simulink model "simulator_prototype_v2"  (R2021b)
(part 8 of 12)

tau_c = ft_11({dq1,dq2,dq3,dq4,dq5,dq6,t10,t1005,t1022,t1089,t11,t1104,t1105,t1108,t1115,t1121,t1158,t1159,t1196,t12,t1205,t1207,t1208,t1210,t1212,t1217,t1218,t1221,t123,t1230,t1235,t1237,t1238,t1288,t1289,t13,t1302,t1303,t1319,t1320,t1336,t1348,t1350,t1351,t1360,t1369,t1378,t1396,t14,t140,t1425,t1435,t1456,t1477,t1488,t15,t1513,t1539,t1544,t1547,t1548,t1553,t1554,t1559,t1564,t1576,t1577,t1578,t1579,t1584,t1585,t1586,t1587,t1591,t1599,t16,t1600,t1602,t1604,t1605,t1606,t1607,t1608,t1609,t1613,t1614,t1615,t1616,t1626,t1627,t1628,t1629,t1631,t1637,t1640,t1641,t1648,t1649,t1659,t1660,t1661,t1666,t1667,t1683,t1686,t1690,t1692,t17,t1700,t1701,t1704,t1705,t1712,t1717,t1738,t1741,t1742,t1750,t1752,t1753,t1754,t1758,t1759,t1775,t1776,t18,t1861,t1874,t1879,t188,t1881,t189,t1896,t19,t1901,t1941,t1959,t1973,t1993,t1994,t20,t201,t202,t2023,t2053,t2060,t2089,t2090,t2098,t2099,t21,t2117,t2120,t2122,t2123,t2125,t2137,t2139,t2140,t2142,t2147,t2149,t2150,t2151,t2152,t2154,t2155,t2159,t2164,t2165,t2166,t2167,t2168,t2174,t2183,t2187,t2193,t2194,t2195,t2199,t22,t2203,t2215,t2219,t2222,t2223,t2239,t2240,t2256,t2257,t2291,t2292,t2293,t2294,t2295,t2297,t2298,t2299,t2301,t2302,t2303,t2304,t2306,t2307,t2308,t2311,t2317,t2320,t2323,t2325,t2326,t2329,t2337,t2338,t2339,t2341,t2343,t2344,t2352,t2353,t2355,t2359,t236,t2360,t2361,t2362,t2363,t2364,t2365,t2366,t2367,t2368,t2369,t237,t2370,t2371,t2378,t2379,t238,t2380,t2384,t2388,t2389,t2391,t2394,t2395,t2397,t2398,t2399,t24,t2400,t2401,t2403,t2404,t2405,t241,t2414,t2419,t2421,t2423,t2438,t2448,t2449,t2461,t2471,t2472,t2492,t2493,t2494,t25,t2502,t2510,t2519,t2527,t2530,t2534,t2555,t2556,t2572,t2575,t2583,t2598,t26,t2605,t2606,t2612,t2613,t2618,t2619,t262,t2638,t264,t2651,t2652,t2670,t2671,t2673,t2674,t2675,t2676,t2678,t2680,t2683,t2684,t2685,t2686,t2687,t2689,t2690,t2692,t2693,t2694,t2695,t2696,t2697,t2698,t27,t2700,t2701,t2704,t2705,t2707,t2708,t2709,t2711,t2712,t2713,t2715,t2716,t2717,t2719,t2720,t2721,t2736,t2740,t2744,t2745,t2747,t2748,t2749,t2750,t2754,t2759,t2773,t2774,t2777,t2778,t2779,t2781,t2785,t2786,t2787,t2788,t2797,t28,t2801,t2804,t2813,t2814,t2820,t2831,t2834,t2835,t2838,t2850,t2851,t29,t2937,t2942,t2945,t2946,t2950,t2951,t2953,t2954,t2955,t2956,t2957,t2965,t2966,t2975,t2978,t2979,t2984,t2987,t2990,t2991,t2993,t2994,t2998,t30,t3003,t3004,t3008,t3009,t3015,t3017,t3022,t3027,t3029,t3030,t3036,t3043,t3044,t3045,t3047,t3049,t3050,t3051,t3054,t3055,t3057,t3058,t3063,t3064,t3066,t3067,t3068,t3072,t3073,t3079,t3080,t3081,t3085,t3086,t3087,t3088,t3096,t3097,t31,t3109,t3117,t3118,t3121,t3122,t3126,t3129,t313,t3130,t3131,t3132,t3133,t3134,t3135,t3136,t314,t3140,t3141,t3142,t3143,t3145,t3148,t3150,t3153,t3154,t3156,t3157,t3158,t3159,t3160,t3161,t3162,t3163,t3164,t3165,t3167,t3171,t3172,t3173,t3180,t3181,t3185,t3187,t3188,t3189,t3190,t3192,t3193,t3194,t3195,t3196,t3198,t3199,t32,t3200,t3201,t3202,t3203,t3205,t3206,t3208,t3209,t321,t3211,t3213,t3216,t3217,t3219,t3221,t3225,t3230,t3231,t3232,t3233,t3234,t3235,t3236,t3237,t3238,t3239,t3242,t3252,t3253,t3254,t3256,t3257,t3259,t326,t3260,t3261,t3263,t3265,t3266,t3267,t3268,t3269,t3270,t3271,t3272,t3273,t3276,t3277,t3278,t3279,t328,t3282,t3283,t3284,t3287,t3288,t329,t3290,t3291,t3294,t3297,t3298,t3299,t33,t3300,t3302,t3303,t3304,t3305,t3307,t3309,t331,t3310,t3312,t3313,t3314,t3315,t3316,t3318,t332,t3322,t3324,t3326,t3328,t3329,t333,t3332,t3333,t3334,t3335,t3336,t3337,t3338,t3340,t3341,t3343,t3344,t3345,t3346,t3347,t3348,t335,t3350,t3351,t3352,t3353,t3354,t3355,t3357,t3358,t3359,t3361,t3363,t3364,t3365,t3367,t3368,t3369,t3370,t3377,t3379,t338,t3383,t3386,t3387,t3389,t339,t3392,t3394,t3395,t3396,t3399,t34,t3402,t3405,t3409,t3415,t3416,t3419,t3420,t3421,t3423,t3426,t3428,t3430,t3431,t3432,t3433,t3434,t3435,t3438,t3439,t3440,t3441,t3443,t3444,t3445,t3446,t3447,t3448,t3449,t3451,t3452,t3453,t3454,t3455,t3456,t3457,t3458,t346,t3460,t3461,t3462,t3463,t3465,t3467,t3468,t3469,t3470,t3471,t3474,t3480,t3482,t3483,t3488,t3489,t3490,t3492,t3495,t3496,t3498,t3499,t35,t350,t3500,t3502,t3503,t3508,t351,t3510,t3512,t3517,t3519,t3522,t3524,t3527,t3528,t3529,t3531,t3532,t3534,t3537,t354,t3541,t3543,t3545,t3546,t3547,t3549,t3550,t3551,t3552,t3554,t3558,t356,t3561,t3562,t3563,t3566,t3568,t3569,t3577,t3578,t358,t3580,t3581,t3582,t3583,t3584,t3586,t3588,t3589,t359,t3590,t3591,t3592,t3593,t3594,t3597,t3598,t3599,t36,t360,t3600,t3601,t3602,t3603,t3605,t3606,t3607,t3608,t3609,t3610,t3611,t3612,t3614,t3616,t3617,t3618,t3619,t362,t3621,t3624,t3626,t3628,t363,t3630,t3631,t3632,t3633,t3634,t3635,t3636,t3637,t3638,t3639,t364,t3640,t3641,t3642,t3643,t3644,t3645,t3646,t3647,t3648,t3649,t365,t3650,t3651,t3652,t3653,t3654,t3655,t3656,t3657,t3658,t3659,t366,t3660,t3661,t3662,t3664,t3666,t3667,t3668,t3669,t3670,t3671,t3672,t3673,t3674,t3675,t3677,t3678,t3679,t3680,t3681,t3683,t3684,t3688,t3689,t3690,t3692,t3693,t3695,t3696,t3697,t3699,t3700,t3701,t3702,t3703,t3704,t3705,t3706,t3707,t3708,t3709,t371,t3710,t3711,t3712,t3713,t3716,t3717,t3719,t372,t3721,t3722,t3723,t3726,t3728,t3729,t3731,t3732,t3734,t3735,t3736,t3737,t3738,t3739,t3741,t3743,t3746,t3747,t3749,t3751,t3752,t3753,t3754,t3755,t3759,t3760,t3764,t3765,t3766,t3770,t3771,t3772,t3774,t3775,t3777,t3779,t378,t3781,t3782,t3783,t3784,t3785,t3786,t3788,t3789,t3790,t3791,t3792,t3793,t3794,t3795,t3796,t3797,t3798,t38,t380,t3800,t3801,t3802,t3804,t3805,t3808,t3809,t3810,t3814,t3815,t3817,t3818,t3819,t382,t3820,t3821,t3823,t3824,t3826,t3827,t3828,t3830,t3832,t3833,t3834,t3835,t3840,t3843,t3844,t3845,t3846,t3848,t3850,t3851,t3855,t3856,t3857,t3859,t3862,t3863,t3866,t3867,t387,t3870,t3873,t3874,t3876,t3877,t3878,t3879,t3880,t3885,t3888,t3889,t3890,t3891,t3893,t3895,t3896,t3897,t3898,t39,t3900,t3901,t3902,t3903,t3906,t3908,t3909,t3910,t3913,t3915,t3919,t3924,t3925,t3926,t3931,t3934,t3937,t3939,t3941,t3943,t3949,t3951,t3953,t3954,t3957,t3958,t3959,t3961,t3966,t3967,t3968,t3970,t3971,t3973,t3974,t3975,t3976,t3977,t3979,t3980,t3983,t3985,t3987,t3988,t3991,t3992,t3993,t3996,t3997,t3998,t3999,t4001,t4002,t4008,t4010,t4011,t4012,t4014,t4015,t4016,t4017,t4018,t4019,t4026,t4030,t4031,t4032,t4035,t4038,t4039,t4041,t4045,t4046,t4047,t4048,t4049,t4050,t4059,t4060,t4063,t4064,t4065,t4066,t4071,t4086,t4090,t4091,t4092,t4096,t4097,t4098,t4099,t410,t4100,t4101,t4103,t4105,t4107,t4108,t4109,t4110,t4111,t4112,t4116,t4117,t4118,t4121,t4122,t4144,t4146,t4147,t4149,t4151,t4153,t4154,t4156,t4157,t4158,t4159,t4160,t4163,t4165,t4171,t4172,t4179,t4180,t4187,t4188,t4189,t4190,t4193,t4195,t4198,t42,t4200,t4201,t4204,t4205,t4207,t4208,t4210,t4213,t4215,t4218,t4219,t4224,t4229,t4230,t4236,t4237,t4240,t4241,t4243,t4244,t4246,t4248,t4249,t4258,t4260,t4261,t4263,t4265,t4270,t4272,t4273,t4274,t4275,t4276,t4277,t4278,t4279,t4280,t4281,t4282,t4283,t4286,t4287,t4288,t4289,t429,t4290,t4291,t4293,t4294,t4295,t4296,t4297,t4298,t4299,t43,t4300,t4301,t4303,t4304,t4305,t4306,t4307,t4308,t4310,t4311,t4312,t4313,t4314,t4318,t4319,t4320,t4322,t4323,t4324,t4325,t4326,t4330,t4331,t4332,t4333,t4334,t4337,t4339,t4341,t4342,t4343,t4344,t4345,t4346,t4347,t4352,t4354,t4355,t4356,t4358,t4359,t4361,t4362,t4371,t4372,t4373,t4374,t4375,t4376,t4403,t4404,t4405,t4406,t4407,t4409,t4413,t4415,t4416,t4417,t4420,t4422,t4423,t4426,t4427,t4428,t4429,t4430,t4431,t4432,t4434,t4435,t4436,t4438,t4439,t4440,t4441,t4443,t4448,t4449,t4455,t4456,t4457,t4458,t4459,t4461,t4462,t4464,t4465,t4466,t4467,t4468,t4470,t4476,t4479,t4482,t4485,t4486,t4487,t4488,t4489,t4491,t4492,t4493,t4494,t4495,t4496,t4497,t4498,t4499,t4500,t4501,t4502,t4504,t4510,t4515,t4517,t4518,t4520,t4522,t4523,t4529,t4532,t4533,t4534,t4537,t4541,t4542,t4544,t4545,t4546,t4548,t4549,t4550,t4551,t4553,t4554,t4559,t4561,t4562,t4563,t4564,t4565,t4567,t4570,t4571,t4573,t4574,t4576,t4577,t4578,t4579,t4580,t4583,t4584,t4585,t4588,t4589,t4591,t4593,t4594,t4595,t4596,t4598,t4599,t46,t4602,t4605,t4606,t4608,t4609,t4612,t4613,t4614,t4615,t4618,t4623,t4625,t4626,t4634,t4635,t4637,t4643,t4644,t4645,t4646,t4647,t4648,t4649,t4650,t4651,t4652,t4654,t4656,t4657,t4658,t4660,t4663,t4665,t4667,t4669,t4670,t4672,t4673,t4674,t4675,t4676,t4677,t4678,t4680,t4681,t4682,t4683,t4684,t4685,t4686,t4687,t4690,t4691,t4692,t4694,t4696,t47,t4703,t4704,t4705,t4708,t4709,t4711,t4712,t4713,t4716,t4718,t4719,t4722,t4724,t4725,t4726,t4727,t4728,t4730,t4731,t4733,t4734,t4737,t4739,t4741,t4742,t4743,t4744,t4746,t4751,t4757,t4760,t4761,t4762,t4763,t4764,t4766,t4767,t4768,t4769,t4774,t4776,t4777,t4778,t4779,t4781,t4783,t4784,t4785,t4786,t4787,t4790,t4791,t4792,t4793,t4794,t4795,t4796,t4798,t4799,t4801,t4803,t4806,t4812,t4814,t4815,t4816,t4818,t4820,t4824,t4825,t4826,t4828,t4833,t4835,t4838,t4843,t4844,t4845,t4846,t4847,t4848,t4849,t4850,t4853,t4856,t4857,t4858,t4859,t4863,t4867,t4872,t4874,t4875,t4876,t4879,t4880,t4883,t4886,t4887,t4889,t4892,t4893,t4895,t4896,t4898,t4899,t4901,t4902,t4904,t4907,t4911,t4912,t4915,t4918,t4919,t4920,t4921,t4922,t4923,t4924,t4925,t4926,t4927,t4928,t4929,t4930,t4933,t4934,t4935,t4936,t4937,t4938,t4939,t4940,t4941,t4943,t4945,t4946,t4947,t4950,t4952,t4953,t4955,t4958,t4969,t4973,t4974,t4977,t4979,t50,t5001,t5003,t5004,t5005,t5012,t5013,t5014,t5016,t5019,t5020,t5024,t5025,t5026,t5027,t5028,t5033,t5034,t5035,t5036,t5037,t5038,t5041,t5042,t5043,t5045,t5046,t5047,t5049,t5051,t5052,t5053,t5059,t5061,t5062,t5063,t5064,t5066,t5070,t5071,t5072,t5074,t5075,t5076,t5077,t5079,t5080,t5081,t5082,t5083,t5084,t5085,t5086,t5087,t5088,t5089,t5090,t5091,t5093,t5096,t5097,t5098,t5100,t5101,t5103,t5106,t5108,t5111,t5113,t5114,t5117,t5118,t5119,t5123,t5124,t5126,t5127,t5141,t5142,t5144,t5146,t5155,t5158,t5161,t5163,t5164,t5165,t5166,t5168,t5169,t5171,t5173,t5174,t5176,t5177,t5178,t5180,t5181,t5194,t5195,t5196,t5197,t5198,t5199,t5200,t5201,t5202,t5203,t5205,t5208,t5212,t5213,t5214,t5215,t5219,t5234,t5240,t5241,t5243,t5244,t5246,t5247,t5248,t5249,t5251,t5254,t5255,t5256,t5257,t5258,t5259,t5261,t5262,t5263,t5264,t5265,t5266,t5267,t5268,t5269,t5271,t5272,t5273,t5274,t5276,t5277,t5278,t5279,t5280,t5281,t5283,t5284,t5285,t5286,t5287,t5288,t5289,t5290,t5291,t5292,t5293,t5294,t5295,t5296,t5297,t5298,t5300,t5301,t5302,t5303,t5304,t5305,t5306,t5308,t5309,t5310,t5312,t5315,t5316,t5318,t5320,t5321,t5322,t5324,t5325,t5327,t5328,t5329,t5330,t5331,t5332,t5336,t5337,t5340,t5343,t5344,t5345,t5346,t5348,t5350,t5352,t5353,t5354,t5356,t5357,t5358,t5359,t5361,t5362,t5363,t5370,t5372,t5374,t5378,t5381,t5383,t5384,t5387,t5389,t5391,t5392,t5393,t5395,t5399,t5400,t5401,t5402,t5403,t5404,t5410,t5411,t5412,t5415,t5416,t5419,t5424,t5425,t5433,t5434,t5436,t5437,t5438,t5439,t5440,t5441,t5442,t5443,t5444,t5445,t5446,t5448,t5449,t5452,t5456,t5457,t5458,t5459,t5460,t5461,t5462,t5464,t5465,t5472,t5474,t5481,t5487,t5488,t5494,t5495,t5499,t5500,t5501,t5503,t5504,t5506,t5507,t5509,t5510,t5512,t5513,t5514,t5516,t5517,t5520,t5522,t5523,t5524,t5535,t5536,t5537,t5538,t5539,t5540,t5541,t5542,t5543,t5544,t5545,t5548,t5549,t5550,t5555,t5556,t5560,t5561,t5565,t5567,t5568,t5569,t5570,t5575,t5576,t5577,t5578,t5586,t5590,t5591,t5592,t5595,t5599,t56,t5602,t5604,t5605,t5607,t5608,t5609,t5611,t5612,t5620,t5624,t5627,t5653,t5658,t5660,t5662,t5677,t5678,t5684,t5698,t5699,t5705,t5719,t5721,t5722,t5730,t5731,t5734,t5735,t5737,t5738,t5739,t5741,t5742,t5744,t5757,t5758,t5759,t5760,t5761,t5768,t5775,t5777,t5779,t5781,t5782,t5783,t5784,t5788,t58,t5813,t5818,t5825,t5849,t5852,t5891,t5892,t5896,t59,t5901,t5902,t5908,t5909,t5916,t5917,t5922,t5924,t5925,t5928,t5933,t5938,t5941,t5954,t5955,t5966,t5971,t5990,t60,t6002,t6004,t6005,t6011,t6013,t6014,t6048,t6050,t6051,t6062,t6074,t6075,t6078,t6123,t6125,t6132,t6143,t6166,t6211,t6221,t6222,t6255,t6256,t6257,t6271,t628,t638,t6394,t6396,t6398,t640,t642,t643,t6442,t6482,t649,t6523,t654,t655,t656,t6564,t6565,t657,t6574,t6588,t6589,t659,t660,t6622,t6623,t665,t6651,t667,t668,t669,t67,t670,t672,t673,t674,t6745,t675,t6751,t676,t677,t68,t681,t682,t684,t685,t686,t687,t691,t6919,t692,t6920,t693,t694,t6966,t6987,t70,t7005,t702,t707,t708,t7088,t7089,t71,t710,t7138,t7148,t715,t7150,t7152,t716,t7160,t717,t7172,t718,t721,t722,t724,t725,t73,t7304,t7319,t7331,t7332,t7333,t7334,t736,t738,t740,t741,t749,t756,t76,t762,t768,t777,t792,t793,t8,t801,t802,t808,t813,t819,t821,t850,t855,t874,t878,t89,t9,t90,t91,t92,t941,t944,t948,t951,t97});
end
function tau_c = ft_11(ct)
dq1 = ct{1};
dq2 = ct{2};
dq3 = ct{3};
dq4 = ct{4};
dq5 = ct{5};
dq6 = ct{6};
t10 = ct{7};
t1005 = ct{8};
t1022 = ct{9};
t1089 = ct{10};
t11 = ct{11};
t1104 = ct{12};
t1105 = ct{13};
t1108 = ct{14};
t1115 = ct{15};
t1121 = ct{16};
t1158 = ct{17};
t1159 = ct{18};
t1196 = ct{19};
t12 = ct{20};
t1205 = ct{21};
t1207 = ct{22};
t1208 = ct{23};
t1210 = ct{24};
t1212 = ct{25};
t1217 = ct{26};
t1218 = ct{27};
t1221 = ct{28};
t123 = ct{29};
t1230 = ct{30};
t1235 = ct{31};
t1237 = ct{32};
t1238 = ct{33};
t1288 = ct{34};
t1289 = ct{35};
t13 = ct{36};
t1302 = ct{37};
t1303 = ct{38};
t1319 = ct{39};
t1320 = ct{40};
t1336 = ct{41};
t1348 = ct{42};
t1350 = ct{43};
t1351 = ct{44};
t1360 = ct{45};
t1369 = ct{46};
t1378 = ct{47};
t1396 = ct{48};
t14 = ct{49};
t140 = ct{50};
t1425 = ct{51};
t1435 = ct{52};
t1456 = ct{53};
t1477 = ct{54};
t1488 = ct{55};
t15 = ct{56};
t1513 = ct{57};
t1539 = ct{58};
t1544 = ct{59};
t1547 = ct{60};
t1548 = ct{61};
t1553 = ct{62};
t1554 = ct{63};
t1559 = ct{64};
t1564 = ct{65};
t1576 = ct{66};
t1577 = ct{67};
t1578 = ct{68};
t1579 = ct{69};
t1584 = ct{70};
t1585 = ct{71};
t1586 = ct{72};
t1587 = ct{73};
t1591 = ct{74};
t1599 = ct{75};
t16 = ct{76};
t1600 = ct{77};
t1602 = ct{78};
t1604 = ct{79};
t1605 = ct{80};
t1606 = ct{81};
t1607 = ct{82};
t1608 = ct{83};
t1609 = ct{84};
t1613 = ct{85};
t1614 = ct{86};
t1615 = ct{87};
t1616 = ct{88};
t1626 = ct{89};
t1627 = ct{90};
t1628 = ct{91};
t1629 = ct{92};
t1631 = ct{93};
t1637 = ct{94};
t1640 = ct{95};
t1641 = ct{96};
t1648 = ct{97};
t1649 = ct{98};
t1659 = ct{99};
t1660 = ct{100};
t1661 = ct{101};
t1666 = ct{102};
t1667 = ct{103};
t1683 = ct{104};
t1686 = ct{105};
t1690 = ct{106};
t1692 = ct{107};
t17 = ct{108};
t1700 = ct{109};
t1701 = ct{110};
t1704 = ct{111};
t1705 = ct{112};
t1712 = ct{113};
t1717 = ct{114};
t1738 = ct{115};
t1741 = ct{116};
t1742 = ct{117};
t1750 = ct{118};
t1752 = ct{119};
t1753 = ct{120};
t1754 = ct{121};
t1758 = ct{122};
t1759 = ct{123};
t1775 = ct{124};
t1776 = ct{125};
t18 = ct{126};
t1861 = ct{127};
t1874 = ct{128};
t1879 = ct{129};
t188 = ct{130};
t1881 = ct{131};
t189 = ct{132};
t1896 = ct{133};
t19 = ct{134};
t1901 = ct{135};
t1941 = ct{136};
t1959 = ct{137};
t1973 = ct{138};
t1993 = ct{139};
t1994 = ct{140};
t20 = ct{141};
t201 = ct{142};
t202 = ct{143};
t2023 = ct{144};
t2053 = ct{145};
t2060 = ct{146};
t2089 = ct{147};
t2090 = ct{148};
t2098 = ct{149};
t2099 = ct{150};
t21 = ct{151};
t2117 = ct{152};
t2120 = ct{153};
t2122 = ct{154};
t2123 = ct{155};
t2125 = ct{156};
t2137 = ct{157};
t2139 = ct{158};
t2140 = ct{159};
t2142 = ct{160};
t2147 = ct{161};
t2149 = ct{162};
t2150 = ct{163};
t2151 = ct{164};
t2152 = ct{165};
t2154 = ct{166};
t2155 = ct{167};
t2159 = ct{168};
t2164 = ct{169};
t2165 = ct{170};
t2166 = ct{171};
t2167 = ct{172};
t2168 = ct{173};
t2174 = ct{174};
t2183 = ct{175};
t2187 = ct{176};
t2193 = ct{177};
t2194 = ct{178};
t2195 = ct{179};
t2199 = ct{180};
t22 = ct{181};
t2203 = ct{182};
t2215 = ct{183};
t2219 = ct{184};
t2222 = ct{185};
t2223 = ct{186};
t2239 = ct{187};
t2240 = ct{188};
t2256 = ct{189};
t2257 = ct{190};
t2291 = ct{191};
t2292 = ct{192};
t2293 = ct{193};
t2294 = ct{194};
t2295 = ct{195};
t2297 = ct{196};
t2298 = ct{197};
t2299 = ct{198};
t2301 = ct{199};
t2302 = ct{200};
t2303 = ct{201};
t2304 = ct{202};
t2306 = ct{203};
t2307 = ct{204};
t2308 = ct{205};
t2311 = ct{206};
t2317 = ct{207};
t2320 = ct{208};
t2323 = ct{209};
t2325 = ct{210};
t2326 = ct{211};
t2329 = ct{212};
t2337 = ct{213};
t2338 = ct{214};
t2339 = ct{215};
t2341 = ct{216};
t2343 = ct{217};
t2344 = ct{218};
t2352 = ct{219};
t2353 = ct{220};
t2355 = ct{221};
t2359 = ct{222};
t236 = ct{223};
t2360 = ct{224};
t2361 = ct{225};
t2362 = ct{226};
t2363 = ct{227};
t2364 = ct{228};
t2365 = ct{229};
t2366 = ct{230};
t2367 = ct{231};
t2368 = ct{232};
t2369 = ct{233};
t237 = ct{234};
t2370 = ct{235};
t2371 = ct{236};
t2378 = ct{237};
t2379 = ct{238};
t238 = ct{239};
t2380 = ct{240};
t2384 = ct{241};
t2388 = ct{242};
t2389 = ct{243};
t2391 = ct{244};
t2394 = ct{245};
t2395 = ct{246};
t2397 = ct{247};
t2398 = ct{248};
t2399 = ct{249};
t24 = ct{250};
t2400 = ct{251};
t2401 = ct{252};
t2403 = ct{253};
t2404 = ct{254};
t2405 = ct{255};
t241 = ct{256};
t2414 = ct{257};
t2419 = ct{258};
t2421 = ct{259};
t2423 = ct{260};
t2438 = ct{261};
t2448 = ct{262};
t2449 = ct{263};
t2461 = ct{264};
t2471 = ct{265};
t2472 = ct{266};
t2492 = ct{267};
t2493 = ct{268};
t2494 = ct{269};
t25 = ct{270};
t2502 = ct{271};
t2510 = ct{272};
t2519 = ct{273};
t2527 = ct{274};
t2530 = ct{275};
t2534 = ct{276};
t2555 = ct{277};
t2556 = ct{278};
t2572 = ct{279};
t2575 = ct{280};
t2583 = ct{281};
t2598 = ct{282};
t26 = ct{283};
t2605 = ct{284};
t2606 = ct{285};
t2612 = ct{286};
t2613 = ct{287};
t2618 = ct{288};
t2619 = ct{289};
t262 = ct{290};
t2638 = ct{291};
t264 = ct{292};
t2651 = ct{293};
t2652 = ct{294};
t2670 = ct{295};
t2671 = ct{296};
t2673 = ct{297};
t2674 = ct{298};
t2675 = ct{299};
t2676 = ct{300};
t2678 = ct{301};
t2680 = ct{302};
t2683 = ct{303};
t2684 = ct{304};
t2685 = ct{305};
t2686 = ct{306};
t2687 = ct{307};
t2689 = ct{308};
t2690 = ct{309};
t2692 = ct{310};
t2693 = ct{311};
t2694 = ct{312};
t2695 = ct{313};
t2696 = ct{314};
t2697 = ct{315};
t2698 = ct{316};
t27 = ct{317};
t2700 = ct{318};
t2701 = ct{319};
t2704 = ct{320};
t2705 = ct{321};
t2707 = ct{322};
t2708 = ct{323};
t2709 = ct{324};
t2711 = ct{325};
t2712 = ct{326};
t2713 = ct{327};
t2715 = ct{328};
t2716 = ct{329};
t2717 = ct{330};
t2719 = ct{331};
t2720 = ct{332};
t2721 = ct{333};
t2736 = ct{334};
t2740 = ct{335};
t2744 = ct{336};
t2745 = ct{337};
t2747 = ct{338};
t2748 = ct{339};
t2749 = ct{340};
t2750 = ct{341};
t2754 = ct{342};
t2759 = ct{343};
t2773 = ct{344};
t2774 = ct{345};
t2777 = ct{346};
t2778 = ct{347};
t2779 = ct{348};
t2781 = ct{349};
t2785 = ct{350};
t2786 = ct{351};
t2787 = ct{352};
t2788 = ct{353};
t2797 = ct{354};
t28 = ct{355};
t2801 = ct{356};
t2804 = ct{357};
t2813 = ct{358};
t2814 = ct{359};
t2820 = ct{360};
t2831 = ct{361};
t2834 = ct{362};
t2835 = ct{363};
t2838 = ct{364};
t2850 = ct{365};
t2851 = ct{366};
t29 = ct{367};
t2937 = ct{368};
t2942 = ct{369};
t2945 = ct{370};
t2946 = ct{371};
t2950 = ct{372};
t2951 = ct{373};
t2953 = ct{374};
t2954 = ct{375};
t2955 = ct{376};
t2956 = ct{377};
t2957 = ct{378};
t2965 = ct{379};
t2966 = ct{380};
t2975 = ct{381};
t2978 = ct{382};
t2979 = ct{383};
t2984 = ct{384};
t2987 = ct{385};
t2990 = ct{386};
t2991 = ct{387};
t2993 = ct{388};
t2994 = ct{389};
t2998 = ct{390};
t30 = ct{391};
t3003 = ct{392};
t3004 = ct{393};
t3008 = ct{394};
t3009 = ct{395};
t3015 = ct{396};
t3017 = ct{397};
t3022 = ct{398};
t3027 = ct{399};
t3029 = ct{400};
t3030 = ct{401};
t3036 = ct{402};
t3043 = ct{403};
t3044 = ct{404};
t3045 = ct{405};
t3047 = ct{406};
t3049 = ct{407};
t3050 = ct{408};
t3051 = ct{409};
t3054 = ct{410};
t3055 = ct{411};
t3057 = ct{412};
t3058 = ct{413};
t3063 = ct{414};
t3064 = ct{415};
t3066 = ct{416};
t3067 = ct{417};
t3068 = ct{418};
t3072 = ct{419};
t3073 = ct{420};
t3079 = ct{421};
t3080 = ct{422};
t3081 = ct{423};
t3085 = ct{424};
t3086 = ct{425};
t3087 = ct{426};
t3088 = ct{427};
t3096 = ct{428};
t3097 = ct{429};
t31 = ct{430};
t3109 = ct{431};
t3117 = ct{432};
t3118 = ct{433};
t3121 = ct{434};
t3122 = ct{435};
t3126 = ct{436};
t3129 = ct{437};
t313 = ct{438};
t3130 = ct{439};
t3131 = ct{440};
t3132 = ct{441};
t3133 = ct{442};
t3134 = ct{443};
t3135 = ct{444};
t3136 = ct{445};
t314 = ct{446};
t3140 = ct{447};
t3141 = ct{448};
t3142 = ct{449};
t3143 = ct{450};
t3145 = ct{451};
t3148 = ct{452};
t3150 = ct{453};
t3153 = ct{454};
t3154 = ct{455};
t3156 = ct{456};
t3157 = ct{457};
t3158 = ct{458};
t3159 = ct{459};
t3160 = ct{460};
t3161 = ct{461};
t3162 = ct{462};
t3163 = ct{463};
t3164 = ct{464};
t3165 = ct{465};
t3167 = ct{466};
t3171 = ct{467};
t3172 = ct{468};
t3173 = ct{469};
t3180 = ct{470};
t3181 = ct{471};
t3185 = ct{472};
t3187 = ct{473};
t3188 = ct{474};
t3189 = ct{475};
t3190 = ct{476};
t3192 = ct{477};
t3193 = ct{478};
t3194 = ct{479};
t3195 = ct{480};
t3196 = ct{481};
t3198 = ct{482};
t3199 = ct{483};
t32 = ct{484};
t3200 = ct{485};
t3201 = ct{486};
t3202 = ct{487};
t3203 = ct{488};
t3205 = ct{489};
t3206 = ct{490};
t3208 = ct{491};
t3209 = ct{492};
t321 = ct{493};
t3211 = ct{494};
t3213 = ct{495};
t3216 = ct{496};
t3217 = ct{497};
t3219 = ct{498};
t3221 = ct{499};
t3225 = ct{500};
t3230 = ct{501};
t3231 = ct{502};
t3232 = ct{503};
t3233 = ct{504};
t3234 = ct{505};
t3235 = ct{506};
t3236 = ct{507};
t3237 = ct{508};
t3238 = ct{509};
t3239 = ct{510};
t3242 = ct{511};
t3252 = ct{512};
t3253 = ct{513};
t3254 = ct{514};
t3256 = ct{515};
t3257 = ct{516};
t3259 = ct{517};
t326 = ct{518};
t3260 = ct{519};
t3261 = ct{520};
t3263 = ct{521};
t3265 = ct{522};
t3266 = ct{523};
t3267 = ct{524};
t3268 = ct{525};
t3269 = ct{526};
t3270 = ct{527};
t3271 = ct{528};
t3272 = ct{529};
t3273 = ct{530};
t3276 = ct{531};
t3277 = ct{532};
t3278 = ct{533};
t3279 = ct{534};
t328 = ct{535};
t3282 = ct{536};
t3283 = ct{537};
t3284 = ct{538};
t3287 = ct{539};
t3288 = ct{540};
t329 = ct{541};
t3290 = ct{542};
t3291 = ct{543};
t3294 = ct{544};
t3297 = ct{545};
t3298 = ct{546};
t3299 = ct{547};
t33 = ct{548};
t3300 = ct{549};
t3302 = ct{550};
t3303 = ct{551};
t3304 = ct{552};
t3305 = ct{553};
t3307 = ct{554};
t3309 = ct{555};
t331 = ct{556};
t3310 = ct{557};
t3312 = ct{558};
t3313 = ct{559};
t3314 = ct{560};
t3315 = ct{561};
t3316 = ct{562};
t3318 = ct{563};
t332 = ct{564};
t3322 = ct{565};
t3324 = ct{566};
t3326 = ct{567};
t3328 = ct{568};
t3329 = ct{569};
t333 = ct{570};
t3332 = ct{571};
t3333 = ct{572};
t3334 = ct{573};
t3335 = ct{574};
t3336 = ct{575};
t3337 = ct{576};
t3338 = ct{577};
t3340 = ct{578};
t3341 = ct{579};
t3343 = ct{580};
t3344 = ct{581};
t3345 = ct{582};
t3346 = ct{583};
t3347 = ct{584};
t3348 = ct{585};
t335 = ct{586};
t3350 = ct{587};
t3351 = ct{588};
t3352 = ct{589};
t3353 = ct{590};
t3354 = ct{591};
t3355 = ct{592};
t3357 = ct{593};
t3358 = ct{594};
t3359 = ct{595};
t3361 = ct{596};
t3363 = ct{597};
t3364 = ct{598};
t3365 = ct{599};
t3367 = ct{600};
t3368 = ct{601};
t3369 = ct{602};
t3370 = ct{603};
t3377 = ct{604};
t3379 = ct{605};
t338 = ct{606};
t3383 = ct{607};
t3386 = ct{608};
t3387 = ct{609};
t3389 = ct{610};
t339 = ct{611};
t3392 = ct{612};
t3394 = ct{613};
t3395 = ct{614};
t3396 = ct{615};
t3399 = ct{616};
t34 = ct{617};
t3402 = ct{618};
t3405 = ct{619};
t3409 = ct{620};
t3415 = ct{621};
t3416 = ct{622};
t3419 = ct{623};
t3420 = ct{624};
t3421 = ct{625};
t3423 = ct{626};
t3426 = ct{627};
t3428 = ct{628};
t3430 = ct{629};
t3431 = ct{630};
t3432 = ct{631};
t3433 = ct{632};
t3434 = ct{633};
t3435 = ct{634};
t3438 = ct{635};
t3439 = ct{636};
t3440 = ct{637};
t3441 = ct{638};
t3443 = ct{639};
t3444 = ct{640};
t3445 = ct{641};
t3446 = ct{642};
t3447 = ct{643};
t3448 = ct{644};
t3449 = ct{645};
t3451 = ct{646};
t3452 = ct{647};
t3453 = ct{648};
t3454 = ct{649};
t3455 = ct{650};
t3456 = ct{651};
t3457 = ct{652};
t3458 = ct{653};
t346 = ct{654};
t3460 = ct{655};
t3461 = ct{656};
t3462 = ct{657};
t3463 = ct{658};
t3465 = ct{659};
t3467 = ct{660};
t3468 = ct{661};
t3469 = ct{662};
t3470 = ct{663};
t3471 = ct{664};
t3474 = ct{665};
t3480 = ct{666};
t3482 = ct{667};
t3483 = ct{668};
t3488 = ct{669};
t3489 = ct{670};
t3490 = ct{671};
t3492 = ct{672};
t3495 = ct{673};
t3496 = ct{674};
t3498 = ct{675};
t3499 = ct{676};
t35 = ct{677};
t350 = ct{678};
t3500 = ct{679};
t3502 = ct{680};
t3503 = ct{681};
t3508 = ct{682};
t351 = ct{683};
t3510 = ct{684};
t3512 = ct{685};
t3517 = ct{686};
t3519 = ct{687};
t3522 = ct{688};
t3524 = ct{689};
t3527 = ct{690};
t3528 = ct{691};
t3529 = ct{692};
t3531 = ct{693};
t3532 = ct{694};
t3534 = ct{695};
t3537 = ct{696};
t354 = ct{697};
t3541 = ct{698};
t3543 = ct{699};
t3545 = ct{700};
t3546 = ct{701};
t3547 = ct{702};
t3549 = ct{703};
t3550 = ct{704};
t3551 = ct{705};
t3552 = ct{706};
t3554 = ct{707};
t3558 = ct{708};
t356 = ct{709};
t3561 = ct{710};
t3562 = ct{711};
t3563 = ct{712};
t3566 = ct{713};
t3568 = ct{714};
t3569 = ct{715};
t3577 = ct{716};
t3578 = ct{717};
t358 = ct{718};
t3580 = ct{719};
t3581 = ct{720};
t3582 = ct{721};
t3583 = ct{722};
t3584 = ct{723};
t3586 = ct{724};
t3588 = ct{725};
t3589 = ct{726};
t359 = ct{727};
t3590 = ct{728};
t3591 = ct{729};
t3592 = ct{730};
t3593 = ct{731};
t3594 = ct{732};
t3597 = ct{733};
t3598 = ct{734};
t3599 = ct{735};
t36 = ct{736};
t360 = ct{737};
t3600 = ct{738};
t3601 = ct{739};
t3602 = ct{740};
t3603 = ct{741};
t3605 = ct{742};
t3606 = ct{743};
t3607 = ct{744};
t3608 = ct{745};
t3609 = ct{746};
t3610 = ct{747};
t3611 = ct{748};
t3612 = ct{749};
t3614 = ct{750};
t3616 = ct{751};
t3617 = ct{752};
t3618 = ct{753};
t3619 = ct{754};
t362 = ct{755};
t3621 = ct{756};
t3624 = ct{757};
t3626 = ct{758};
t3628 = ct{759};
t363 = ct{760};
t3630 = ct{761};
t3631 = ct{762};
t3632 = ct{763};
t3633 = ct{764};
t3634 = ct{765};
t3635 = ct{766};
t3636 = ct{767};
t3637 = ct{768};
t3638 = ct{769};
t3639 = ct{770};
t364 = ct{771};
t3640 = ct{772};
t3641 = ct{773};
t3642 = ct{774};
t3643 = ct{775};
t3644 = ct{776};
t3645 = ct{777};
t3646 = ct{778};
t3647 = ct{779};
t3648 = ct{780};
t3649 = ct{781};
t365 = ct{782};
t3650 = ct{783};
t3651 = ct{784};
t3652 = ct{785};
t3653 = ct{786};
t3654 = ct{787};
t3655 = ct{788};
t3656 = ct{789};
t3657 = ct{790};
t3658 = ct{791};
t3659 = ct{792};
t366 = ct{793};
t3660 = ct{794};
t3661 = ct{795};
t3662 = ct{796};
t3664 = ct{797};
t3666 = ct{798};
t3667 = ct{799};
t3668 = ct{800};
t3669 = ct{801};
t3670 = ct{802};
t3671 = ct{803};
t3672 = ct{804};
t3673 = ct{805};
t3674 = ct{806};
t3675 = ct{807};
t3677 = ct{808};
t3678 = ct{809};
t3679 = ct{810};
t3680 = ct{811};
t3681 = ct{812};
t3683 = ct{813};
t3684 = ct{814};
t3688 = ct{815};
t3689 = ct{816};
t3690 = ct{817};
t3692 = ct{818};
t3693 = ct{819};
t3695 = ct{820};
t3696 = ct{821};
t3697 = ct{822};
t3699 = ct{823};
t3700 = ct{824};
t3701 = ct{825};
t3702 = ct{826};
t3703 = ct{827};
t3704 = ct{828};
t3705 = ct{829};
t3706 = ct{830};
t3707 = ct{831};
t3708 = ct{832};
t3709 = ct{833};
t371 = ct{834};
t3710 = ct{835};
t3711 = ct{836};
t3712 = ct{837};
t3713 = ct{838};
t3716 = ct{839};
t3717 = ct{840};
t3719 = ct{841};
t372 = ct{842};
t3721 = ct{843};
t3722 = ct{844};
t3723 = ct{845};
t3726 = ct{846};
t3728 = ct{847};
t3729 = ct{848};
t3731 = ct{849};
t3732 = ct{850};
t3734 = ct{851};
t3735 = ct{852};
t3736 = ct{853};
t3737 = ct{854};
t3738 = ct{855};
t3739 = ct{856};
t3741 = ct{857};
t3743 = ct{858};
t3746 = ct{859};
t3747 = ct{860};
t3749 = ct{861};
t3751 = ct{862};
t3752 = ct{863};
t3753 = ct{864};
t3754 = ct{865};
t3755 = ct{866};
t3759 = ct{867};
t3760 = ct{868};
t3764 = ct{869};
t3765 = ct{870};
t3766 = ct{871};
t3770 = ct{872};
t3771 = ct{873};
t3772 = ct{874};
t3774 = ct{875};
t3775 = ct{876};
t3777 = ct{877};
t3779 = ct{878};
t378 = ct{879};
t3781 = ct{880};
t3782 = ct{881};
t3783 = ct{882};
t3784 = ct{883};
t3785 = ct{884};
t3786 = ct{885};
t3788 = ct{886};
t3789 = ct{887};
t3790 = ct{888};
t3791 = ct{889};
t3792 = ct{890};
t3793 = ct{891};
t3794 = ct{892};
t3795 = ct{893};
t3796 = ct{894};
t3797 = ct{895};
t3798 = ct{896};
t38 = ct{897};
t380 = ct{898};
t3800 = ct{899};
t3801 = ct{900};
t3802 = ct{901};
t3804 = ct{902};
t3805 = ct{903};
t3808 = ct{904};
t3809 = ct{905};
t3810 = ct{906};
t3814 = ct{907};
t3815 = ct{908};
t3817 = ct{909};
t3818 = ct{910};
t3819 = ct{911};
t382 = ct{912};
t3820 = ct{913};
t3821 = ct{914};
t3823 = ct{915};
t3824 = ct{916};
t3826 = ct{917};
t3827 = ct{918};
t3828 = ct{919};
t3830 = ct{920};
t3832 = ct{921};
t3833 = ct{922};
t3834 = ct{923};
t3835 = ct{924};
t3840 = ct{925};
t3843 = ct{926};
t3844 = ct{927};
t3845 = ct{928};
t3846 = ct{929};
t3848 = ct{930};
t3850 = ct{931};
t3851 = ct{932};
t3855 = ct{933};
t3856 = ct{934};
t3857 = ct{935};
t3859 = ct{936};
t3862 = ct{937};
t3863 = ct{938};
t3866 = ct{939};
t3867 = ct{940};
t387 = ct{941};
t3870 = ct{942};
t3873 = ct{943};
t3874 = ct{944};
t3876 = ct{945};
t3877 = ct{946};
t3878 = ct{947};
t3879 = ct{948};
t3880 = ct{949};
t3885 = ct{950};
t3888 = ct{951};
t3889 = ct{952};
t3890 = ct{953};
t3891 = ct{954};
t3893 = ct{955};
t3895 = ct{956};
t3896 = ct{957};
t3897 = ct{958};
t3898 = ct{959};
t39 = ct{960};
t3900 = ct{961};
t3901 = ct{962};
t3902 = ct{963};
t3903 = ct{964};
t3906 = ct{965};
t3908 = ct{966};
t3909 = ct{967};
t3910 = ct{968};
t3913 = ct{969};
t3915 = ct{970};
t3919 = ct{971};
t3924 = ct{972};
t3925 = ct{973};
t3926 = ct{974};
t3931 = ct{975};
t3934 = ct{976};
t3937 = ct{977};
t3939 = ct{978};
t3941 = ct{979};
t3943 = ct{980};
t3949 = ct{981};
t3951 = ct{982};
t3953 = ct{983};
t3954 = ct{984};
t3957 = ct{985};
t3958 = ct{986};
t3959 = ct{987};
t3961 = ct{988};
t3966 = ct{989};
t3967 = ct{990};
t3968 = ct{991};
t3970 = ct{992};
t3971 = ct{993};
t3973 = ct{994};
t3974 = ct{995};
t3975 = ct{996};
t3976 = ct{997};
t3977 = ct{998};
t3979 = ct{999};
t3980 = ct{1000};
t3983 = ct{1001};
t3985 = ct{1002};
t3987 = ct{1003};
t3988 = ct{1004};
t3991 = ct{1005};
t3992 = ct{1006};
t3993 = ct{1007};
t3996 = ct{1008};
t3997 = ct{1009};
t3998 = ct{1010};
t3999 = ct{1011};
t4001 = ct{1012};
t4002 = ct{1013};
t4008 = ct{1014};
t4010 = ct{1015};
t4011 = ct{1016};
t4012 = ct{1017};
t4014 = ct{1018};
t4015 = ct{1019};
t4016 = ct{1020};
t4017 = ct{1021};
t4018 = ct{1022};
t4019 = ct{1023};
t4026 = ct{1024};
t4030 = ct{1025};
t4031 = ct{1026};
t4032 = ct{1027};
t4035 = ct{1028};
t4038 = ct{1029};
t4039 = ct{1030};
t4041 = ct{1031};
t4045 = ct{1032};
t4046 = ct{1033};
t4047 = ct{1034};
t4048 = ct{1035};
t4049 = ct{1036};
t4050 = ct{1037};
t4059 = ct{1038};
t4060 = ct{1039};
t4063 = ct{1040};
t4064 = ct{1041};
t4065 = ct{1042};
t4066 = ct{1043};
t4071 = ct{1044};
t4086 = ct{1045};
t4090 = ct{1046};
t4091 = ct{1047};
t4092 = ct{1048};
t4096 = ct{1049};
t4097 = ct{1050};
t4098 = ct{1051};
t4099 = ct{1052};
t410 = ct{1053};
t4100 = ct{1054};
t4101 = ct{1055};
t4103 = ct{1056};
t4105 = ct{1057};
t4107 = ct{1058};
t4108 = ct{1059};
t4109 = ct{1060};
t4110 = ct{1061};
t4111 = ct{1062};
t4112 = ct{1063};
t4116 = ct{1064};
t4117 = ct{1065};
t4118 = ct{1066};
t4121 = ct{1067};
t4122 = ct{1068};
t4144 = ct{1069};
t4146 = ct{1070};
t4147 = ct{1071};
t4149 = ct{1072};
t4151 = ct{1073};
t4153 = ct{1074};
t4154 = ct{1075};
t4156 = ct{1076};
t4157 = ct{1077};
t4158 = ct{1078};
t4159 = ct{1079};
t4160 = ct{1080};
t4163 = ct{1081};
t4165 = ct{1082};
t4171 = ct{1083};
t4172 = ct{1084};
t4179 = ct{1085};
t4180 = ct{1086};
t4187 = ct{1087};
t4188 = ct{1088};
t4189 = ct{1089};
t4190 = ct{1090};
t4193 = ct{1091};
t4195 = ct{1092};
t4198 = ct{1093};
t42 = ct{1094};
t4200 = ct{1095};
t4201 = ct{1096};
t4204 = ct{1097};
t4205 = ct{1098};
t4207 = ct{1099};
t4208 = ct{1100};
t4210 = ct{1101};
t4213 = ct{1102};
t4215 = ct{1103};
t4218 = ct{1104};
t4219 = ct{1105};
t4224 = ct{1106};
t4229 = ct{1107};
t4230 = ct{1108};
t4236 = ct{1109};
t4237 = ct{1110};
t4240 = ct{1111};
t4241 = ct{1112};
t4243 = ct{1113};
t4244 = ct{1114};
t4246 = ct{1115};
t4248 = ct{1116};
t4249 = ct{1117};
t4258 = ct{1118};
t4260 = ct{1119};
t4261 = ct{1120};
t4263 = ct{1121};
t4265 = ct{1122};
t4270 = ct{1123};
t4272 = ct{1124};
t4273 = ct{1125};
t4274 = ct{1126};
t4275 = ct{1127};
t4276 = ct{1128};
t4277 = ct{1129};
t4278 = ct{1130};
t4279 = ct{1131};
t4280 = ct{1132};
t4281 = ct{1133};
t4282 = ct{1134};
t4283 = ct{1135};
t4286 = ct{1136};
t4287 = ct{1137};
t4288 = ct{1138};
t4289 = ct{1139};
t429 = ct{1140};
t4290 = ct{1141};
t4291 = ct{1142};
t4293 = ct{1143};
t4294 = ct{1144};
t4295 = ct{1145};
t4296 = ct{1146};
t4297 = ct{1147};
t4298 = ct{1148};
t4299 = ct{1149};
t43 = ct{1150};
t4300 = ct{1151};
t4301 = ct{1152};
t4303 = ct{1153};
t4304 = ct{1154};
t4305 = ct{1155};
t4306 = ct{1156};
t4307 = ct{1157};
t4308 = ct{1158};
t4310 = ct{1159};
t4311 = ct{1160};
t4312 = ct{1161};
t4313 = ct{1162};
t4314 = ct{1163};
t4318 = ct{1164};
t4319 = ct{1165};
t4320 = ct{1166};
t4322 = ct{1167};
t4323 = ct{1168};
t4324 = ct{1169};
t4325 = ct{1170};
t4326 = ct{1171};
t4330 = ct{1172};
t4331 = ct{1173};
t4332 = ct{1174};
t4333 = ct{1175};
t4334 = ct{1176};
t4337 = ct{1177};
t4339 = ct{1178};
t4341 = ct{1179};
t4342 = ct{1180};
t4343 = ct{1181};
t4344 = ct{1182};
t4345 = ct{1183};
t4346 = ct{1184};
t4347 = ct{1185};
t4352 = ct{1186};
t4354 = ct{1187};
t4355 = ct{1188};
t4356 = ct{1189};
t4358 = ct{1190};
t4359 = ct{1191};
t4361 = ct{1192};
t4362 = ct{1193};
t4371 = ct{1194};
t4372 = ct{1195};
t4373 = ct{1196};
t4374 = ct{1197};
t4375 = ct{1198};
t4376 = ct{1199};
t4403 = ct{1200};
t4404 = ct{1201};
t4405 = ct{1202};
t4406 = ct{1203};
t4407 = ct{1204};
t4409 = ct{1205};
t4413 = ct{1206};
t4415 = ct{1207};
t4416 = ct{1208};
t4417 = ct{1209};
t4420 = ct{1210};
t4422 = ct{1211};
t4423 = ct{1212};
t4426 = ct{1213};
t4427 = ct{1214};
t4428 = ct{1215};
t4429 = ct{1216};
t4430 = ct{1217};
t4431 = ct{1218};
t4432 = ct{1219};
t4434 = ct{1220};
t4435 = ct{1221};
t4436 = ct{1222};
t4438 = ct{1223};
t4439 = ct{1224};
t4440 = ct{1225};
t4441 = ct{1226};
t4443 = ct{1227};
t4448 = ct{1228};
t4449 = ct{1229};
t4455 = ct{1230};
t4456 = ct{1231};
t4457 = ct{1232};
t4458 = ct{1233};
t4459 = ct{1234};
t4461 = ct{1235};
t4462 = ct{1236};
t4464 = ct{1237};
t4465 = ct{1238};
t4466 = ct{1239};
t4467 = ct{1240};
t4468 = ct{1241};
t4470 = ct{1242};
t4476 = ct{1243};
t4479 = ct{1244};
t4482 = ct{1245};
t4485 = ct{1246};
t4486 = ct{1247};
t4487 = ct{1248};
t4488 = ct{1249};
t4489 = ct{1250};
t4491 = ct{1251};
t4492 = ct{1252};
t4493 = ct{1253};
t4494 = ct{1254};
t4495 = ct{1255};
t4496 = ct{1256};
t4497 = ct{1257};
t4498 = ct{1258};
t4499 = ct{1259};
t4500 = ct{1260};
t4501 = ct{1261};
t4502 = ct{1262};
t4504 = ct{1263};
t4510 = ct{1264};
t4515 = ct{1265};
t4517 = ct{1266};
t4518 = ct{1267};
t4520 = ct{1268};
t4522 = ct{1269};
t4523 = ct{1270};
t4529 = ct{1271};
t4532 = ct{1272};
t4533 = ct{1273};
t4534 = ct{1274};
t4537 = ct{1275};
t4541 = ct{1276};
t4542 = ct{1277};
t4544 = ct{1278};
t4545 = ct{1279};
t4546 = ct{1280};
t4548 = ct{1281};
t4549 = ct{1282};
t4550 = ct{1283};
t4551 = ct{1284};
t4553 = ct{1285};
t4554 = ct{1286};
t4559 = ct{1287};
t4561 = ct{1288};
t4562 = ct{1289};
t4563 = ct{1290};
t4564 = ct{1291};
t4565 = ct{1292};
t4567 = ct{1293};
t4570 = ct{1294};
t4571 = ct{1295};
t4573 = ct{1296};
t4574 = ct{1297};
t4576 = ct{1298};
t4577 = ct{1299};
t4578 = ct{1300};
t4579 = ct{1301};
t4580 = ct{1302};
t4583 = ct{1303};
t4584 = ct{1304};
t4585 = ct{1305};
t4588 = ct{1306};
t4589 = ct{1307};
t4591 = ct{1308};
t4593 = ct{1309};
t4594 = ct{1310};
t4595 = ct{1311};
t4596 = ct{1312};
t4598 = ct{1313};
t4599 = ct{1314};
t46 = ct{1315};
t4602 = ct{1316};
t4605 = ct{1317};
t4606 = ct{1318};
t4608 = ct{1319};
t4609 = ct{1320};
t4612 = ct{1321};
t4613 = ct{1322};
t4614 = ct{1323};
t4615 = ct{1324};
t4618 = ct{1325};
t4623 = ct{1326};
t4625 = ct{1327};
t4626 = ct{1328};
t4634 = ct{1329};
t4635 = ct{1330};
t4637 = ct{1331};
t4643 = ct{1332};
t4644 = ct{1333};
t4645 = ct{1334};
t4646 = ct{1335};
t4647 = ct{1336};
t4648 = ct{1337};
t4649 = ct{1338};
t4650 = ct{1339};
t4651 = ct{1340};
t4652 = ct{1341};
t4654 = ct{1342};
t4656 = ct{1343};
t4657 = ct{1344};
t4658 = ct{1345};
t4660 = ct{1346};
t4663 = ct{1347};
t4665 = ct{1348};
t4667 = ct{1349};
t4669 = ct{1350};
t4670 = ct{1351};
t4672 = ct{1352};
t4673 = ct{1353};
t4674 = ct{1354};
t4675 = ct{1355};
t4676 = ct{1356};
t4677 = ct{1357};
t4678 = ct{1358};
t4680 = ct{1359};
t4681 = ct{1360};
t4682 = ct{1361};
t4683 = ct{1362};
t4684 = ct{1363};
t4685 = ct{1364};
t4686 = ct{1365};
t4687 = ct{1366};
t4690 = ct{1367};
t4691 = ct{1368};
t4692 = ct{1369};
t4694 = ct{1370};
t4696 = ct{1371};
t47 = ct{1372};
t4703 = ct{1373};
t4704 = ct{1374};
t4705 = ct{1375};
t4708 = ct{1376};
t4709 = ct{1377};
t4711 = ct{1378};
t4712 = ct{1379};
t4713 = ct{1380};
t4716 = ct{1381};
t4718 = ct{1382};
t4719 = ct{1383};
t4722 = ct{1384};
t4724 = ct{1385};
t4725 = ct{1386};
t4726 = ct{1387};
t4727 = ct{1388};
t4728 = ct{1389};
t4730 = ct{1390};
t4731 = ct{1391};
t4733 = ct{1392};
t4734 = ct{1393};
t4737 = ct{1394};
t4739 = ct{1395};
t4741 = ct{1396};
t4742 = ct{1397};
t4743 = ct{1398};
t4744 = ct{1399};
t4746 = ct{1400};
t4751 = ct{1401};
t4757 = ct{1402};
t4760 = ct{1403};
t4761 = ct{1404};
t4762 = ct{1405};
t4763 = ct{1406};
t4764 = ct{1407};
t4766 = ct{1408};
t4767 = ct{1409};
t4768 = ct{1410};
t4769 = ct{1411};
t4774 = ct{1412};
t4776 = ct{1413};
t4777 = ct{1414};
t4778 = ct{1415};
t4779 = ct{1416};
t4781 = ct{1417};
t4783 = ct{1418};
t4784 = ct{1419};
t4785 = ct{1420};
t4786 = ct{1421};
t4787 = ct{1422};
t4790 = ct{1423};
t4791 = ct{1424};
t4792 = ct{1425};
t4793 = ct{1426};
t4794 = ct{1427};
t4795 = ct{1428};
t4796 = ct{1429};
t4798 = ct{1430};
t4799 = ct{1431};
t4801 = ct{1432};
t4803 = ct{1433};
t4806 = ct{1434};
t4812 = ct{1435};
t4814 = ct{1436};
t4815 = ct{1437};
t4816 = ct{1438};
t4818 = ct{1439};
t4820 = ct{1440};
t4824 = ct{1441};
t4825 = ct{1442};
t4826 = ct{1443};
t4828 = ct{1444};
t4833 = ct{1445};
t4835 = ct{1446};
t4838 = ct{1447};
t4843 = ct{1448};
t4844 = ct{1449};
t4845 = ct{1450};
t4846 = ct{1451};
t4847 = ct{1452};
t4848 = ct{1453};
t4849 = ct{1454};
t4850 = ct{1455};
t4853 = ct{1456};
t4856 = ct{1457};
t4857 = ct{1458};
t4858 = ct{1459};
t4859 = ct{1460};
t4863 = ct{1461};
t4867 = ct{1462};
t4872 = ct{1463};
t4874 = ct{1464};
t4875 = ct{1465};
t4876 = ct{1466};
t4879 = ct{1467};
t4880 = ct{1468};
t4883 = ct{1469};
t4886 = ct{1470};
t4887 = ct{1471};
t4889 = ct{1472};
t4892 = ct{1473};
t4893 = ct{1474};
t4895 = ct{1475};
t4896 = ct{1476};
t4898 = ct{1477};
t4899 = ct{1478};
t4901 = ct{1479};
t4902 = ct{1480};
t4904 = ct{1481};
t4907 = ct{1482};
t4911 = ct{1483};
t4912 = ct{1484};
t4915 = ct{1485};
t4918 = ct{1486};
t4919 = ct{1487};
t4920 = ct{1488};
t4921 = ct{1489};
t4922 = ct{1490};
t4923 = ct{1491};
t4924 = ct{1492};
t4925 = ct{1493};
t4926 = ct{1494};
t4927 = ct{1495};
t4928 = ct{1496};
t4929 = ct{1497};
t4930 = ct{1498};
t4933 = ct{1499};
t4934 = ct{1500};
t4935 = ct{1501};
t4936 = ct{1502};
t4937 = ct{1503};
t4938 = ct{1504};
t4939 = ct{1505};
t4940 = ct{1506};
t4941 = ct{1507};
t4943 = ct{1508};
t4945 = ct{1509};
t4946 = ct{1510};
t4947 = ct{1511};
t4950 = ct{1512};
t4952 = ct{1513};
t4953 = ct{1514};
t4955 = ct{1515};
t4958 = ct{1516};
t4969 = ct{1517};
t4973 = ct{1518};
t4974 = ct{1519};
t4977 = ct{1520};
t4979 = ct{1521};
t50 = ct{1522};
t5001 = ct{1523};
t5003 = ct{1524};
t5004 = ct{1525};
t5005 = ct{1526};
t5012 = ct{1527};
t5013 = ct{1528};
t5014 = ct{1529};
t5016 = ct{1530};
t5019 = ct{1531};
t5020 = ct{1532};
t5024 = ct{1533};
t5025 = ct{1534};
t5026 = ct{1535};
t5027 = ct{1536};
t5028 = ct{1537};
t5033 = ct{1538};
t5034 = ct{1539};
t5035 = ct{1540};
t5036 = ct{1541};
t5037 = ct{1542};
t5038 = ct{1543};
t5041 = ct{1544};
t5042 = ct{1545};
t5043 = ct{1546};
t5045 = ct{1547};
t5046 = ct{1548};
t5047 = ct{1549};
t5049 = ct{1550};
t5051 = ct{1551};
t5052 = ct{1552};
t5053 = ct{1553};
t5059 = ct{1554};
t5061 = ct{1555};
t5062 = ct{1556};
t5063 = ct{1557};
t5064 = ct{1558};
t5066 = ct{1559};
t5070 = ct{1560};
t5071 = ct{1561};
t5072 = ct{1562};
t5074 = ct{1563};
t5075 = ct{1564};
t5076 = ct{1565};
t5077 = ct{1566};
t5079 = ct{1567};
t5080 = ct{1568};
t5081 = ct{1569};
t5082 = ct{1570};
t5083 = ct{1571};
t5084 = ct{1572};
t5085 = ct{1573};
t5086 = ct{1574};
t5087 = ct{1575};
t5088 = ct{1576};
t5089 = ct{1577};
t5090 = ct{1578};
t5091 = ct{1579};
t5093 = ct{1580};
t5096 = ct{1581};
t5097 = ct{1582};
t5098 = ct{1583};
t5100 = ct{1584};
t5101 = ct{1585};
t5103 = ct{1586};
t5106 = ct{1587};
t5108 = ct{1588};
t5111 = ct{1589};
t5113 = ct{1590};
t5114 = ct{1591};
t5117 = ct{1592};
t5118 = ct{1593};
t5119 = ct{1594};
t5123 = ct{1595};
t5124 = ct{1596};
t5126 = ct{1597};
t5127 = ct{1598};
t5141 = ct{1599};
t5142 = ct{1600};
t5144 = ct{1601};
t5146 = ct{1602};
t5155 = ct{1603};
t5158 = ct{1604};
t5161 = ct{1605};
t5163 = ct{1606};
t5164 = ct{1607};
t5165 = ct{1608};
t5166 = ct{1609};
t5168 = ct{1610};
t5169 = ct{1611};
t5171 = ct{1612};
t5173 = ct{1613};
t5174 = ct{1614};
t5176 = ct{1615};
t5177 = ct{1616};
t5178 = ct{1617};
t5180 = ct{1618};
t5181 = ct{1619};
t5194 = ct{1620};
t5195 = ct{1621};
t5196 = ct{1622};
t5197 = ct{1623};
t5198 = ct{1624};
t5199 = ct{1625};
t5200 = ct{1626};
t5201 = ct{1627};
t5202 = ct{1628};
t5203 = ct{1629};
t5205 = ct{1630};
t5208 = ct{1631};
t5212 = ct{1632};
t5213 = ct{1633};
t5214 = ct{1634};
t5215 = ct{1635};
t5219 = ct{1636};
t5234 = ct{1637};
t5240 = ct{1638};
t5241 = ct{1639};
t5243 = ct{1640};
t5244 = ct{1641};
t5246 = ct{1642};
t5247 = ct{1643};
t5248 = ct{1644};
t5249 = ct{1645};
t5251 = ct{1646};
t5254 = ct{1647};
t5255 = ct{1648};
t5256 = ct{1649};
t5257 = ct{1650};
t5258 = ct{1651};
t5259 = ct{1652};
t5261 = ct{1653};
t5262 = ct{1654};
t5263 = ct{1655};
t5264 = ct{1656};
t5265 = ct{1657};
t5266 = ct{1658};
t5267 = ct{1659};
t5268 = ct{1660};
t5269 = ct{1661};
t5271 = ct{1662};
t5272 = ct{1663};
t5273 = ct{1664};
t5274 = ct{1665};
t5276 = ct{1666};
t5277 = ct{1667};
t5278 = ct{1668};
t5279 = ct{1669};
t5280 = ct{1670};
t5281 = ct{1671};
t5283 = ct{1672};
t5284 = ct{1673};
t5285 = ct{1674};
t5286 = ct{1675};
t5287 = ct{1676};
t5288 = ct{1677};
t5289 = ct{1678};
t5290 = ct{1679};
t5291 = ct{1680};
t5292 = ct{1681};
t5293 = ct{1682};
t5294 = ct{1683};
t5295 = ct{1684};
t5296 = ct{1685};
t5297 = ct{1686};
t5298 = ct{1687};
t5300 = ct{1688};
t5301 = ct{1689};
t5302 = ct{1690};
t5303 = ct{1691};
t5304 = ct{1692};
t5305 = ct{1693};
t5306 = ct{1694};
t5308 = ct{1695};
t5309 = ct{1696};
t5310 = ct{1697};
t5312 = ct{1698};
t5315 = ct{1699};
t5316 = ct{1700};
t5318 = ct{1701};
t5320 = ct{1702};
t5321 = ct{1703};
t5322 = ct{1704};
t5324 = ct{1705};
t5325 = ct{1706};
t5327 = ct{1707};
t5328 = ct{1708};
t5329 = ct{1709};
t5330 = ct{1710};
t5331 = ct{1711};
t5332 = ct{1712};
t5336 = ct{1713};
t5337 = ct{1714};
t5340 = ct{1715};
t5343 = ct{1716};
t5344 = ct{1717};
t5345 = ct{1718};
t5346 = ct{1719};
t5348 = ct{1720};
t5350 = ct{1721};
t5352 = ct{1722};
t5353 = ct{1723};
t5354 = ct{1724};
t5356 = ct{1725};
t5357 = ct{1726};
t5358 = ct{1727};
t5359 = ct{1728};
t5361 = ct{1729};
t5362 = ct{1730};
t5363 = ct{1731};
t5370 = ct{1732};
t5372 = ct{1733};
t5374 = ct{1734};
t5378 = ct{1735};
t5381 = ct{1736};
t5383 = ct{1737};
t5384 = ct{1738};
t5387 = ct{1739};
t5389 = ct{1740};
t5391 = ct{1741};
t5392 = ct{1742};
t5393 = ct{1743};
t5395 = ct{1744};
t5399 = ct{1745};
t5400 = ct{1746};
t5401 = ct{1747};
t5402 = ct{1748};
t5403 = ct{1749};
t5404 = ct{1750};
t5410 = ct{1751};
t5411 = ct{1752};
t5412 = ct{1753};
t5415 = ct{1754};
t5416 = ct{1755};
t5419 = ct{1756};
t5424 = ct{1757};
t5425 = ct{1758};
t5433 = ct{1759};
t5434 = ct{1760};
t5436 = ct{1761};
t5437 = ct{1762};
t5438 = ct{1763};
t5439 = ct{1764};
t5440 = ct{1765};
t5441 = ct{1766};
t5442 = ct{1767};
t5443 = ct{1768};
t5444 = ct{1769};
t5445 = ct{1770};
t5446 = ct{1771};
t5448 = ct{1772};
t5449 = ct{1773};
t5452 = ct{1774};
t5456 = ct{1775};
t5457 = ct{1776};
t5458 = ct{1777};
t5459 = ct{1778};
t5460 = ct{1779};
t5461 = ct{1780};
t5462 = ct{1781};
t5464 = ct{1782};
t5465 = ct{1783};
t5472 = ct{1784};
t5474 = ct{1785};
t5481 = ct{1786};
t5487 = ct{1787};
t5488 = ct{1788};
t5494 = ct{1789};
t5495 = ct{1790};
t5499 = ct{1791};
t5500 = ct{1792};
t5501 = ct{1793};
t5503 = ct{1794};
t5504 = ct{1795};
t5506 = ct{1796};
t5507 = ct{1797};
t5509 = ct{1798};
t5510 = ct{1799};
t5512 = ct{1800};
t5513 = ct{1801};
t5514 = ct{1802};
t5516 = ct{1803};
t5517 = ct{1804};
t5520 = ct{1805};
t5522 = ct{1806};
t5523 = ct{1807};
t5524 = ct{1808};
t5535 = ct{1809};
t5536 = ct{1810};
t5537 = ct{1811};
t5538 = ct{1812};
t5539 = ct{1813};
t5540 = ct{1814};
t5541 = ct{1815};
t5542 = ct{1816};
t5543 = ct{1817};
t5544 = ct{1818};
t5545 = ct{1819};
t5548 = ct{1820};
t5549 = ct{1821};
t5550 = ct{1822};
t5555 = ct{1823};
t5556 = ct{1824};
t5560 = ct{1825};
t5561 = ct{1826};
t5565 = ct{1827};
t5567 = ct{1828};
t5568 = ct{1829};
t5569 = ct{1830};
t5570 = ct{1831};
t5575 = ct{1832};
t5576 = ct{1833};
t5577 = ct{1834};
t5578 = ct{1835};
t5586 = ct{1836};
t5590 = ct{1837};
t5591 = ct{1838};
t5592 = ct{1839};
t5595 = ct{1840};
t5599 = ct{1841};
t56 = ct{1842};
t5602 = ct{1843};
t5604 = ct{1844};
t5605 = ct{1845};
t5607 = ct{1846};
t5608 = ct{1847};
t5609 = ct{1848};
t5611 = ct{1849};
t5612 = ct{1850};
t5620 = ct{1851};
t5624 = ct{1852};
t5627 = ct{1853};
t5653 = ct{1854};
t5658 = ct{1855};
t5660 = ct{1856};
t5662 = ct{1857};
t5677 = ct{1858};
t5678 = ct{1859};
t5684 = ct{1860};
t5698 = ct{1861};
t5699 = ct{1862};
t5705 = ct{1863};
t5719 = ct{1864};
t5721 = ct{1865};
t5722 = ct{1866};
t5730 = ct{1867};
t5731 = ct{1868};
t5734 = ct{1869};
t5735 = ct{1870};
t5737 = ct{1871};
t5738 = ct{1872};
t5739 = ct{1873};
t5741 = ct{1874};
t5742 = ct{1875};
t5744 = ct{1876};
t5757 = ct{1877};
t5758 = ct{1878};
t5759 = ct{1879};
t5760 = ct{1880};
t5761 = ct{1881};
t5768 = ct{1882};
t5775 = ct{1883};
t5777 = ct{1884};
t5779 = ct{1885};
t5781 = ct{1886};
t5782 = ct{1887};
t5783 = ct{1888};
t5784 = ct{1889};
t5788 = ct{1890};
t58 = ct{1891};
t5813 = ct{1892};
t5818 = ct{1893};
t5825 = ct{1894};
t5849 = ct{1895};
t5852 = ct{1896};
t5891 = ct{1897};
t5892 = ct{1898};
t5896 = ct{1899};
t59 = ct{1900};
t5901 = ct{1901};
t5902 = ct{1902};
t5908 = ct{1903};
t5909 = ct{1904};
t5916 = ct{1905};
t5917 = ct{1906};
t5922 = ct{1907};
t5924 = ct{1908};
t5925 = ct{1909};
t5928 = ct{1910};
t5933 = ct{1911};
t5938 = ct{1912};
t5941 = ct{1913};
t5954 = ct{1914};
t5955 = ct{1915};
t5966 = ct{1916};
t5971 = ct{1917};
t5990 = ct{1918};
t60 = ct{1919};
t6002 = ct{1920};
t6004 = ct{1921};
t6005 = ct{1922};
t6011 = ct{1923};
t6013 = ct{1924};
t6014 = ct{1925};
t6048 = ct{1926};
t6050 = ct{1927};
t6051 = ct{1928};
t6062 = ct{1929};
t6074 = ct{1930};
t6075 = ct{1931};
t6078 = ct{1932};
t6123 = ct{1933};
t6125 = ct{1934};
t6132 = ct{1935};
t6143 = ct{1936};
t6166 = ct{1937};
t6211 = ct{1938};
t6221 = ct{1939};
t6222 = ct{1940};
t6255 = ct{1941};
t6256 = ct{1942};
t6257 = ct{1943};
t6271 = ct{1944};
t628 = ct{1945};
t638 = ct{1946};
t6394 = ct{1947};
t6396 = ct{1948};
t6398 = ct{1949};
t640 = ct{1950};
t642 = ct{1951};
t643 = ct{1952};
t6442 = ct{1953};
t6482 = ct{1954};
t649 = ct{1955};
t6523 = ct{1956};
t654 = ct{1957};
t655 = ct{1958};
t656 = ct{1959};
t6564 = ct{1960};
t6565 = ct{1961};
t657 = ct{1962};
t6574 = ct{1963};
t6588 = ct{1964};
t6589 = ct{1965};
t659 = ct{1966};
t660 = ct{1967};
t6622 = ct{1968};
t6623 = ct{1969};
t665 = ct{1970};
t6651 = ct{1971};
t667 = ct{1972};
t668 = ct{1973};
t669 = ct{1974};
t67 = ct{1975};
t670 = ct{1976};
t672 = ct{1977};
t673 = ct{1978};
t674 = ct{1979};
t6745 = ct{1980};
t675 = ct{1981};
t6751 = ct{1982};
t676 = ct{1983};
t677 = ct{1984};
t68 = ct{1985};
t681 = ct{1986};
t682 = ct{1987};
t684 = ct{1988};
t685 = ct{1989};
t686 = ct{1990};
t687 = ct{1991};
t691 = ct{1992};
t6919 = ct{1993};
t692 = ct{1994};
t6920 = ct{1995};
t693 = ct{1996};
t694 = ct{1997};
t6966 = ct{1998};
t6987 = ct{1999};
t70 = ct{2000};
t7005 = ct{2001};
t702 = ct{2002};
t707 = ct{2003};
t708 = ct{2004};
t7088 = ct{2005};
t7089 = ct{2006};
t71 = ct{2007};
t710 = ct{2008};
t7138 = ct{2009};
t7148 = ct{2010};
t715 = ct{2011};
t7150 = ct{2012};
t7152 = ct{2013};
t716 = ct{2014};
t7160 = ct{2015};
t717 = ct{2016};
t7172 = ct{2017};
t718 = ct{2018};
t721 = ct{2019};
t722 = ct{2020};
t724 = ct{2021};
t725 = ct{2022};
t73 = ct{2023};
t7304 = ct{2024};
t7319 = ct{2025};
t7331 = ct{2026};
t7332 = ct{2027};
t7333 = ct{2028};
t7334 = ct{2029};
t736 = ct{2030};
t738 = ct{2031};
t740 = ct{2032};
t741 = ct{2033};
t749 = ct{2034};
t756 = ct{2035};
t76 = ct{2036};
t762 = ct{2037};
t768 = ct{2038};
t777 = ct{2039};
t792 = ct{2040};
t793 = ct{2041};
t8 = ct{2042};
t801 = ct{2043};
t802 = ct{2044};
t808 = ct{2045};
t813 = ct{2046};
t819 = ct{2047};
t821 = ct{2048};
t850 = ct{2049};
t855 = ct{2050};
t874 = ct{2051};
t878 = ct{2052};
t89 = ct{2053};
t9 = ct{2054};
t90 = ct{2055};
t91 = ct{2056};
t92 = ct{2057};
t941 = ct{2058};
t944 = ct{2059};
t948 = ct{2060};
t951 = ct{2061};
t97 = ct{2062};
t5525 = t3547.*t5346;
t5526 = t3550.*t5345;
t5527 = t3550.*t5346;
t5530 = -t5353.*(t1896-t3239);
t5531 = t3547.*t5353;
t5532 = t5353.*(t1896-t3239);
t5587 = (t4374.*t5200)./2.0;
t5589 = (t4374.*t5201)./2.0;
t5593 = (t4376.*t5205)./2.0;
t5594 = t1207+t1208+t1221+t1235+t2149+t2150+t2151+t2168+t2744+t3399+t3402+t3419+t3719+t3721;
t5596 = t5318.*(t2694-t2701+t3036-t3043).*(-1.02e-6);
t5597 = t5318.*(t2694-t2701+t3036-t3043).*1.02e-6;
t5598 = t5318.*(t2694-t2701+t3036-t3043).*(-9.0e-8);
t5600 = t5318.*(t2694-t2701+t3036-t3043).*9.0e-8;
t5601 = -t5599;
t5606 = -t5602;
t5610 = t3764+t3859+t3866+t3870+t3939;
t5613 = t3369.*t5200.*(t2694-t2701+t3036-t3043).*(-1.444822e-2);
t5614 = t3369.*t5200.*(t2694-t2701+t3036-t3043).*1.444822e-2;
t5615 = t3369.*t5201.*(t2694-t2701+t3036-t3043).*(-1.444822e-2);
t5616 = t3369.*t5201.*(t2694-t2701+t3036-t3043).*1.444822e-2;
t5617 = t5318.*(t3242-t3554).*(-1.02e-6);
t5619 = t5318.*(t3242-t3554).*1.02e-6;
t5621 = t5318.*(t3242-t3554).*(-9.0e-8);
t5623 = -t5620;
t5625 = t5318.*(t3242-t3554).*9.0e-8;
t5629 = -t5627;
t5630 = t4026.*t5320.*9.3e-7;
t5631 = t3369.*t3934.*t5205.*1.444822e-2;
t5633 = t4026.*t5321.*1.02e-6;
t5634 = t4026.*t5320.*9.0e-8;
t5635 = t4026.*t5321.*9.0e-8;
t5636 = -t5354.*(t3242-t3554);
t5637 = t4026.*t5354;
t5649 = t4215.*t4939.*(t2694-t2701+t3036-t3043).*(-5.43845e-3);
t5650 = t4215.*t4939.*(t2694-t2701+t3036-t3043).*5.43845e-3;
t5654 = t5346.*(t3941-(t262.*(t46-t47))./9.007199254740992e+15);
t5655 = -t5653;
t5656 = t4149.*t5346;
t5659 = -t5658;
t5663 = (t4171-t4896).*(t2813-t2835+t12.*(t1456-t2355).*1.02e-6+t17.*(t1456-t2355).*9.0e-8);
t5664 = t2298+t3300+t3591+t3601+t3602+t3616+t3619+t3628;
t5674 = t3333+t3353+t3650+t3658+t4116+t4117;
t5675 = t3649.*t3934.*t5200.*1.444822e-2;
t5679 = t4172.*t5024.*(t2674-t2676+t3022-t3027).*(-1.0./2.0);
t5680 = (t4172.*t5024.*(t2674-t2676+t3022-t3027))./2.0;
t5696 = t2397+t3348+t3639+t3647+t3648+t3666+t3668+t3669;
t5697 = t2369+t2423+t3341+t3361+t3580+t3639+t3647+t3668+t3669;
t5717 = (t4322.*t5358)./2.0;
t5720 = (t4322.*t5359)./2.0;
t5724 = (t4323.*t5362)./2.0;
t5725 = t201.*t5699.*4.297799892626299e-1;
t5726 = t201.*t5699.*8.595599785252598e-1;
t5736 = t50.*t202.*t5699.*9.543032792050485e-17;
t5745 = (t3216.*t5595)./2.0;
t5748 = t2363.*t5698;
t5750 = t2419.*t5698;
t5751 = (t2388.*t5698)./2.0;
t5763 = t3322.*t5358.*(t2674-t2676+t3022-t3027).*(-1.0./2.0);
t5764 = (t3322.*t5358.*(t2674-t2676+t3022-t3027))./2.0;
t5765 = t3322.*t5359.*(t2674-t2676+t3022-t3027).*(-1.0./2.0);
t5766 = (t3322.*t5359.*(t2674-t2676+t3022-t3027))./2.0;
t5769 = (t3322.*t3910.*t5362)./2.0;
t5776 = -t5775;
t5778 = -t5777;
t5785 = -t5784;
t5787 = (t3638.*t3910.*t5358)./2.0;
t5789 = t3051+t3073+t4012+t4017+t4066+t4097;
t5790 = t4405+t5378;
t5804 = t3236.*t5699;
t5805 = t3237.*t5699;
t5807 = t3085+t3086+t4092+t4096+t4099+t4107;
t5808 = t4237+t4682+t4734;
t5812 = -t2363.*(t3067+t4016-t4066+t4091+(t11.*t3236.*(t1861-t3221))./1.0e+8-t11.*t50.*t202.*t2297.*9.543032792050485e-25);
t5814 = t2363.*(t3067+t4016-t4066+t4091+(t11.*t3236.*(t1861-t3221))./1.0e+8-t11.*t50.*t202.*t2297.*9.543032792050485e-25);
t5821 = t3543.*t5698;
t5822 = -t5698.*(t1896-t3239);
t5823 = t3547.*t5698;
t5824 = t3550.*t5698;
t5835 = t5595.*(t2674-t2676+t3022-t3027).*(-1.0./2.0);
t5836 = (t5595.*(t2674-t2676+t3022-t3027))./2.0;
t5842 = t50.*t189.*t5818.*4.771516396025243e-17;
t5851 = (t2297.*t5818)./2.0;
t5853 = t5852./2.0;
t5863 = (t1896-t3239).*(t3067+t4016-t4066+t4091+(t11.*t3236.*(t1861-t3221))./1.0e+8-t11.*t50.*t202.*t2297.*9.543032792050485e-25);
t5864 = -t3547.*(t3067+t4016-t4066+t4091+(t11.*t3236.*(t1861-t3221))./1.0e+8-t11.*t50.*t202.*t2297.*9.543032792050485e-25);
t5865 = t3937.*t5699;
t5866 = -t5699.*(t1959-t3313+t38.*t1022.*(t855-t878).*2.196325630278387e-1);
t5885 = t4151.*t5698;
t5886 = -t5698.*(t1005+t20.*(t1941-t3315+t39.*t1022.*(t855-t878).*2.196325630278387e-1));
t5887 = t5698.*(t1005+t20.*(t1941-t3315+t39.*t1022.*(t855-t878).*2.196325630278387e-1));
t5919 = t5200.*(t1196+t1212+t1237+t1238+t2139+t2140+t2159+t2165+t2754+t2814+t2953+t3072+t3415+t3423).*(-1.0./2.0);
t5930 = t5358.*(t649+t670+t686+t687+t1577+t1578+t1586+t1600+t2303+t2339+t2689+t3030+t3299+t3312).*(-1.0./2.0);
t5959 = t3712.*t3910.*(t350+t366-t1205+t1210-t1217-t1218-t2147+t2152+t2154+t2155-t3405-t3409-t3420-t3739+t3746+t26.*t50.*t202.*(t46-t47).*8.687615694748404e-39).*(-1.0./2.0);
t5960 = (t3712.*t3910.*(t350+t366-t1205+t1210-t1217-t1218-t2147+t2152+t2154+t2155-t3405-t3409-t3420-t3739+t3746+t26.*t50.*t202.*(t46-t47).*8.687615694748404e-39))./2.0;
t5978 = t3808.*t3910.*(t350+t366-t1205+t1210-t1217-t1218-t2147+t2152+t2154+t2155-t3405-t3409-t3420-t3739+t3746+t26.*t50.*t202.*(t46-t47).*8.687615694748404e-39).*(-1.0./2.0);
t5979 = (t3808.*t3910.*(t350+t366-t1205+t1210-t1217-t1218-t2147+t2152+t2154+t2155-t3405-t3409-t3420-t3739+t3746+t26.*t50.*t202.*(t46-t47).*8.687615694748404e-39))./2.0;
t6019 = t201.*t6005.*4.297799892626299e-1;
t6022 = (t2388.*t6004)./2.0;
t6024 = (t2419.*t6004)./2.0;
t6030 = t4498+t4500+t4510+t4529;
t6031 = t4726+t5705;
t6040 = t4541+t4546+t4548+t4550;
t6054 = t3236.*t6005;
t6056 = t3237.*t6005;
t6059 = t4742+t5744;
t6063 = t4820+t5737;
t6066 = t50.*t189.*t6051.*4.771516396025243e-17;
t6068 = t3543.*t6004;
t6069 = -t6004.*(t1896-t3239);
t6070 = t3547.*t6004;
t6072 = t3550.*t6004;
t6076 = (t2297.*t6051)./2.0;
t6079 = -t6078;
t6080 = t6078./2.0;
t6090 = t3834+t3867+t3900+t4331+t4347+t4420;
t6091 = t50.*t189.*t6075.*4.771516396025243e-17;
t6093 = (t3047.*t6051)./2.0;
t6095 = (t2297.*t6075)./2.0;
t6118 = (t3047.*t6075)./2.0;
t6126 = t3937.*t6005;
t6127 = -t6005.*(t1959-t3313+t38.*t1022.*(t855-t878).*2.196325630278387e-1);
et106 = -t2125-t2142+t2745-t2750+t2774+t2785+t2786-t3470+t4038+t26.*(t1941-t3315+t39.*t1022.*(t855-t878).*2.196325630278387e-1).*1.869599668e-7;
et107 = t38.*t1022.*(t855-t878).*1.46680315462752e-4;
t6128 = t5200.*(et106+et107).*(-1.0./2.0);
et108 = -t2125-t2142+t2745-t2750+t2774+t2785+t2786-t3470+t4038+t26.*(t1941-t3315+t39.*t1022.*(t855-t878).*2.196325630278387e-1).*1.869599668e-7;
et109 = t38.*t1022.*(t855-t878).*1.46680315462752e-4;
t6129 = (t5200.*(et108+et109))./2.0;
et110 = -t2125-t2142+t2745-t2750+t2774+t2785+t2786-t3470+t4038+t26.*(t1941-t3315+t39.*t1022.*(t855-t878).*2.196325630278387e-1).*1.869599668e-7;
et111 = t38.*t1022.*(t855-t878).*1.46680315462752e-4;
t6130 = t5201.*(et110+et111).*(-1.0./2.0);
et112 = -t2125-t2142+t2745-t2750+t2774+t2785+t2786-t3470+t4038+t26.*(t1941-t3315+t39.*t1022.*(t855-t878).*2.196325630278387e-1).*1.869599668e-7;
et113 = t38.*t1022.*(t855-t878).*1.46680315462752e-4;
t6131 = (t5201.*(et112+et113))./2.0;
t6133 = -t6132;
et114 = -t2748-t2749+t2773+t2781-t2788+t3211+t3471+t4032-t4047+t262.*(t46-t47).*2.075672598245148e-23;
et115 = t264.*(t46-t47).*1.875105520197095e-20;
t6134 = t5205.*(et114+et115).*(-1.0./2.0);
t6154 = t4151.*t6004;
t6155 = -t6004.*(t1005+t20.*(t1941-t3315+t39.*t1022.*(t855-t878).*2.196325630278387e-1));
t6158 = t6004.*(t1005+t20.*(t1941-t3315+t39.*t1022.*(t855-t878).*2.196325630278387e-1));
t6162 = (t5358.*t5560)./2.0;
t6164 = (t5359.*t5560)./2.0;
t6167 = t3050+t3087+t3088+t4011+t4015+t4098+t4101+t4103+t4108;
t6168 = (t5362.*t5561)./2.0;
t6183 = t5278.*(t350+t366-t1205+t1210-t1217-t1218-t2147+t2152+t2154+t2155-t3405-t3409-t3420-t3739+t3746+t26.*t50.*t202.*(t46-t47).*8.687615694748404e-39).*(-1.0./2.0);
t6203 = t3680+t3683+t4455+t4456+t4485+t4487;
t6381 = t3987+t4236+t4333+t4403+t4462+t4648;
t6397 = -t6396;
t6425 = (t5024.*t6011)./2.0;
t6440 = (t3910.*t4172.*t6048)./2.0;
t6460 = t3216.*(t3885+t4681-t4731+t3815.*(t3242-t3554)+t3819.*(t3242-t3554)).*(-1.0./2.0);
t6461 = (t3216.*(t3885+t4681-t4731+t3815.*(t3242-t3554)+t3819.*(t3242-t3554)))./2.0;
t6483 = -t6482;
t6491 = ((t1861-t3221).*(t3885+t4681-t4731+t3815.*(t3242-t3554)+t3819.*(t3242-t3554)))./2.0;
t6517 = t5783.*(t350+t366-t1205+t1210-t1217-t1218-t2147+t2152+t2154+t2155-t3405-t3409-t3420-t3739+t3746+t26.*t50.*t202.*(t46-t47).*8.687615694748404e-39).*(-1.0./2.0);
t6524 = -t6523;
t6527 = ((t2674-t2676+t3022-t3027).*(t3885+t4681-t4731+t3815.*(t3242-t3554)+t3819.*(t3242-t3554)))./2.0;
t6581 = t4492+t4499+t4544+t4549+t4551+t4554;
t6587 = t2320+t2378+t2510+t2534+t2978+t2979+t3926+t4144+t4190+t4193+t4863+t4867;
t6594 = (t4939.*t6255)./2.0;
t6602 = (t2388.*t6589)./2.0;
t6661 = t3543.*t6589;
t6662 = t3550.*t6589;
et116 = t1554+t2361+t2362+t2367+t2414+t3961+t3968+t4198+t4201+t11.*(-t1901+t3122+t3277).*5.68686e-3;
et117 = (t350+t366-t1205+t1210-t1217-t1218-t2147+t2152+t2154+t2155-t3405-t3409-t3420-t3739+t3746+t26.*t50.*t202.*(t46-t47).*8.687615694748404e-39)./2.0;
t6680 = et116.*et117;
t6961 = t4204+t4637+t4658+t4719+t5240+t5262;
t6965 = (t2694-t2701+t3036-t3043).*(t1513+t1879+t2598+t2820+t2834+t3117+t3118).*(-t2308+t2378+t2510-t2530-t2975+t2979+t3926+t4144+t4190+t4193+t4863+t4867).*3.633675e-3;
t7003 = (t3216.*(t4658+t4719+t5240+t5262-t3483.*(t1005+t20.*(t1941-t3315+t39.*t1022.*(t855-t878).*2.196325630278387e-1))-t3431.*(t1896-t3239)))./2.0;
et118 = t707+t708-t721-t722-t749+t762+t768-t777-t792-t793-t801-t802-t808+t813-t819+t821-t1629+t1637-t1640-t1641-t1659-t1661+t1666+t1667+t1683+t1692+t1705-t1712+t1758+t1759+t1775+t1776+t1973+t1993+t1994+t2023+t2053+t2060-t2089-t2090+t2098+t2099-t8.*t9.*t15.*t50.*t189.*3.670836568391568e-22;
et119 = t10.*t13.*t14.*t50.*t189.*(-3.279367663374749e-19)-t8.*t9.*t11.*t15.*t50.*t189.*7.075931802640439e-19;
et120 = t8.*t11.*t14.*t15.*t50.*t189.*(-1.190170786299927e-18)-t9.*t11.*t13.*t15.*t50.*t189.*1.190170786299927e-18;
et121 = t13.*t14.*t15.*t16.*t50.*t189.*(-3.226512155691387e-19);
t7006 = t6048.*(et118+et119+et120+et121).*(-1.0./2.0);
et122 = t707+t708-t721-t722-t749+t762+t768-t777-t792-t793-t801-t802-t808+t813-t819+t821-t1629+t1637-t1640-t1641-t1659-t1661+t1666+t1667+t1683+t1692+t1705-t1712+t1758+t1759+t1775+t1776+t1973+t1993+t1994+t2023+t2053+t2060-t2089-t2090+t2098+t2099-t8.*t9.*t15.*t50.*t189.*3.670836568391568e-22;
et123 = t10.*t13.*t14.*t50.*t189.*(-3.279367663374749e-19)-t8.*t9.*t11.*t15.*t50.*t189.*7.075931802640439e-19;
et124 = t8.*t11.*t14.*t15.*t50.*t189.*(-1.190170786299927e-18)-t9.*t11.*t13.*t15.*t50.*t189.*1.190170786299927e-18;
et125 = t13.*t14.*t15.*t16.*t50.*t189.*(-3.226512155691387e-19);
t7007 = (t6048.*(et122+et123+et124+et125))./2.0;
t7014 = (t6651.*(t2674-t2676+t3022-t3027).*(t1488+t1874+t2519+t2740+t2747+t3096+t3097))./2.0;
t7035 = (t1861-t3221).*(t4658+t4719+t5240+t5262-t3483.*(t1005+t20.*(t1941-t3315+t39.*t1022.*(t855-t878).*2.196325630278387e-1))-t3431.*(t1896-t3239)).*(-1.0./2.0);
t7086 = (t2674-t2676+t3022-t3027).*(t4658+t4719+t5240+t5262-t3483.*(t1005+t20.*(t1941-t3315+t39.*t1022.*(t855-t878).*2.196325630278387e-1))-t3431.*(t1896-t3239)).*(-1.0./2.0);
t7087 = ((t2674-t2676+t3022-t3027).*(t4658+t4719+t5240+t5262-t3483.*(t1005+t20.*(t1941-t3315+t39.*t1022.*(t855-t878).*2.196325630278387e-1))-t3431.*(t1896-t3239)))./2.0;
t7093 = t50.*t202.*t7089.*4.771516396025243e-17;
t7094 = t50.*t202.*t7089.*9.543032792050485e-17;
t7096 = t2363.*t7088;
t7116 = t1544+t1559+t2320+t2323+t2329+t2341+t2379+t2380+t2510+t2534+t2978+t2979+t3153+t3377+t3926+t3953+t3973+t4144+t4190+t4193+t4863+t4867;
t7134 = t3236.*t7089;
t7135 = t3237.*t7089;
t7137 = t50.*t189.*(t1548+t1564+t2308-t2323+t2326+t2343+t2352+t2353-t2510+t2530+t2975-t2979+t3150+t3379-t3926+t3958+t3970+t4189-t4190-t4863-t4867+t16.*(t944-t3919).*(3.0./5.0e+2)).*(-9.543032792050485e-17);
t7139 = t1547+t2320+t2364+t2378+t2384+t2394+t2395+t2510+t2534+t2978+t2979+t3957+t3959+t3971+t4190+t4193+t4195+t4210+t4863+t4867;
t7153 = -t7088.*(t1896-t3239);
t7154 = t3547.*t7088;
t7158 = -t2297.*(t1553+t2308+t2359+t2365+t2366-t2378+t2389-t2510+t2530+t2975-t2979+t3954+t3966-t3971+t4189-t4190+t4200-t4863-t4867+t16.*(t944-t3919).*3.131399999999998e-4);
t7167 = t50.*t202.*t7152.*6.935255936130809e-19;
t7199 = t2363.*t7172.*7.26735e-3;
t4006 = t12.*t4001;
t4007 = t17.*t4001;
t4051 = t22.*t4031;
t4052 = t28.*t4031;
t4053 = -t4046;
t4054 = -t4048;
t4056 = -t4049;
t4113 = -t4109;
t4114 = -t4111;
t4115 = -t4112;
t4168 = -t4157;
t4267 = t3519+t3528;
t4292 = t3568+t3584;
t4321 = -t4320;
t4363 = t3133.*t4031;
t4364 = -t4359;
t4408 = -t4031.*(t2801-t2850);
t4411 = (t3237.*t4001)./1.0e+8;
t4433 = t12.*t4428;
t4442 = t12.*t4436;
t4444 = t3237.*t4001.*5.7e-7;
t4445 = t3237.*t4001.*1.02e-6;
t4446 = t3237.*t4001.*2.4e-7;
t4447 = t3237.*t4001.*4.0e-8;
t4555 = t3508+t3997;
t4566 = -t4565;
t4568 = -t4567;
t4569 = (t3547.*t4001)./1.0e+8;
t4582 = t3237.*t4265.*9.3e-7;
t4590 = t3237.*t4265.*9.0e-8;
t4600 = -t4596;
t4601 = t12.*t4591;
t4607 = t21.*t4591;
t4610 = -t4605;
t4611 = -t4606;
t4617 = t12.*t4606;
t4619 = t3547.*t4001.*5.7e-7;
t4620 = -t4612;
t4621 = t3547.*t4001.*1.02e-6;
t4622 = -t4614;
t4624 = -t4615;
t4627 = -t4618;
t4629 = t3550.*t4001.*5.7e-7;
t4630 = t21.*t4606;
t4631 = -t4623;
t4632 = t3547.*t4001.*2.4e-7;
t4633 = t3547.*t4001.*4.0e-8;
t4639 = t3550.*t4001.*4.0e-8;
t4640 = -t4634;
t4641 = -t4635;
t4661 = t3711.*t4031;
t4688 = t3814.*t4031;
t4689 = t3815.*t4031;
t4697 = t3547.*t4265.*9.3e-7;
t4698 = t3547.*t4265.*9.0e-8;
t4720 = -t4718;
t4735 = t3893.*t4031;
t4770 = -t4768;
t4771 = -t4769;
t4772 = (t3934.*t4001)./1.0e+8;
t4788 = t12.*t4781;
t4797 = t12.*t4784;
t4800 = -t4794;
t4805 = t12.*t4792;
t4808 = t3934.*t4001.*5.7e-7;
t4809 = t3934.*t4001.*1.02e-6;
t4810 = -t4799;
t4811 = -t4801;
t4813 = -t4803;
t4821 = t3934.*t4001.*2.4e-7;
t4822 = t3937.*t4001.*5.7e-7;
t4823 = t3934.*t4001.*4.0e-8;
t4830 = t3937.*t4001.*4.0e-8;
t4851 = t3236.*t4553.*9.3e-7;
t4852 = t3236.*t4553.*1.02e-6;
t4854 = t3236.*t4553.*9.0e-8;
t4881 = -t4876;
t4888 = t12.*t4883;
t4903 = t12.*t4899;
t4905 = t3991.*t4031.*1.02e-6;
t4906 = t4001.*t4026.*1.02e-6;
t4908 = -t4904;
t4913 = -t4911;
t4914 = -t4912;
t4948 = t4001.*t4151.*5.7e-7;
t4949 = t4001.*t4151.*4.0e-8;
t4957 = t3934.*t4265.*9.3e-7;
t4959 = t3934.*t4265.*9.0e-8;
t4964 = t3543.*t4553.*1.02e-6;
t4965 = t4553.*(t1896-t3239).*(-9.3e-7);
t4966 = t4553.*(t1896-t3239).*(-1.02e-6);
t4968 = t3543.*t4553.*9.0e-8;
t4970 = t4553.*(t1896-t3239).*1.02e-6;
t4971 = t4553.*(t1896-t3239).*(-9.0e-8);
t4976 = t4553.*(t1896-t3239).*9.0e-8;
t4981 = t21.*t4973;
t4983 = t21.*t4979;
t5006 = t4026.*t4265.*9.3e-7;
t5008 = t4026.*t4265.*9.0e-8;
t5021 = -t4291.*(-t2804+t2838+t3109+t17.*(t1456-t2355).*9.3e-7);
t5029 = t3760.*t4573;
t5030 = t3759.*t4577;
t5054 = t3874.*t4573;
t5055 = t3873.*t4577;
t5104 = t5101./2.0;
t5107 = -t5106;
t5109 = t4553.*(t2694-t2701+t3036-t3043).*(-9.3e-7);
t5110 = t4553.*(t2694-t2701+t3036-t3043).*(-1.02e-6);
t5112 = t4553.*(t2694-t2701+t3036-t3043).*1.02e-6;
t5115 = t4553.*(t1959-t3313+t38.*t1022.*(t855-t878).*2.196325630278387e-1).*(-1.02e-6);
t5116 = t4553.*(t2694-t2701+t3036-t3043).*(-9.0e-8);
t5120 = t4553.*(t1959-t3313+t38.*t1022.*(t855-t878).*2.196325630278387e-1).*1.02e-6;
t5121 = t4553.*(t2694-t2701+t3036-t3043).*9.0e-8;
t5122 = t4553.*(t1959-t3313+t38.*t1022.*(t855-t878).*2.196325630278387e-1).*(-9.0e-8);
t5125 = t4553.*(t1959-t3313+t38.*t1022.*(t855-t878).*2.196325630278387e-1).*9.0e-8;
t5147 = t3979.*t4573;
t5148 = t3977.*t4577;
t5153 = t4019.*t4553.*1.02e-6;
t5154 = t4019.*t4553.*9.0e-8;
t5156 = t4553.*(t3242-t3554).*(-9.3e-7);
t5157 = t4553.*(t3242-t3554).*(-1.02e-6);
t5159 = t4553.*(t3242-t3554).*1.02e-6;
t5162 = t4553.*(t3242-t3554).*(-9.0e-8);
t5167 = t4553.*(t3242-t3554).*9.0e-8;
t5206 = t4553.*(t1005+t20.*(t1941-t3315+t39.*t1022.*(t855-t878).*2.196325630278387e-1)).*(-1.02e-6);
t5207 = t4553.*(t1005+t20.*(t1941-t3315+t39.*t1022.*(t855-t878).*2.196325630278387e-1)).*(-9.0e-8);
t5211 = -t5208;
t5216 = -t5212;
t5224 = -t4573.*(-t2804+t2838+t3109+t17.*(t1456-t2355).*9.3e-7);
t5225 = -t4573.*(t2813-t2835+t12.*(t1456-t2355).*1.02e-6+t17.*(t1456-t2355).*9.0e-8);
t5226 = t4163.*t4573;
t5227 = t4160.*t4577;
t5228 = -t4577.*(-t2804+t2838+t3109+t17.*(t1456-t2355).*9.3e-7);
t5229 = t4573.*(-t2804+t2838+t3109+t17.*(t1456-t2355).*9.3e-7);
t5230 = -t4577.*(t2813-t2835+t12.*(t1456-t2355).*1.02e-6+t17.*(t1456-t2355).*9.0e-8);
t5245 = -t5243;
t5270 = -t5266;
t5275 = t3532+t3618+t3630+t3631+t3632;
t5313 = t3231+t3529+t4059+t4060;
t5317 = t3234+t3534+t4063+t4064;
t5323 = -t5322;
t5326 = -t5325;
t5333 = t4001.*t4915.*5.7e-7;
t5334 = -t5330;
t5335 = -t5331;
t5339 = -t5337;
t5341 = t4001.*t4915.*4.0e-8;
t5355 = t3254+t3586+t4121+t4122;
t5369 = t3679+t3743+t3749+t3753+t3754;
t5373 = t3365+t3681+t4179+t4180;
t5376 = -t5374;
t5385 = -t5383;
t5386 = -t5384;
t5388 = -t5387;
t5390 = -t5389;
t5405 = t3259+t4428+t4436;
t5407 = t50.*t189.*(-t4045+t4049+t12.*(t1861-t3221).*1.838876e-2+t17.*(t1861-t3221).*9.99471e-3).*(-9.543032792050485e-17);
t5408 = t50.*t189.*(-t4045+t4049+t12.*(t1861-t3221).*1.838876e-2+t17.*(t1861-t3221).*9.99471e-3).*9.543032792050485e-17;
t5413 = -t2297.*(-t4045+t4049+t12.*(t1861-t3221).*1.838876e-2+t17.*(t1861-t3221).*9.99471e-3);
t5414 = t2297.*(-t4045+t4049+t12.*(t1861-t3221).*1.838876e-2+t17.*(t1861-t3221).*9.99471e-3);
t5421 = t5419./2.0;
t5426 = -t5425;
t5429 = t50.*t202.*(t3566.*1.838876e-2+t4109-t4110+t28.*(t1896-t3239).*9.99471e-3).*(-6.935255936130809e-19);
t5431 = t50.*t202.*(t3566.*1.838876e-2+t4109-t4110+t28.*(t1896-t3239).*9.99471e-3).*6.935255936130809e-19;
t5447 = t2363.*(t3566.*1.838876e-2+t4109-t4110+t28.*(t1896-t3239).*9.99471e-3).*(-7.26735e-3);
t5451 = t5141.*(-t1901+t3122+t3277).*(-1.0./2.0);
t5466 = t628+t665+t675+t676+t1604+t1605+t1607+t1628+t2302+t3283+t3294+t3298+t3624+t3635;
t5469 = t4553.*(t4165+t27.*(t1959-t3313+t38.*t1022.*(t855-t878).*2.196325630278387e-1)).*(-1.02e-6);
t5470 = t4553.*(t4165+t27.*(t1959-t3313+t38.*t1022.*(t855-t878).*2.196325630278387e-1)).*1.02e-6;
t5471 = t4553.*(t4165+t27.*(t1959-t3313+t38.*t1022.*(t855-t878).*2.196325630278387e-1)).*(-9.0e-8);
t5473 = t4553.*(t4165+t27.*(t1959-t3313+t38.*t1022.*(t855-t878).*2.196325630278387e-1)).*9.0e-8;
t5480 = t58+t59+t5465;
t5483 = t429+t5465;
t5502 = t4553.*t4920.*1.02e-6;
t5508 = t4553.*t4920.*9.0e-8;
t5528 = -t5525;
t5529 = -t5526;
t5553 = -t21.*t2363.*(-t3434+t4606+t3980.*(t1896-t3239).*1.02e-6);
t5554 = t21.*t2363.*(-t3434+t4606+t3980.*(t1896-t3239).*1.02e-6).*(-1.0./2.0);
t5557 = t3934.*t4215.*t4712.*5.43845e-3;
t5572 = t4784+t4792;
t5573 = -t3003.*(-t3434+t4606+t3980.*(t1896-t3239).*1.02e-6);
t5574 = t3003.*(-t3434+t4606+t3980.*(t1896-t3239).*1.02e-6).*(-1.0./2.0);
t5579 = -t3055.*(-t3434+t4606+t3980.*(t1896-t3239).*1.02e-6);
t5581 = (t1477-t2502).*(-t3434+t4606+t3980.*(t1896-t3239).*1.02e-6);
t5588 = -t5587;
t5603 = t1205+t1217+t1218+t1230+t2147+t2164+t2166+t2167+t2759+t3405+t3409+t3420+t3739+t3751;
t5632 = -t5631;
t5638 = -t5637;
t5639 = t3278+t3304+t3594+t3626+t4059+t4060;
t5644 = t3282+t3309+t3633+t3636+t4063+t4064;
t5645 = t328+t338+t5594;
t5646 = t351+t363+t5594;
t5651 = t3934.*t4215.*t4950.*5.43845e-3;
t5657 = -t5656;
t5661 = -t5348.*(-t2804+t2838+t3109+t17.*(t1456-t2355).*9.3e-7);
t5665 = t2293+t2304+t3291+t3310+t5273;
t5666 = t2299+t3305+t3612+t3618+t3630+t3631+t3632+t3634;
t5676 = t3332+t3352+t3672+t3677+t4121+t4122;
t5689 = (t3910.*t4172.*t5026)./2.0;
t5691 = t21.*(t1896-t3239).*(-t3434+t4606+t3980.*(t1896-t3239).*1.02e-6);
t5694 = -t21.*t3547.*(-t3434+t4606+t3980.*(t1896-t3239).*1.02e-6);
t5701 = t2398+t3355+t3657+t3661+t3667+t3673+t3674+t3675;
t5702 = t2370+t2494+t3350+t3368+t3583+t3661+t3667+t3674+t3675;
t5718 = -t5717;
t5727 = -t5726;
t5747 = (t3217.*t5610)./2.0;
t5749 = -t5748;
t5752 = t5750./2.0;
t5770 = -t5769;
et126 = -t2306-t2317+t3145+t3148+t35.*t941.*t948.*(t850-t874).*3.775747223193135e-1;
et127 = t36.*t941.*t948.*(t850-t874).*2.244797987218524e-1;
t5786 = t5141.*(et126+et127).*(-1.0./2.0);
t5792 = t3700+t4887+t4899;
t5793 = -t4019.*(-t3434+t4606+t3980.*(t1896-t3239).*1.02e-6);
t5794 = (t3242-t3554).*(-t3434+t4606+t3980.*(t1896-t3239).*1.02e-6);
t5795 = t4019.*(-t3434+t4606+t3980.*(t1896-t3239).*1.02e-6);
t5797 = -t4026.*(-t3434+t4606+t3980.*(t1896-t3239).*1.02e-6);
t5800 = -t4031.*(-t3434+t4606+t3980.*(t1896-t3239).*1.02e-6);
t5801 = t4026.*(-t3434+t4606+t3980.*(t1896-t3239).*1.02e-6);
t5802 = t4031.*(-t3434+t4606+t3980.*(t1896-t3239).*1.02e-6);
t5806 = -t5804;
t5815 = t5814.*(-1.0./2.0);
t5839 = (t3910.*t5610)./2.0;
t5843 = -t5842;
t5854 = -t5853;
t5855 = t70+t76+t90+t91+t2675+t2678+t2690+t2695+t3230+t3527+t3600+t3605+t4046+t4048;
t5876 = (t3500.*t5808)./2.0;
t5904 = t360+t364+t365+t371+t2946+t2951+t2954+t2956+t3358+t3671+t3723+t3734+t4156+t4159;
t5918 = t3066+t3219+t4071+t4090+t4407+t4409;
t5920 = t3934.*t4215.*t5465.*5.43845e-3;
t5929 = (t3915.*t5808)./2.0;
t5961 = -t4872.*(-t3434+t4606+t3980.*(t1896-t3239).*1.02e-6);
t5963 = t4872.*(-t3434+t4606+t3980.*(t1896-t3239).*1.02e-6);
t5964 = (t4165+t27.*(t1959-t3313+t38.*t1022.*(t855-t878).*2.196325630278387e-1)).*(-t3434+t4606+t3980.*(t1896-t3239).*1.02e-6);
t5967 = (-t4045+t4049+t12.*(t1861-t3221).*1.838876e-2+t17.*(t1861-t3221).*9.99471e-3).*(t2694-t2701+t3036-t3043).*(t1513+t1879+t2598+t2820+t2834+t3117+t3118).*(-3.633675e-3);
t5968 = (-t4045+t4049+t12.*(t1861-t3221).*1.838876e-2+t17.*(t1861-t3221).*9.99471e-3).*(t2694-t2701+t3036-t3043).*(t1513+t1879+t2598+t2820+t2834+t3117+t3118).*3.633675e-3;
t5972 = -t4031.*(t3081-t3086+t4086-t4099+t4105+t11.*t3236.*(t1861-t3221).*4.0e-8);
t5973 = t4031.*(t3081-t3086+t4086-t4099+t4105+t11.*t3236.*(t1861-t3221).*4.0e-8);
t5980 = (t4118.*t5808)./2.0;
t5992 = (t3566.*1.33637554986e-4+t4157-t4158+t28.*(t1896-t3239).*7.26350557185e-5).*(t2674-t2676+t3022-t3027).*(t1488+t1874+t2519+t2740+t2747+t3096+t3097).*(-1.0./2.0);
t5993 = ((t3566.*1.33637554986e-4+t4157-t4158+t28.*(t1896-t3239).*7.26350557185e-5).*(t2674-t2676+t3022-t3027).*(t1488+t1874+t2519+t2740+t2747+t3096+t3097))./2.0;
t6012 = t4712.*(t350+t366-t1205+t1210-t1217-t1218-t2147+t2152+t2154+t2155-t3405-t3409-t3420-t3739+t3746+t26.*t50.*t202.*(t46-t47).*8.687615694748404e-39).*(-1.0./2.0);
t6015 = (t4712.*(t350+t366-t1205+t1210-t1217-t1218-t2147+t2152+t2154+t2155-t3405-t3409-t3420-t3739+t3746+t26.*t50.*t202.*(t46-t47).*8.687615694748404e-39))./2.0;
t6020 = (t3910.*t4172.*t5594)./2.0;
t6023 = -t6022;
t6025 = -t6024;
t6047 = t4950.*(t350+t366-t1205+t1210-t1217-t1218-t2147+t2152+t2154+t2155-t3405-t3409-t3420-t3739+t3746+t26.*t50.*t202.*(t46-t47).*8.687615694748404e-39).*(-1.0./2.0);
t6052 = t2363.*t6030;
t6057 = -t6054;
t6067 = -t6066;
t6071 = -t6068;
t6077 = -t6076;
t6081 = -t6080;
t6094 = -t6093;
t6096 = -t6095;
t6101 = t3260+t3271+t4434+t4438+t4443+t4448;
t6113 = -t6030.*(t1896-t3239);
t6114 = t3547.*t6030;
t6115 = (t4879.*t5808)./2.0;
t6119 = -t6118;
t6144 = (t3217.*t6090)./2.0;
t6172 = (t5790.*(t2674-t2676+t3022-t3027).*(t1488+t1874+t2519+t2740+t2747+t3096+t3097))./2.0;
t6212 = -t4031.*(t4533+t4542-t4546-t4550);
t6213 = t4031.*(t4533+t4542-t4546-t4550);
t6217 = t3500.*(t4573.*(t2813-t2835+t12.*(t1456-t2355).*1.02e-6+t17.*(t1456-t2355).*9.0e-8)+t4577.*(-t2804+t2838+t3109+t17.*(t1456-t2355).*9.3e-7)+t3133.*(t3242-t3554)).*(-1.0./2.0);
t6219 = (t11.*(t1861-t3221).*(t4573.*(t2813-t2835+t12.*(t1456-t2355).*1.02e-6+t17.*(t1456-t2355).*9.0e-8)+t4577.*(-t2804+t2838+t3109+t17.*(t1456-t2355).*9.3e-7)+t3133.*(t3242-t3554)))./2.0;
t6227 = t50.*t189.*t6203.*4.771516396025243e-17;
t6232 = t3055.*t6167;
t6241 = (t2297.*t6203)./2.0;
t6270 = (t3047.*t6203)./2.0;
t6272 = (t3910.*t6090)./2.0;
t6279 = t667+t672+t673+t691+t1591+t1602+t1626+t1627+t2301+t2675+t2678+t2690+t2695+t3284+t3287+t3303+t3593+t3600+t3605+t3614+t4046+t4048;
t6301 = (t4673+t2363.*(t3566.*1.838876e-2+t4109-t4110+t28.*(t1896-t3239).*9.99471e-3).*7.26735e-3).*(t2674-t2676+t3022-t3027).*(t1488+t1874+t2519+t2740+t2747+t3096+t3097).*(-1.0./2.0);
t6307 = t3915.*(t4573.*(t2813-t2835+t12.*(t1456-t2355).*1.02e-6+t17.*(t1456-t2355).*9.0e-8)+t4577.*(-t2804+t2838+t3109+t17.*(t1456-t2355).*9.3e-7)+t3133.*(t3242-t3554)).*(-1.0./2.0);
t6324 = t3976.*(t4573.*(t2813-t2835+t12.*(t1456-t2355).*1.02e-6+t17.*(t1456-t2355).*9.0e-8)+t4577.*(-t2804+t2838+t3109+t17.*(t1456-t2355).*9.3e-7)+t3133.*(t3242-t3554)).*(-1.0./2.0);
t6349 = t710+t717+t718+t756+t1690+t1738+t1752+t1753+t2400+t2705+t2711+t2713+t2716+t3335+t3337+t3351+t3641+t3646+t3651+t3659+t4111+t4112;
t6366 = t4118.*(t4573.*(t2813-t2835+t12.*(t1456-t2355).*1.02e-6+t17.*(t1456-t2355).*9.0e-8)+t4577.*(-t2804+t2838+t3109+t17.*(t1456-t2355).*9.3e-7)+t3133.*(t3242-t3554)).*(-1.0./2.0);
t6375 = -t3395.*(t4618+t4634-t12.*t2363.*t3047.*9.0e-8-t17.*t2363.*t3047.*9.3e-7+t12.*t3980.*(t1896-t3239).*9.0e-8+t17.*t3980.*(t1896-t3239).*9.3e-7);
t6377 = t3395.*(t4618+t4634-t12.*t2363.*t3047.*9.0e-8-t17.*t2363.*t3047.*9.3e-7+t12.*t3980.*(t1896-t3239).*9.0e-8+t17.*t3980.*(t1896-t3239).*9.3e-7).*(-1.0./2.0);
t6378 = (t3395.*(t4618+t4634-t12.*t2363.*t3047.*9.0e-8-t17.*t2363.*t3047.*9.3e-7+t12.*t3980.*(t1896-t3239).*9.0e-8+t17.*t3980.*(t1896-t3239).*9.3e-7))./2.0;
t6388 = t4798+t4806+t4812+t4824;
t6401 = t3888+t4684+t4685+t4687+t4731;
t6411 = -t6167.*(t3242-t3554);
t6412 = t4026.*t6167;
et128 = t707+t708-t721-t722-t749+t762+t768-t777-t792-t793-t801-t802-t808+t813-t819+t821-t1629+t1637-t1640-t1641-t1659-t1661+t1666+t1667+t1683+t1692+t1705-t1712+t1758+t1759+t1775+t1776+t1973+t1993+t1994+t2023+t2053+t2060-t2089-t2090+t2098+t2099-t8.*t9.*t15.*t50.*t189.*3.670836568391568e-22;
et129 = t10.*t13.*t14.*t50.*t189.*(-3.279367663374749e-19)-t8.*t9.*t11.*t15.*t50.*t189.*7.075931802640439e-19;
et130 = t8.*t11.*t14.*t15.*t50.*t189.*(-1.190170786299927e-18)-t9.*t11.*t13.*t15.*t50.*t189.*1.190170786299927e-18;
et131 = t13.*t14.*t15.*t16.*t50.*t189.*(-3.226512155691387e-19);
t6438 = t5026.*(et128+et129+et130+et131).*(-1.0./2.0);
t6451 = t3217.*(t3993+t4240-t4332+t4464+t4031.*(t2801-t2850)+t4026.*(t335-t1539-t2831+t2851)).*(-1.0./2.0);
t6484 = t3502.*(t3993+t4240-t4332+t4464+t4031.*(t2801-t2850)+t4026.*(t335-t1539-t2831+t2851)).*(-1.0./2.0);
t6492 = -t6491;
t6508 = t4838.*(t4573.*(t2813-t2835+t12.*(t1456-t2355).*1.02e-6+t17.*(t1456-t2355).*9.0e-8)+t4577.*(-t2804+t2838+t3109+t17.*(t1456-t2355).*9.3e-7)+t3133.*(t3242-t3554)).*(-1.0./2.0);
t6515 = t4879.*(t4573.*(t2813-t2835+t12.*(t1456-t2355).*1.02e-6+t17.*(t1456-t2355).*9.0e-8)+t4577.*(-t2804+t2838+t3109+t17.*(t1456-t2355).*9.3e-7)+t3133.*(t3242-t3554)).*(-1.0./2.0);
t6516 = (t4879.*(t4573.*(t2813-t2835+t12.*(t1456-t2355).*1.02e-6+t17.*(t1456-t2355).*9.0e-8)+t4577.*(-t2804+t2838+t3109+t17.*(t1456-t2355).*9.3e-7)+t3133.*(t3242-t3554)))./2.0;
t6525 = t3910.*(t3993+t4240-t4332+t4464+t4031.*(t2801-t2850)+t4026.*(t335-t1539-t2831+t2851)).*(-1.0./2.0);
t6526 = (t3910.*(t3993+t4240-t4332+t4464+t4031.*(t2801-t2850)+t4026.*(t335-t1539-t2831+t2851)))./2.0;
t6528 = -t6527;
t6560 = -t4577.*(t4618+t4634-t12.*t2363.*t3047.*9.0e-8-t17.*t2363.*t3047.*9.3e-7+t12.*t3980.*(t1896-t3239).*9.0e-8+t17.*t3980.*(t1896-t3239).*9.3e-7);
et132 = t1288+t1289+t1302+t1303-t1319-t1320+t1336-t1348+t1350+t1351-t1360+t1369-t1378+t1396-t1425+t1435-t2174+t2183-t2187+t2193-t2194-t2195+t2199-t2203-t2215+t2219-t2222-t2223+t2239+t2240-t2256-t2257+t2555+t2556+t2572+t2583-t2605-t2606+t2612+t2613-t2618-t2619+t2651+t2652;
et133 = t18.*t19.*t20.*t50.*t202.*(-3.566935413776081e-21);
et134 = t24.*t25.*t26.*t50.*t202.*(-3.992732227073824e-24);
tau_c = ft_12({dq1,dq2,dq3,dq4,dq5,dq6,et132,et133,et134,t10,t1005,t1022,t1089,t11,t1104,t1105,t1108,t1115,t1121,t1158,t1159,t1196,t12,t1205,t1210,t1212,t1217,t1218,t123,t1237,t1238,t1288,t1289,t13,t1302,t1303,t1319,t1320,t1336,t1348,t1350,t1351,t1360,t1369,t1378,t1396,t14,t140,t1425,t1435,t1456,t1477,t1488,t15,t1513,t1539,t1554,t1576,t1577,t1578,t1579,t1584,t1585,t1586,t1587,t1599,t16,t1600,t1604,t1605,t1606,t1607,t1608,t1609,t1613,t1614,t1615,t1616,t1628,t1629,t1631,t1637,t1640,t1641,t1648,t1649,t1659,t1660,t1661,t1666,t1667,t1683,t1686,t1690,t1692,t17,t1700,t1701,t1704,t1705,t1712,t1717,t1741,t1742,t1750,t1754,t1758,t1759,t1775,t1776,t18,t1861,t1874,t1879,t188,t1881,t189,t1896,t19,t1901,t1941,t1959,t1973,t1993,t1994,t20,t201,t202,t2023,t2053,t2060,t2089,t2090,t2098,t2099,t21,t2117,t2120,t2122,t2123,t2137,t2139,t2140,t2147,t2152,t2154,t2155,t2159,t2165,t2174,t2183,t2187,t2193,t2194,t2195,t2199,t22,t2203,t2215,t2219,t2222,t2223,t2239,t2240,t2256,t2257,t2291,t2292,t2294,t2295,t2297,t2302,t2303,t2306,t2307,t2308,t2311,t2317,t2325,t2337,t2338,t2339,t2344,t2355,t236,t2360,t2361,t2362,t2363,t2367,t2368,t237,t2371,t2378,t238,t2388,t2391,t2399,t24,t2401,t2403,t2404,t2405,t241,t2414,t2419,t2421,t2438,t2448,t2449,t2461,t2471,t2472,t2492,t2493,t25,t2502,t2510,t2519,t2527,t2530,t2555,t2556,t2572,t2575,t2583,t2598,t26,t2605,t2606,t2612,t2613,t2618,t2619,t262,t2638,t264,t2651,t2652,t2670,t2671,t2673,t2674,t2676,t2680,t2683,t2684,t2685,t2686,t2687,t2689,t2692,t2693,t2694,t2695,t2696,t2697,t2698,t27,t2700,t2701,t2704,t2707,t2708,t2709,t2712,t2715,t2716,t2717,t2719,t2720,t2721,t2736,t2740,t2747,t2748,t2749,t2754,t2773,t2777,t2778,t2779,t2781,t2787,t2788,t2797,t28,t2801,t2804,t2813,t2814,t2820,t2831,t2834,t2835,t2838,t2850,t2851,t29,t2937,t2942,t2945,t2950,t2953,t2955,t2957,t2965,t2966,t2975,t2979,t2984,t2987,t2990,t2991,t2993,t2994,t2998,t30,t3003,t3004,t3008,t3009,t3015,t3017,t3022,t3027,t3029,t3030,t3036,t3043,t3044,t3045,t3047,t3049,t3054,t3055,t3057,t3058,t3063,t3064,t3068,t3072,t3079,t3080,t3096,t3097,t31,t3109,t3117,t3118,t3121,t3122,t3126,t3129,t313,t3130,t3131,t3132,t3133,t3134,t3135,t3136,t314,t3140,t3141,t3142,t3143,t3145,t3148,t3154,t3156,t3157,t3158,t3159,t3160,t3161,t3162,t3163,t3164,t3165,t3167,t3171,t3172,t3173,t3180,t3181,t3185,t3187,t3188,t3189,t3190,t3192,t3193,t3194,t3195,t3196,t3198,t3199,t32,t3200,t3201,t3202,t3203,t3205,t3206,t3208,t3209,t321,t3211,t3213,t3216,t3217,t3221,t3225,t3232,t3233,t3235,t3236,t3237,t3238,t3239,t3242,t3252,t3253,t3256,t3257,t326,t3261,t3263,t3265,t3266,t3267,t3268,t3269,t3270,t3272,t3273,t3276,t3277,t3279,t3283,t3288,t329,t3290,t3297,t3298,t3299,t33,t3302,t3303,t3307,t331,t3312,t3313,t3314,t3315,t3316,t3318,t332,t3322,t3324,t3326,t3328,t3329,t333,t3334,t3336,t3337,t3338,t3340,t3343,t3344,t3345,t3346,t3347,t335,t3351,t3354,t3357,t3359,t3363,t3364,t3367,t3369,t3370,t3383,t3386,t3387,t3389,t339,t3392,t3394,t3395,t3396,t34,t3405,t3409,t3415,t3416,t3420,t3421,t3423,t3426,t3428,t3430,t3431,t3432,t3433,t3434,t3435,t3438,t3439,t3440,t3441,t3443,t3444,t3445,t3446,t3447,t3448,t3449,t3451,t3452,t3453,t3454,t3455,t3456,t3457,t3458,t346,t3460,t3461,t3462,t3463,t3465,t3467,t3468,t3469,t3471,t3474,t3480,t3482,t3483,t3488,t3489,t3490,t3492,t3495,t3496,t3498,t3499,t35,t350,t3500,t3502,t3503,t3510,t3512,t3517,t3522,t3524,t3531,t3537,t354,t3541,t3543,t3545,t3546,t3547,t3549,t3550,t3551,t3552,t3554,t3558,t356,t3561,t3562,t3563,t3566,t3569,t3577,t3578,t358,t3581,t3582,t3588,t3589,t359,t3590,t3591,t3592,t3597,t3598,t3599,t36,t3603,t3606,t3607,t3608,t3609,t3610,t3611,t3614,t3617,t362,t3621,t3624,t3637,t3638,t3639,t3640,t3641,t3642,t3643,t3644,t3645,t3649,t3652,t3653,t3654,t3655,t3656,t3658,t3659,t366,t3660,t3662,t3664,t3670,t3678,t3684,t3688,t3689,t3690,t3692,t3693,t3695,t3696,t3697,t3699,t3701,t3702,t3703,t3704,t3705,t3706,t3707,t3708,t3709,t3710,t3712,t3713,t3716,t3717,t372,t3722,t3726,t3728,t3729,t3731,t3732,t3735,t3736,t3737,t3738,t3739,t3741,t3746,t3747,t3752,t3755,t3759,t3760,t3765,t3766,t3770,t3771,t3772,t3774,t3775,t3777,t3779,t378,t3781,t3782,t3783,t3784,t3785,t3786,t3788,t3789,t3790,t3791,t3792,t3793,t3794,t3795,t3796,t3797,t3798,t38,t380,t3800,t3801,t3802,t3804,t3805,t3808,t3809,t3810,t3817,t3818,t382,t3820,t3821,t3823,t3824,t3826,t3827,t3828,t3830,t3832,t3833,t3835,t3840,t3843,t3844,t3845,t3846,t3848,t3850,t3851,t3855,t3856,t3857,t3862,t3863,t387,t3873,t3874,t3876,t3877,t3878,t3879,t3880,t3889,t3890,t3891,t3893,t3895,t3896,t3897,t3898,t39,t3901,t3902,t3903,t3906,t3908,t3909,t3910,t3913,t3915,t3924,t3925,t3926,t3931,t3934,t3937,t3943,t3949,t3951,t3961,t3967,t3968,t3974,t3975,t3976,t3977,t3979,t3980,t3983,t3985,t3988,t3991,t3992,t3993,t3996,t3998,t3999,t4001,t4002,t4006,t4007,t4008,t4010,t4014,t4018,t4019,t4026,t4030,t4031,t4032,t4035,t4039,t4041,t4045,t4047,t4049,t4050,t4051,t4052,t4053,t4054,t4056,t4065,t410,t4100,t4109,t4110,t4113,t4114,t4115,t4118,t4144,t4146,t4147,t4151,t4153,t4154,t4157,t4158,t4160,t4163,t4165,t4168,t4171,t4172,t4187,t4188,t4190,t4193,t4198,t42,t4201,t4205,t4207,t4208,t4213,t4215,t4218,t4219,t4224,t4229,t4230,t4236,t4240,t4241,t4243,t4244,t4246,t4248,t4249,t4258,t4260,t4261,t4263,t4267,t4270,t4272,t4273,t4274,t4275,t4276,t4277,t4278,t4279,t4280,t4281,t4282,t4283,t4286,t4287,t4288,t4289,t429,t4290,t4291,t4292,t4293,t4294,t4295,t4296,t4297,t4298,t4299,t43,t4300,t4301,t4303,t4304,t4305,t4306,t4307,t4308,t4310,t4311,t4312,t4313,t4314,t4318,t4319,t4321,t4324,t4325,t4326,t4330,t4332,t4334,t4337,t4339,t4341,t4342,t4343,t4344,t4345,t4346,t4352,t4354,t4355,t4356,t4358,t4359,t4361,t4362,t4363,t4364,t4371,t4372,t4373,t4375,t4404,t4406,t4408,t4411,t4413,t4415,t4416,t4417,t4422,t4423,t4426,t4427,t4429,t4430,t4431,t4432,t4433,t4435,t4439,t4440,t4441,t4442,t4444,t4445,t4446,t4447,t4449,t4457,t4458,t4459,t4461,t4464,t4465,t4466,t4467,t4468,t4470,t4476,t4479,t4482,t4486,t4488,t4489,t4491,t4493,t4494,t4495,t4496,t4497,t4501,t4502,t4504,t4515,t4517,t4518,t4520,t4522,t4523,t4532,t4534,t4537,t4545,t4553,t4559,t4561,t4562,t4563,t4564,t4566,t4567,t4568,t4569,t4570,t4571,t4573,t4574,t4576,t4577,t4578,t4579,t4580,t4582,t4583,t4584,t4585,t4588,t4589,t4590,t4591,t4593,t4594,t4595,t4598,t4599,t46,t4600,t4601,t4602,t4606,t4608,t4609,t4610,t4611,t4613,t4615,t4617,t4618,t4619,t4620,t4621,t4622,t4623,t4624,t4625,t4626,t4627,t4629,t4630,t4631,t4632,t4633,t4634,t4635,t4639,t4640,t4641,t4643,t4644,t4645,t4646,t4647,t4649,t4650,t4651,t4652,t4654,t4656,t4657,t4658,t4660,t4661,t4663,t4665,t4667,t4669,t4670,t4672,t4673,t4674,t4675,t4676,t4677,t4678,t4680,t4683,t4686,t4688,t4689,t4690,t4691,t4692,t4694,t4696,t4697,t4698,t47,t4703,t4704,t4705,t4708,t4709,t4711,t4712,t4713,t4716,t4719,t4720,t4722,t4724,t4725,t4727,t4728,t4730,t4733,t4735,t4737,t4739,t4741,t4743,t4744,t4746,t4751,t4757,t4760,t4761,t4762,t4763,t4764,t4766,t4767,t4770,t4771,t4772,t4774,t4776,t4777,t4778,t4779,t4783,t4785,t4786,t4787,t4790,t4791,t4793,t4795,t4796,t4797,t4799,t4800,t4801,t4805,t4808,t4809,t4810,t4811,t4813,t4814,t4815,t4816,t4818,t4821,t4822,t4823,t4825,t4826,t4828,t4830,t4833,t4835,t4838,t4843,t4844,t4845,t4846,t4847,t4848,t4849,t4850,t4851,t4852,t4853,t4854,t4856,t4857,t4858,t4859,t4863,t4867,t4872,t4874,t4875,t4876,t4879,t4880,t4881,t4886,t4887,t4888,t4889,t4892,t4893,t4895,t4896,t4898,t4901,t4902,t4903,t4904,t4905,t4906,t4907,t4908,t4911,t4912,t4913,t4914,t4915,t4918,t4919,t4920,t4921,t4922,t4923,t4924,t4925,t4926,t4927,t4928,t4929,t4930,t4933,t4934,t4935,t4936,t4937,t4938,t4939,t4940,t4941,t4943,t4945,t4946,t4947,t4948,t4949,t4950,t4952,t4953,t4955,t4957,t4958,t4959,t4964,t4965,t4966,t4968,t4969,t4970,t4971,t4973,t4974,t4976,t4977,t4979,t4981,t4983,t50,t5001,t5003,t5004,t5005,t5006,t5008,t5012,t5013,t5014,t5016,t5019,t5020,t5021,t5024,t5025,t5026,t5027,t5028,t5029,t5030,t5033,t5034,t5035,t5036,t5037,t5038,t5041,t5042,t5043,t5045,t5046,t5047,t5049,t5051,t5052,t5053,t5054,t5055,t5059,t5061,t5062,t5063,t5064,t5066,t5070,t5071,t5072,t5074,t5075,t5076,t5077,t5079,t5080,t5081,t5082,t5083,t5084,t5085,t5086,t5087,t5088,t5089,t5090,t5091,t5093,t5096,t5097,t5098,t5100,t5101,t5103,t5104,t5106,t5108,t5109,t5111,t5112,t5113,t5114,t5116,t5117,t5118,t5119,t5120,t5121,t5123,t5124,t5125,t5126,t5127,t5141,t5142,t5144,t5146,t5147,t5148,t5153,t5154,t5155,t5156,t5158,t5159,t5161,t5162,t5163,t5164,t5165,t5166,t5167,t5168,t5169,t5171,t5173,t5174,t5176,t5177,t5178,t5180,t5181,t5194,t5195,t5196,t5197,t5198,t5199,t5200,t5201,t5202,t5203,t5205,t5206,t5207,t5208,t5211,t5212,t5213,t5214,t5215,t5216,t5219,t5225,t5226,t5227,t5228,t5229,t5230,t5234,t5240,t5241,t5243,t5244,t5245,t5246,t5247,t5248,t5249,t5251,t5254,t5255,t5256,t5257,t5258,t5259,t5261,t5262,t5263,t5264,t5265,t5267,t5268,t5269,t5270,t5271,t5272,t5274,t5275,t5276,t5277,t5278,t5279,t5280,t5281,t5283,t5284,t5285,t5286,t5287,t5288,t5289,t5290,t5291,t5292,t5293,t5294,t5295,t5296,t5297,t5298,t5300,t5301,t5302,t5303,t5304,t5305,t5306,t5308,t5309,t5310,t5312,t5313,t5315,t5316,t5317,t5323,t5324,t5325,t5326,t5327,t5328,t5329,t5330,t5331,t5332,t5333,t5334,t5335,t5336,t5337,t5339,t5340,t5341,t5343,t5344,t5345,t5346,t5348,t5350,t5352,t5353,t5355,t5356,t5357,t5358,t5359,t5361,t5362,t5363,t5369,t5370,t5372,t5373,t5374,t5376,t5381,t5383,t5384,t5385,t5386,t5387,t5389,t5390,t5391,t5392,t5393,t5395,t5399,t5400,t5401,t5402,t5403,t5404,t5405,t5408,t5410,t5411,t5412,t5413,t5414,t5415,t5416,t5419,t5421,t5424,t5425,t5426,t5431,t5433,t5434,t5436,t5437,t5438,t5439,t5440,t5441,t5442,t5443,t5444,t5445,t5446,t5447,t5448,t5449,t5451,t5452,t5456,t5457,t5458,t5459,t5460,t5461,t5462,t5464,t5465,t5466,t5470,t5472,t5473,t5474,t5480,t5481,t5483,t5487,t5488,t5494,t5495,t5499,t5500,t5501,t5502,t5503,t5504,t5506,t5507,t5508,t5509,t5510,t5512,t5513,t5514,t5516,t5517,t5520,t5522,t5523,t5524,t5527,t5528,t5529,t5531,t5532,t5535,t5536,t5537,t5538,t5539,t5540,t5541,t5542,t5543,t5544,t5545,t5548,t5549,t5550,t5553,t5554,t5555,t5556,t5557,t5560,t5565,t5567,t5568,t5569,t5570,t5572,t5573,t5574,t5575,t5576,t5577,t5578,t5579,t5581,t5586,t5587,t5588,t5589,t5590,t5591,t5592,t5593,t5594,t5596,t5597,t5598,t5599,t56,t5600,t5601,t5602,t5603,t5604,t5605,t5606,t5607,t5608,t5609,t5611,t5612,t5613,t5614,t5615,t5616,t5619,t5623,t5624,t5625,t5629,t5630,t5631,t5632,t5633,t5634,t5635,t5636,t5637,t5638,t5639,t5644,t5645,t5646,t5649,t5650,t5651,t5653,t5654,t5655,t5657,t5658,t5659,t5660,t5661,t5662,t5663,t5666,t5675,t5676,t5677,t5678,t5679,t5680,t5684,t5689,t5691,t5694,t5698,t5699,t5701,t5702,t5717,t5718,t5719,t5720,t5721,t5722,t5724,t5725,t5727,t5730,t5731,t5734,t5735,t5736,t5738,t5739,t5741,t5742,t5745,t5747,t5749,t5750,t5751,t5752,t5757,t5758,t5759,t5760,t5761,t5763,t5764,t5765,t5766,t5768,t5769,t5770,t5775,t5776,t5777,t5778,t5779,t5781,t5782,t5783,t5784,t5787,t5788,t5790,t5792,t5793,t5794,t5795,t58,t5801,t5802,t5804,t5805,t5806,t5813,t5814,t5821,t5822,t5823,t5824,t5825,t5835,t5836,t5839,t5842,t5849,t5851,t5852,t5853,t5855,t5863,t5864,t5865,t5866,t5876,t5885,t5886,t5887,t5891,t5892,t5896,t59,t5901,t5902,t5904,t5908,t5909,t5916,t5917,t5918,t5919,t5920,t5922,t5924,t5925,t5928,t5929,t5930,t5933,t5938,t5941,t5954,t5955,t5959,t5960,t5963,t5964,t5966,t5967,t5968,t5971,t5973,t5978,t5979,t5980,t5990,t5992,t5993,t60,t6002,t6004,t6005,t6011,t6013,t6014,t6015,t6019,t6020,t6022,t6023,t6024,t6031,t6047,t6048,t6050,t6052,t6054,t6056,t6057,t6059,t6062,t6066,t6067,t6069,t6070,t6071,t6072,t6074,t6076,t6079,t6080,t6081,t6091,t6093,t6094,t6095,t6096,t6101,t6113,t6114,t6115,t6119,t6123,t6125,t6126,t6127,t6129,t6131,t6133,t6134,t6143,t6144,t6154,t6158,t6162,t6164,t6166,t6168,t6172,t6183,t6211,t6213,t6217,t6219,t6221,t6222,t6227,t6232,t6241,t6255,t6256,t6257,t6270,t6271,t6272,t6307,t6324,t6366,t6375,t6377,t638,t6388,t6394,t6396,t6398,t640,t6411,t6412,t642,t6425,t643,t6438,t6440,t6442,t6460,t6461,t6482,t6483,t6484,t649,t6491,t6508,t6515,t6517,t6523,t6524,t6525,t6526,t6527,t6528,t654,t655,t656,t6560,t6564,t6565,t657,t6574,t6581,t6588,t6589,t659,t6594,t660,t6602,t6622,t6623,t6651,t6661,t6662,t667,t668,t6680,t669,t67,t670,t674,t6745,t6751,t677,t68,t681,t682,t684,t685,t686,t687,t6919,t692,t6920,t693,t694,t6965,t6966,t6987,t7003,t7005,t7007,t7014,t702,t7035,t707,t708,t7086,t7088,t7093,t7094,t7096,t71,t710,t7134,t7135,t7137,t7138,t7148,t715,t7150,t7153,t7154,t7158,t716,t7160,t7167,t7199,t721,t722,t724,t725,t73,t7304,t7319,t7331,t7332,t7333,t7334,t736,t738,t740,t741,t749,t762,t768,t777,t792,t793,t8,t801,t802,t808,t813,t819,t821,t850,t855,t874,t878,t89,t9,t92,t941,t948,t951,t97});
end
function tau_c = ft_12(ct)
dq1 = ct{1};
dq2 = ct{2};
dq3 = ct{3};
dq4 = ct{4};
dq5 = ct{5};
dq6 = ct{6};
et132 = ct{7};
et133 = ct{8};
et134 = ct{9};
t10 = ct{10};
t1005 = ct{11};
t1022 = ct{12};
t1089 = ct{13};
t11 = ct{14};
t1104 = ct{15};
t1105 = ct{16};
t1108 = ct{17};
t1115 = ct{18};
t1121 = ct{19};
t1158 = ct{20};
t1159 = ct{21};
t1196 = ct{22};
t12 = ct{23};
t1205 = ct{24};
t1210 = ct{25};
t1212 = ct{26};
t1217 = ct{27};
t1218 = ct{28};
t123 = ct{29};
t1237 = ct{30};
t1238 = ct{31};
t1288 = ct{32};
t1289 = ct{33};
t13 = ct{34};
t1302 = ct{35};
t1303 = ct{36};
t1319 = ct{37};
t1320 = ct{38};
t1336 = ct{39};
t1348 = ct{40};
t1350 = ct{41};
t1351 = ct{42};
t1360 = ct{43};
t1369 = ct{44};
t1378 = ct{45};
t1396 = ct{46};
t14 = ct{47};
t140 = ct{48};
t1425 = ct{49};
t1435 = ct{50};
t1456 = ct{51};
t1477 = ct{52};
t1488 = ct{53};
t15 = ct{54};
t1513 = ct{55};
t1539 = ct{56};
t1554 = ct{57};
t1576 = ct{58};
t1577 = ct{59};
t1578 = ct{60};
t1579 = ct{61};
t1584 = ct{62};
t1585 = ct{63};
t1586 = ct{64};
t1587 = ct{65};
t1599 = ct{66};
t16 = ct{67};
t1600 = ct{68};
t1604 = ct{69};
t1605 = ct{70};
t1606 = ct{71};
t1607 = ct{72};
t1608 = ct{73};
t1609 = ct{74};
t1613 = ct{75};
t1614 = ct{76};
t1615 = ct{77};
t1616 = ct{78};
t1628 = ct{79};
t1629 = ct{80};
t1631 = ct{81};
t1637 = ct{82};
t1640 = ct{83};
t1641 = ct{84};
t1648 = ct{85};
t1649 = ct{86};
t1659 = ct{87};
t1660 = ct{88};
t1661 = ct{89};
t1666 = ct{90};
t1667 = ct{91};
t1683 = ct{92};
t1686 = ct{93};
t1690 = ct{94};
t1692 = ct{95};
t17 = ct{96};
t1700 = ct{97};
t1701 = ct{98};
t1704 = ct{99};
t1705 = ct{100};
t1712 = ct{101};
t1717 = ct{102};
t1741 = ct{103};
t1742 = ct{104};
t1750 = ct{105};
t1754 = ct{106};
t1758 = ct{107};
t1759 = ct{108};
t1775 = ct{109};
t1776 = ct{110};
t18 = ct{111};
t1861 = ct{112};
t1874 = ct{113};
t1879 = ct{114};
t188 = ct{115};
t1881 = ct{116};
t189 = ct{117};
t1896 = ct{118};
t19 = ct{119};
t1901 = ct{120};
t1941 = ct{121};
t1959 = ct{122};
t1973 = ct{123};
t1993 = ct{124};
t1994 = ct{125};
t20 = ct{126};
t201 = ct{127};
t202 = ct{128};
t2023 = ct{129};
t2053 = ct{130};
t2060 = ct{131};
t2089 = ct{132};
t2090 = ct{133};
t2098 = ct{134};
t2099 = ct{135};
t21 = ct{136};
t2117 = ct{137};
t2120 = ct{138};
t2122 = ct{139};
t2123 = ct{140};
t2137 = ct{141};
t2139 = ct{142};
t2140 = ct{143};
t2147 = ct{144};
t2152 = ct{145};
t2154 = ct{146};
t2155 = ct{147};
t2159 = ct{148};
t2165 = ct{149};
t2174 = ct{150};
t2183 = ct{151};
t2187 = ct{152};
t2193 = ct{153};
t2194 = ct{154};
t2195 = ct{155};
t2199 = ct{156};
t22 = ct{157};
t2203 = ct{158};
t2215 = ct{159};
t2219 = ct{160};
t2222 = ct{161};
t2223 = ct{162};
t2239 = ct{163};
t2240 = ct{164};
t2256 = ct{165};
t2257 = ct{166};
t2291 = ct{167};
t2292 = ct{168};
t2294 = ct{169};
t2295 = ct{170};
t2297 = ct{171};
t2302 = ct{172};
t2303 = ct{173};
t2306 = ct{174};
t2307 = ct{175};
t2308 = ct{176};
t2311 = ct{177};
t2317 = ct{178};
t2325 = ct{179};
t2337 = ct{180};
t2338 = ct{181};
t2339 = ct{182};
t2344 = ct{183};
t2355 = ct{184};
t236 = ct{185};
t2360 = ct{186};
t2361 = ct{187};
t2362 = ct{188};
t2363 = ct{189};
t2367 = ct{190};
t2368 = ct{191};
t237 = ct{192};
t2371 = ct{193};
t2378 = ct{194};
t238 = ct{195};
t2388 = ct{196};
t2391 = ct{197};
t2399 = ct{198};
t24 = ct{199};
t2401 = ct{200};
t2403 = ct{201};
t2404 = ct{202};
t2405 = ct{203};
t241 = ct{204};
t2414 = ct{205};
t2419 = ct{206};
t2421 = ct{207};
t2438 = ct{208};
t2448 = ct{209};
t2449 = ct{210};
t2461 = ct{211};
t2471 = ct{212};
t2472 = ct{213};
t2492 = ct{214};
t2493 = ct{215};
t25 = ct{216};
t2502 = ct{217};
t2510 = ct{218};
t2519 = ct{219};
t2527 = ct{220};
t2530 = ct{221};
t2555 = ct{222};
t2556 = ct{223};
t2572 = ct{224};
t2575 = ct{225};
t2583 = ct{226};
t2598 = ct{227};
t26 = ct{228};
t2605 = ct{229};
t2606 = ct{230};
t2612 = ct{231};
t2613 = ct{232};
t2618 = ct{233};
t2619 = ct{234};
t262 = ct{235};
t2638 = ct{236};
t264 = ct{237};
t2651 = ct{238};
t2652 = ct{239};
t2670 = ct{240};
t2671 = ct{241};
t2673 = ct{242};
t2674 = ct{243};
t2676 = ct{244};
t2680 = ct{245};
t2683 = ct{246};
t2684 = ct{247};
t2685 = ct{248};
t2686 = ct{249};
t2687 = ct{250};
t2689 = ct{251};
t2692 = ct{252};
t2693 = ct{253};
t2694 = ct{254};
t2695 = ct{255};
t2696 = ct{256};
t2697 = ct{257};
t2698 = ct{258};
t27 = ct{259};
t2700 = ct{260};
t2701 = ct{261};
t2704 = ct{262};
t2707 = ct{263};
t2708 = ct{264};
t2709 = ct{265};
t2712 = ct{266};
t2715 = ct{267};
t2716 = ct{268};
t2717 = ct{269};
t2719 = ct{270};
t2720 = ct{271};
t2721 = ct{272};
t2736 = ct{273};
t2740 = ct{274};
t2747 = ct{275};
t2748 = ct{276};
t2749 = ct{277};
t2754 = ct{278};
t2773 = ct{279};
t2777 = ct{280};
t2778 = ct{281};
t2779 = ct{282};
t2781 = ct{283};
t2787 = ct{284};
t2788 = ct{285};
t2797 = ct{286};
t28 = ct{287};
t2801 = ct{288};
t2804 = ct{289};
t2813 = ct{290};
t2814 = ct{291};
t2820 = ct{292};
t2831 = ct{293};
t2834 = ct{294};
t2835 = ct{295};
t2838 = ct{296};
t2850 = ct{297};
t2851 = ct{298};
t29 = ct{299};
t2937 = ct{300};
t2942 = ct{301};
t2945 = ct{302};
t2950 = ct{303};
t2953 = ct{304};
t2955 = ct{305};
t2957 = ct{306};
t2965 = ct{307};
t2966 = ct{308};
t2975 = ct{309};
t2979 = ct{310};
t2984 = ct{311};
t2987 = ct{312};
t2990 = ct{313};
t2991 = ct{314};
t2993 = ct{315};
t2994 = ct{316};
t2998 = ct{317};
t30 = ct{318};
t3003 = ct{319};
t3004 = ct{320};
t3008 = ct{321};
t3009 = ct{322};
t3015 = ct{323};
t3017 = ct{324};
t3022 = ct{325};
t3027 = ct{326};
t3029 = ct{327};
t3030 = ct{328};
t3036 = ct{329};
t3043 = ct{330};
t3044 = ct{331};
t3045 = ct{332};
t3047 = ct{333};
t3049 = ct{334};
t3054 = ct{335};
t3055 = ct{336};
t3057 = ct{337};
t3058 = ct{338};
t3063 = ct{339};
t3064 = ct{340};
t3068 = ct{341};
t3072 = ct{342};
t3079 = ct{343};
t3080 = ct{344};
t3096 = ct{345};
t3097 = ct{346};
t31 = ct{347};
t3109 = ct{348};
t3117 = ct{349};
t3118 = ct{350};
t3121 = ct{351};
t3122 = ct{352};
t3126 = ct{353};
t3129 = ct{354};
t313 = ct{355};
t3130 = ct{356};
t3131 = ct{357};
t3132 = ct{358};
t3133 = ct{359};
t3134 = ct{360};
t3135 = ct{361};
t3136 = ct{362};
t314 = ct{363};
t3140 = ct{364};
t3141 = ct{365};
t3142 = ct{366};
t3143 = ct{367};
t3145 = ct{368};
t3148 = ct{369};
t3154 = ct{370};
t3156 = ct{371};
t3157 = ct{372};
t3158 = ct{373};
t3159 = ct{374};
t3160 = ct{375};
t3161 = ct{376};
t3162 = ct{377};
t3163 = ct{378};
t3164 = ct{379};
t3165 = ct{380};
t3167 = ct{381};
t3171 = ct{382};
t3172 = ct{383};
t3173 = ct{384};
t3180 = ct{385};
t3181 = ct{386};
t3185 = ct{387};
t3187 = ct{388};
t3188 = ct{389};
t3189 = ct{390};
t3190 = ct{391};
t3192 = ct{392};
t3193 = ct{393};
t3194 = ct{394};
t3195 = ct{395};
t3196 = ct{396};
t3198 = ct{397};
t3199 = ct{398};
t32 = ct{399};
t3200 = ct{400};
t3201 = ct{401};
t3202 = ct{402};
t3203 = ct{403};
t3205 = ct{404};
t3206 = ct{405};
t3208 = ct{406};
t3209 = ct{407};
t321 = ct{408};
t3211 = ct{409};
t3213 = ct{410};
t3216 = ct{411};
t3217 = ct{412};
t3221 = ct{413};
t3225 = ct{414};
t3232 = ct{415};
t3233 = ct{416};
t3235 = ct{417};
t3236 = ct{418};
t3237 = ct{419};
t3238 = ct{420};
t3239 = ct{421};
t3242 = ct{422};
t3252 = ct{423};
t3253 = ct{424};
t3256 = ct{425};
t3257 = ct{426};
t326 = ct{427};
t3261 = ct{428};
t3263 = ct{429};
t3265 = ct{430};
t3266 = ct{431};
t3267 = ct{432};
t3268 = ct{433};
t3269 = ct{434};
t3270 = ct{435};
t3272 = ct{436};
t3273 = ct{437};
t3276 = ct{438};
t3277 = ct{439};
t3279 = ct{440};
t3283 = ct{441};
t3288 = ct{442};
t329 = ct{443};
t3290 = ct{444};
t3297 = ct{445};
t3298 = ct{446};
t3299 = ct{447};
t33 = ct{448};
t3302 = ct{449};
t3303 = ct{450};
t3307 = ct{451};
t331 = ct{452};
t3312 = ct{453};
t3313 = ct{454};
t3314 = ct{455};
t3315 = ct{456};
t3316 = ct{457};
t3318 = ct{458};
t332 = ct{459};
t3322 = ct{460};
t3324 = ct{461};
t3326 = ct{462};
t3328 = ct{463};
t3329 = ct{464};
t333 = ct{465};
t3334 = ct{466};
t3336 = ct{467};
t3337 = ct{468};
t3338 = ct{469};
t3340 = ct{470};
t3343 = ct{471};
t3344 = ct{472};
t3345 = ct{473};
t3346 = ct{474};
t3347 = ct{475};
t335 = ct{476};
t3351 = ct{477};
t3354 = ct{478};
t3357 = ct{479};
t3359 = ct{480};
t3363 = ct{481};
t3364 = ct{482};
t3367 = ct{483};
t3369 = ct{484};
t3370 = ct{485};
t3383 = ct{486};
t3386 = ct{487};
t3387 = ct{488};
t3389 = ct{489};
t339 = ct{490};
t3392 = ct{491};
t3394 = ct{492};
t3395 = ct{493};
t3396 = ct{494};
t34 = ct{495};
t3405 = ct{496};
t3409 = ct{497};
t3415 = ct{498};
t3416 = ct{499};
t3420 = ct{500};
t3421 = ct{501};
t3423 = ct{502};
t3426 = ct{503};
t3428 = ct{504};
t3430 = ct{505};
t3431 = ct{506};
t3432 = ct{507};
t3433 = ct{508};
t3434 = ct{509};
t3435 = ct{510};
t3438 = ct{511};
t3439 = ct{512};
t3440 = ct{513};
t3441 = ct{514};
t3443 = ct{515};
t3444 = ct{516};
t3445 = ct{517};
t3446 = ct{518};
t3447 = ct{519};
t3448 = ct{520};
t3449 = ct{521};
t3451 = ct{522};
t3452 = ct{523};
t3453 = ct{524};
t3454 = ct{525};
t3455 = ct{526};
t3456 = ct{527};
t3457 = ct{528};
t3458 = ct{529};
t346 = ct{530};
t3460 = ct{531};
t3461 = ct{532};
t3462 = ct{533};
t3463 = ct{534};
t3465 = ct{535};
t3467 = ct{536};
t3468 = ct{537};
t3469 = ct{538};
t3471 = ct{539};
t3474 = ct{540};
t3480 = ct{541};
t3482 = ct{542};
t3483 = ct{543};
t3488 = ct{544};
t3489 = ct{545};
t3490 = ct{546};
t3492 = ct{547};
t3495 = ct{548};
t3496 = ct{549};
t3498 = ct{550};
t3499 = ct{551};
t35 = ct{552};
t350 = ct{553};
t3500 = ct{554};
t3502 = ct{555};
t3503 = ct{556};
t3510 = ct{557};
t3512 = ct{558};
t3517 = ct{559};
t3522 = ct{560};
t3524 = ct{561};
t3531 = ct{562};
t3537 = ct{563};
t354 = ct{564};
t3541 = ct{565};
t3543 = ct{566};
t3545 = ct{567};
t3546 = ct{568};
t3547 = ct{569};
t3549 = ct{570};
t3550 = ct{571};
t3551 = ct{572};
t3552 = ct{573};
t3554 = ct{574};
t3558 = ct{575};
t356 = ct{576};
t3561 = ct{577};
t3562 = ct{578};
t3563 = ct{579};
t3566 = ct{580};
t3569 = ct{581};
t3577 = ct{582};
t3578 = ct{583};
t358 = ct{584};
t3581 = ct{585};
t3582 = ct{586};
t3588 = ct{587};
t3589 = ct{588};
t359 = ct{589};
t3590 = ct{590};
t3591 = ct{591};
t3592 = ct{592};
t3597 = ct{593};
t3598 = ct{594};
t3599 = ct{595};
t36 = ct{596};
t3603 = ct{597};
t3606 = ct{598};
t3607 = ct{599};
t3608 = ct{600};
t3609 = ct{601};
t3610 = ct{602};
t3611 = ct{603};
t3614 = ct{604};
t3617 = ct{605};
t362 = ct{606};
t3621 = ct{607};
t3624 = ct{608};
t3637 = ct{609};
t3638 = ct{610};
t3639 = ct{611};
t3640 = ct{612};
t3641 = ct{613};
t3642 = ct{614};
t3643 = ct{615};
t3644 = ct{616};
t3645 = ct{617};
t3649 = ct{618};
t3652 = ct{619};
t3653 = ct{620};
t3654 = ct{621};
t3655 = ct{622};
t3656 = ct{623};
t3658 = ct{624};
t3659 = ct{625};
t366 = ct{626};
t3660 = ct{627};
t3662 = ct{628};
t3664 = ct{629};
t3670 = ct{630};
t3678 = ct{631};
t3684 = ct{632};
t3688 = ct{633};
t3689 = ct{634};
t3690 = ct{635};
t3692 = ct{636};
t3693 = ct{637};
t3695 = ct{638};
t3696 = ct{639};
t3697 = ct{640};
t3699 = ct{641};
t3701 = ct{642};
t3702 = ct{643};
t3703 = ct{644};
t3704 = ct{645};
t3705 = ct{646};
t3706 = ct{647};
t3707 = ct{648};
t3708 = ct{649};
t3709 = ct{650};
t3710 = ct{651};
t3712 = ct{652};
t3713 = ct{653};
t3716 = ct{654};
t3717 = ct{655};
t372 = ct{656};
t3722 = ct{657};
t3726 = ct{658};
t3728 = ct{659};
t3729 = ct{660};
t3731 = ct{661};
t3732 = ct{662};
t3735 = ct{663};
t3736 = ct{664};
t3737 = ct{665};
t3738 = ct{666};
t3739 = ct{667};
t3741 = ct{668};
t3746 = ct{669};
t3747 = ct{670};
t3752 = ct{671};
t3755 = ct{672};
t3759 = ct{673};
t3760 = ct{674};
t3765 = ct{675};
t3766 = ct{676};
t3770 = ct{677};
t3771 = ct{678};
t3772 = ct{679};
t3774 = ct{680};
t3775 = ct{681};
t3777 = ct{682};
t3779 = ct{683};
t378 = ct{684};
t3781 = ct{685};
t3782 = ct{686};
t3783 = ct{687};
t3784 = ct{688};
t3785 = ct{689};
t3786 = ct{690};
t3788 = ct{691};
t3789 = ct{692};
t3790 = ct{693};
t3791 = ct{694};
t3792 = ct{695};
t3793 = ct{696};
t3794 = ct{697};
t3795 = ct{698};
t3796 = ct{699};
t3797 = ct{700};
t3798 = ct{701};
t38 = ct{702};
t380 = ct{703};
t3800 = ct{704};
t3801 = ct{705};
t3802 = ct{706};
t3804 = ct{707};
t3805 = ct{708};
t3808 = ct{709};
t3809 = ct{710};
t3810 = ct{711};
t3817 = ct{712};
t3818 = ct{713};
t382 = ct{714};
t3820 = ct{715};
t3821 = ct{716};
t3823 = ct{717};
t3824 = ct{718};
t3826 = ct{719};
t3827 = ct{720};
t3828 = ct{721};
t3830 = ct{722};
t3832 = ct{723};
t3833 = ct{724};
t3835 = ct{725};
t3840 = ct{726};
t3843 = ct{727};
t3844 = ct{728};
t3845 = ct{729};
t3846 = ct{730};
t3848 = ct{731};
t3850 = ct{732};
t3851 = ct{733};
t3855 = ct{734};
t3856 = ct{735};
t3857 = ct{736};
t3862 = ct{737};
t3863 = ct{738};
t387 = ct{739};
t3873 = ct{740};
t3874 = ct{741};
t3876 = ct{742};
t3877 = ct{743};
t3878 = ct{744};
t3879 = ct{745};
t3880 = ct{746};
t3889 = ct{747};
t3890 = ct{748};
t3891 = ct{749};
t3893 = ct{750};
t3895 = ct{751};
t3896 = ct{752};
t3897 = ct{753};
t3898 = ct{754};
t39 = ct{755};
t3901 = ct{756};
t3902 = ct{757};
t3903 = ct{758};
t3906 = ct{759};
t3908 = ct{760};
t3909 = ct{761};
t3910 = ct{762};
t3913 = ct{763};
t3915 = ct{764};
t3924 = ct{765};
t3925 = ct{766};
t3926 = ct{767};
t3931 = ct{768};
t3934 = ct{769};
t3937 = ct{770};
t3943 = ct{771};
t3949 = ct{772};
t3951 = ct{773};
t3961 = ct{774};
t3967 = ct{775};
t3968 = ct{776};
t3974 = ct{777};
t3975 = ct{778};
t3976 = ct{779};
t3977 = ct{780};
t3979 = ct{781};
t3980 = ct{782};
t3983 = ct{783};
t3985 = ct{784};
t3988 = ct{785};
t3991 = ct{786};
t3992 = ct{787};
t3993 = ct{788};
t3996 = ct{789};
t3998 = ct{790};
t3999 = ct{791};
t4001 = ct{792};
t4002 = ct{793};
t4006 = ct{794};
t4007 = ct{795};
t4008 = ct{796};
t4010 = ct{797};
t4014 = ct{798};
t4018 = ct{799};
t4019 = ct{800};
t4026 = ct{801};
t4030 = ct{802};
t4031 = ct{803};
t4032 = ct{804};
t4035 = ct{805};
t4039 = ct{806};
t4041 = ct{807};
t4045 = ct{808};
t4047 = ct{809};
t4049 = ct{810};
t4050 = ct{811};
t4051 = ct{812};
t4052 = ct{813};
t4053 = ct{814};
t4054 = ct{815};
t4056 = ct{816};
t4065 = ct{817};
t410 = ct{818};
t4100 = ct{819};
t4109 = ct{820};
t4110 = ct{821};
t4113 = ct{822};
t4114 = ct{823};
t4115 = ct{824};
t4118 = ct{825};
t4144 = ct{826};
t4146 = ct{827};
t4147 = ct{828};
t4151 = ct{829};
t4153 = ct{830};
t4154 = ct{831};
t4157 = ct{832};
t4158 = ct{833};
t4160 = ct{834};
t4163 = ct{835};
t4165 = ct{836};
t4168 = ct{837};
t4171 = ct{838};
t4172 = ct{839};
t4187 = ct{840};
t4188 = ct{841};
t4190 = ct{842};
t4193 = ct{843};
t4198 = ct{844};
t42 = ct{845};
t4201 = ct{846};
t4205 = ct{847};
t4207 = ct{848};
t4208 = ct{849};
t4213 = ct{850};
t4215 = ct{851};
t4218 = ct{852};
t4219 = ct{853};
t4224 = ct{854};
t4229 = ct{855};
t4230 = ct{856};
t4236 = ct{857};
t4240 = ct{858};
t4241 = ct{859};
t4243 = ct{860};
t4244 = ct{861};
t4246 = ct{862};
t4248 = ct{863};
t4249 = ct{864};
t4258 = ct{865};
t4260 = ct{866};
t4261 = ct{867};
t4263 = ct{868};
t4267 = ct{869};
t4270 = ct{870};
t4272 = ct{871};
t4273 = ct{872};
t4274 = ct{873};
t4275 = ct{874};
t4276 = ct{875};
t4277 = ct{876};
t4278 = ct{877};
t4279 = ct{878};
t4280 = ct{879};
t4281 = ct{880};
t4282 = ct{881};
t4283 = ct{882};
t4286 = ct{883};
t4287 = ct{884};
t4288 = ct{885};
t4289 = ct{886};
t429 = ct{887};
t4290 = ct{888};
t4291 = ct{889};
t4292 = ct{890};
t4293 = ct{891};
t4294 = ct{892};
t4295 = ct{893};
t4296 = ct{894};
t4297 = ct{895};
t4298 = ct{896};
t4299 = ct{897};
t43 = ct{898};
t4300 = ct{899};
t4301 = ct{900};
t4303 = ct{901};
t4304 = ct{902};
t4305 = ct{903};
t4306 = ct{904};
t4307 = ct{905};
t4308 = ct{906};
t4310 = ct{907};
t4311 = ct{908};
t4312 = ct{909};
t4313 = ct{910};
t4314 = ct{911};
t4318 = ct{912};
t4319 = ct{913};
t4321 = ct{914};
t4324 = ct{915};
t4325 = ct{916};
t4326 = ct{917};
t4330 = ct{918};
t4332 = ct{919};
t4334 = ct{920};
t4337 = ct{921};
t4339 = ct{922};
t4341 = ct{923};
t4342 = ct{924};
t4343 = ct{925};
t4344 = ct{926};
t4345 = ct{927};
t4346 = ct{928};
t4352 = ct{929};
t4354 = ct{930};
t4355 = ct{931};
t4356 = ct{932};
t4358 = ct{933};
t4359 = ct{934};
t4361 = ct{935};
t4362 = ct{936};
t4363 = ct{937};
t4364 = ct{938};
t4371 = ct{939};
t4372 = ct{940};
t4373 = ct{941};
t4375 = ct{942};
t4404 = ct{943};
t4406 = ct{944};
t4408 = ct{945};
t4411 = ct{946};
t4413 = ct{947};
t4415 = ct{948};
t4416 = ct{949};
t4417 = ct{950};
t4422 = ct{951};
t4423 = ct{952};
t4426 = ct{953};
t4427 = ct{954};
t4429 = ct{955};
t4430 = ct{956};
t4431 = ct{957};
t4432 = ct{958};
t4433 = ct{959};
t4435 = ct{960};
t4439 = ct{961};
t4440 = ct{962};
t4441 = ct{963};
t4442 = ct{964};
t4444 = ct{965};
t4445 = ct{966};
t4446 = ct{967};
t4447 = ct{968};
t4449 = ct{969};
t4457 = ct{970};
t4458 = ct{971};
t4459 = ct{972};
t4461 = ct{973};
t4464 = ct{974};
t4465 = ct{975};
t4466 = ct{976};
t4467 = ct{977};
t4468 = ct{978};
t4470 = ct{979};
t4476 = ct{980};
t4479 = ct{981};
t4482 = ct{982};
t4486 = ct{983};
t4488 = ct{984};
t4489 = ct{985};
t4491 = ct{986};
t4493 = ct{987};
t4494 = ct{988};
t4495 = ct{989};
t4496 = ct{990};
t4497 = ct{991};
t4501 = ct{992};
t4502 = ct{993};
t4504 = ct{994};
t4515 = ct{995};
t4517 = ct{996};
t4518 = ct{997};
t4520 = ct{998};
t4522 = ct{999};
t4523 = ct{1000};
t4532 = ct{1001};
t4534 = ct{1002};
t4537 = ct{1003};
t4545 = ct{1004};
t4553 = ct{1005};
t4559 = ct{1006};
t4561 = ct{1007};
t4562 = ct{1008};
t4563 = ct{1009};
t4564 = ct{1010};
t4566 = ct{1011};
t4567 = ct{1012};
t4568 = ct{1013};
t4569 = ct{1014};
t4570 = ct{1015};
t4571 = ct{1016};
t4573 = ct{1017};
t4574 = ct{1018};
t4576 = ct{1019};
t4577 = ct{1020};
t4578 = ct{1021};
t4579 = ct{1022};
t4580 = ct{1023};
t4582 = ct{1024};
t4583 = ct{1025};
t4584 = ct{1026};
t4585 = ct{1027};
t4588 = ct{1028};
t4589 = ct{1029};
t4590 = ct{1030};
t4591 = ct{1031};
t4593 = ct{1032};
t4594 = ct{1033};
t4595 = ct{1034};
t4598 = ct{1035};
t4599 = ct{1036};
t46 = ct{1037};
t4600 = ct{1038};
t4601 = ct{1039};
t4602 = ct{1040};
t4606 = ct{1041};
t4608 = ct{1042};
t4609 = ct{1043};
t4610 = ct{1044};
t4611 = ct{1045};
t4613 = ct{1046};
t4615 = ct{1047};
t4617 = ct{1048};
t4618 = ct{1049};
t4619 = ct{1050};
t4620 = ct{1051};
t4621 = ct{1052};
t4622 = ct{1053};
t4623 = ct{1054};
t4624 = ct{1055};
t4625 = ct{1056};
t4626 = ct{1057};
t4627 = ct{1058};
t4629 = ct{1059};
t4630 = ct{1060};
t4631 = ct{1061};
t4632 = ct{1062};
t4633 = ct{1063};
t4634 = ct{1064};
t4635 = ct{1065};
t4639 = ct{1066};
t4640 = ct{1067};
t4641 = ct{1068};
t4643 = ct{1069};
t4644 = ct{1070};
t4645 = ct{1071};
t4646 = ct{1072};
t4647 = ct{1073};
t4649 = ct{1074};
t4650 = ct{1075};
t4651 = ct{1076};
t4652 = ct{1077};
t4654 = ct{1078};
t4656 = ct{1079};
t4657 = ct{1080};
t4658 = ct{1081};
t4660 = ct{1082};
t4661 = ct{1083};
t4663 = ct{1084};
t4665 = ct{1085};
t4667 = ct{1086};
t4669 = ct{1087};
t4670 = ct{1088};
t4672 = ct{1089};
t4673 = ct{1090};
t4674 = ct{1091};
t4675 = ct{1092};
t4676 = ct{1093};
t4677 = ct{1094};
t4678 = ct{1095};
t4680 = ct{1096};
t4683 = ct{1097};
t4686 = ct{1098};
t4688 = ct{1099};
t4689 = ct{1100};
t4690 = ct{1101};
t4691 = ct{1102};
t4692 = ct{1103};
t4694 = ct{1104};
t4696 = ct{1105};
t4697 = ct{1106};
t4698 = ct{1107};
t47 = ct{1108};
t4703 = ct{1109};
t4704 = ct{1110};
t4705 = ct{1111};
t4708 = ct{1112};
t4709 = ct{1113};
t4711 = ct{1114};
t4712 = ct{1115};
t4713 = ct{1116};
t4716 = ct{1117};
t4719 = ct{1118};
t4720 = ct{1119};
t4722 = ct{1120};
t4724 = ct{1121};
t4725 = ct{1122};
t4727 = ct{1123};
t4728 = ct{1124};
t4730 = ct{1125};
t4733 = ct{1126};
t4735 = ct{1127};
t4737 = ct{1128};
t4739 = ct{1129};
t4741 = ct{1130};
t4743 = ct{1131};
t4744 = ct{1132};
t4746 = ct{1133};
t4751 = ct{1134};
t4757 = ct{1135};
t4760 = ct{1136};
t4761 = ct{1137};
t4762 = ct{1138};
t4763 = ct{1139};
t4764 = ct{1140};
t4766 = ct{1141};
t4767 = ct{1142};
t4770 = ct{1143};
t4771 = ct{1144};
t4772 = ct{1145};
t4774 = ct{1146};
t4776 = ct{1147};
t4777 = ct{1148};
t4778 = ct{1149};
t4779 = ct{1150};
t4783 = ct{1151};
t4785 = ct{1152};
t4786 = ct{1153};
t4787 = ct{1154};
t4790 = ct{1155};
t4791 = ct{1156};
t4793 = ct{1157};
t4795 = ct{1158};
t4796 = ct{1159};
t4797 = ct{1160};
t4799 = ct{1161};
t4800 = ct{1162};
t4801 = ct{1163};
t4805 = ct{1164};
t4808 = ct{1165};
t4809 = ct{1166};
t4810 = ct{1167};
t4811 = ct{1168};
t4813 = ct{1169};
t4814 = ct{1170};
t4815 = ct{1171};
t4816 = ct{1172};
t4818 = ct{1173};
t4821 = ct{1174};
t4822 = ct{1175};
t4823 = ct{1176};
t4825 = ct{1177};
t4826 = ct{1178};
t4828 = ct{1179};
t4830 = ct{1180};
t4833 = ct{1181};
t4835 = ct{1182};
t4838 = ct{1183};
t4843 = ct{1184};
t4844 = ct{1185};
t4845 = ct{1186};
t4846 = ct{1187};
t4847 = ct{1188};
t4848 = ct{1189};
t4849 = ct{1190};
t4850 = ct{1191};
t4851 = ct{1192};
t4852 = ct{1193};
t4853 = ct{1194};
t4854 = ct{1195};
t4856 = ct{1196};
t4857 = ct{1197};
t4858 = ct{1198};
t4859 = ct{1199};
t4863 = ct{1200};
t4867 = ct{1201};
t4872 = ct{1202};
t4874 = ct{1203};
t4875 = ct{1204};
t4876 = ct{1205};
t4879 = ct{1206};
t4880 = ct{1207};
t4881 = ct{1208};
t4886 = ct{1209};
t4887 = ct{1210};
t4888 = ct{1211};
t4889 = ct{1212};
t4892 = ct{1213};
t4893 = ct{1214};
t4895 = ct{1215};
t4896 = ct{1216};
t4898 = ct{1217};
t4901 = ct{1218};
t4902 = ct{1219};
t4903 = ct{1220};
t4904 = ct{1221};
t4905 = ct{1222};
t4906 = ct{1223};
t4907 = ct{1224};
t4908 = ct{1225};
t4911 = ct{1226};
t4912 = ct{1227};
t4913 = ct{1228};
t4914 = ct{1229};
t4915 = ct{1230};
t4918 = ct{1231};
t4919 = ct{1232};
t4920 = ct{1233};
t4921 = ct{1234};
t4922 = ct{1235};
t4923 = ct{1236};
t4924 = ct{1237};
t4925 = ct{1238};
t4926 = ct{1239};
t4927 = ct{1240};
t4928 = ct{1241};
t4929 = ct{1242};
t4930 = ct{1243};
t4933 = ct{1244};
t4934 = ct{1245};
t4935 = ct{1246};
t4936 = ct{1247};
t4937 = ct{1248};
t4938 = ct{1249};
t4939 = ct{1250};
t4940 = ct{1251};
t4941 = ct{1252};
t4943 = ct{1253};
t4945 = ct{1254};
t4946 = ct{1255};
t4947 = ct{1256};
t4948 = ct{1257};
t4949 = ct{1258};
t4950 = ct{1259};
t4952 = ct{1260};
t4953 = ct{1261};
t4955 = ct{1262};
t4957 = ct{1263};
t4958 = ct{1264};
t4959 = ct{1265};
t4964 = ct{1266};
t4965 = ct{1267};
t4966 = ct{1268};
t4968 = ct{1269};
t4969 = ct{1270};
t4970 = ct{1271};
t4971 = ct{1272};
t4973 = ct{1273};
t4974 = ct{1274};
t4976 = ct{1275};
t4977 = ct{1276};
t4979 = ct{1277};
t4981 = ct{1278};
t4983 = ct{1279};
t50 = ct{1280};
t5001 = ct{1281};
t5003 = ct{1282};
t5004 = ct{1283};
t5005 = ct{1284};
t5006 = ct{1285};
t5008 = ct{1286};
t5012 = ct{1287};
t5013 = ct{1288};
t5014 = ct{1289};
t5016 = ct{1290};
t5019 = ct{1291};
t5020 = ct{1292};
t5021 = ct{1293};
t5024 = ct{1294};
t5025 = ct{1295};
t5026 = ct{1296};
t5027 = ct{1297};
t5028 = ct{1298};
t5029 = ct{1299};
t5030 = ct{1300};
t5033 = ct{1301};
t5034 = ct{1302};
t5035 = ct{1303};
t5036 = ct{1304};
t5037 = ct{1305};
t5038 = ct{1306};
t5041 = ct{1307};
t5042 = ct{1308};
t5043 = ct{1309};
t5045 = ct{1310};
t5046 = ct{1311};
t5047 = ct{1312};
t5049 = ct{1313};
t5051 = ct{1314};
t5052 = ct{1315};
t5053 = ct{1316};
t5054 = ct{1317};
t5055 = ct{1318};
t5059 = ct{1319};
t5061 = ct{1320};
t5062 = ct{1321};
t5063 = ct{1322};
t5064 = ct{1323};
t5066 = ct{1324};
t5070 = ct{1325};
t5071 = ct{1326};
t5072 = ct{1327};
t5074 = ct{1328};
t5075 = ct{1329};
t5076 = ct{1330};
t5077 = ct{1331};
t5079 = ct{1332};
t5080 = ct{1333};
t5081 = ct{1334};
t5082 = ct{1335};
t5083 = ct{1336};
t5084 = ct{1337};
t5085 = ct{1338};
t5086 = ct{1339};
t5087 = ct{1340};
t5088 = ct{1341};
t5089 = ct{1342};
t5090 = ct{1343};
t5091 = ct{1344};
t5093 = ct{1345};
t5096 = ct{1346};
t5097 = ct{1347};
t5098 = ct{1348};
t5100 = ct{1349};
t5101 = ct{1350};
t5103 = ct{1351};
t5104 = ct{1352};
t5106 = ct{1353};
t5108 = ct{1354};
t5109 = ct{1355};
t5111 = ct{1356};
t5112 = ct{1357};
t5113 = ct{1358};
t5114 = ct{1359};
t5116 = ct{1360};
t5117 = ct{1361};
t5118 = ct{1362};
t5119 = ct{1363};
t5120 = ct{1364};
t5121 = ct{1365};
t5123 = ct{1366};
t5124 = ct{1367};
t5125 = ct{1368};
t5126 = ct{1369};
t5127 = ct{1370};
t5141 = ct{1371};
t5142 = ct{1372};
t5144 = ct{1373};
t5146 = ct{1374};
t5147 = ct{1375};
t5148 = ct{1376};
t5153 = ct{1377};
t5154 = ct{1378};
t5155 = ct{1379};
t5156 = ct{1380};
t5158 = ct{1381};
t5159 = ct{1382};
t5161 = ct{1383};
t5162 = ct{1384};
t5163 = ct{1385};
t5164 = ct{1386};
t5165 = ct{1387};
t5166 = ct{1388};
t5167 = ct{1389};
t5168 = ct{1390};
t5169 = ct{1391};
t5171 = ct{1392};
t5173 = ct{1393};
t5174 = ct{1394};
t5176 = ct{1395};
t5177 = ct{1396};
t5178 = ct{1397};
t5180 = ct{1398};
t5181 = ct{1399};
t5194 = ct{1400};
t5195 = ct{1401};
t5196 = ct{1402};
t5197 = ct{1403};
t5198 = ct{1404};
t5199 = ct{1405};
t5200 = ct{1406};
t5201 = ct{1407};
t5202 = ct{1408};
t5203 = ct{1409};
t5205 = ct{1410};
t5206 = ct{1411};
t5207 = ct{1412};
t5208 = ct{1413};
t5211 = ct{1414};
t5212 = ct{1415};
t5213 = ct{1416};
t5214 = ct{1417};
t5215 = ct{1418};
t5216 = ct{1419};
t5219 = ct{1420};
t5225 = ct{1421};
t5226 = ct{1422};
t5227 = ct{1423};
t5228 = ct{1424};
t5229 = ct{1425};
t5230 = ct{1426};
t5234 = ct{1427};
t5240 = ct{1428};
t5241 = ct{1429};
t5243 = ct{1430};
t5244 = ct{1431};
t5245 = ct{1432};
t5246 = ct{1433};
t5247 = ct{1434};
t5248 = ct{1435};
t5249 = ct{1436};
t5251 = ct{1437};
t5254 = ct{1438};
t5255 = ct{1439};
t5256 = ct{1440};
t5257 = ct{1441};
t5258 = ct{1442};
t5259 = ct{1443};
t5261 = ct{1444};
t5262 = ct{1445};
t5263 = ct{1446};
t5264 = ct{1447};
t5265 = ct{1448};
t5267 = ct{1449};
t5268 = ct{1450};
t5269 = ct{1451};
t5270 = ct{1452};
t5271 = ct{1453};
t5272 = ct{1454};
t5274 = ct{1455};
t5275 = ct{1456};
t5276 = ct{1457};
t5277 = ct{1458};
t5278 = ct{1459};
t5279 = ct{1460};
t5280 = ct{1461};
t5281 = ct{1462};
t5283 = ct{1463};
t5284 = ct{1464};
t5285 = ct{1465};
t5286 = ct{1466};
t5287 = ct{1467};
t5288 = ct{1468};
t5289 = ct{1469};
t5290 = ct{1470};
t5291 = ct{1471};
t5292 = ct{1472};
t5293 = ct{1473};
t5294 = ct{1474};
t5295 = ct{1475};
t5296 = ct{1476};
t5297 = ct{1477};
t5298 = ct{1478};
t5300 = ct{1479};
t5301 = ct{1480};
t5302 = ct{1481};
t5303 = ct{1482};
t5304 = ct{1483};
t5305 = ct{1484};
t5306 = ct{1485};
t5308 = ct{1486};
t5309 = ct{1487};
t5310 = ct{1488};
t5312 = ct{1489};
t5313 = ct{1490};
t5315 = ct{1491};
t5316 = ct{1492};
t5317 = ct{1493};
t5323 = ct{1494};
t5324 = ct{1495};
t5325 = ct{1496};
t5326 = ct{1497};
t5327 = ct{1498};
t5328 = ct{1499};
t5329 = ct{1500};
t5330 = ct{1501};
t5331 = ct{1502};
t5332 = ct{1503};
t5333 = ct{1504};
t5334 = ct{1505};
t5335 = ct{1506};
t5336 = ct{1507};
t5337 = ct{1508};
t5339 = ct{1509};
t5340 = ct{1510};
t5341 = ct{1511};
t5343 = ct{1512};
t5344 = ct{1513};
t5345 = ct{1514};
t5346 = ct{1515};
t5348 = ct{1516};
t5350 = ct{1517};
t5352 = ct{1518};
t5353 = ct{1519};
t5355 = ct{1520};
t5356 = ct{1521};
t5357 = ct{1522};
t5358 = ct{1523};
t5359 = ct{1524};
t5361 = ct{1525};
t5362 = ct{1526};
t5363 = ct{1527};
t5369 = ct{1528};
t5370 = ct{1529};
t5372 = ct{1530};
t5373 = ct{1531};
t5374 = ct{1532};
t5376 = ct{1533};
t5381 = ct{1534};
t5383 = ct{1535};
t5384 = ct{1536};
t5385 = ct{1537};
t5386 = ct{1538};
t5387 = ct{1539};
t5389 = ct{1540};
t5390 = ct{1541};
t5391 = ct{1542};
t5392 = ct{1543};
t5393 = ct{1544};
t5395 = ct{1545};
t5399 = ct{1546};
t5400 = ct{1547};
t5401 = ct{1548};
t5402 = ct{1549};
t5403 = ct{1550};
t5404 = ct{1551};
t5405 = ct{1552};
t5408 = ct{1553};
t5410 = ct{1554};
t5411 = ct{1555};
t5412 = ct{1556};
t5413 = ct{1557};
t5414 = ct{1558};
t5415 = ct{1559};
t5416 = ct{1560};
t5419 = ct{1561};
t5421 = ct{1562};
t5424 = ct{1563};
t5425 = ct{1564};
t5426 = ct{1565};
t5431 = ct{1566};
t5433 = ct{1567};
t5434 = ct{1568};
t5436 = ct{1569};
t5437 = ct{1570};
t5438 = ct{1571};
t5439 = ct{1572};
t5440 = ct{1573};
t5441 = ct{1574};
t5442 = ct{1575};
t5443 = ct{1576};
t5444 = ct{1577};
t5445 = ct{1578};
t5446 = ct{1579};
t5447 = ct{1580};
t5448 = ct{1581};
t5449 = ct{1582};
t5451 = ct{1583};
t5452 = ct{1584};
t5456 = ct{1585};
t5457 = ct{1586};
t5458 = ct{1587};
t5459 = ct{1588};
t5460 = ct{1589};
t5461 = ct{1590};
t5462 = ct{1591};
t5464 = ct{1592};
t5465 = ct{1593};
t5466 = ct{1594};
t5470 = ct{1595};
t5472 = ct{1596};
t5473 = ct{1597};
t5474 = ct{1598};
t5480 = ct{1599};
t5481 = ct{1600};
t5483 = ct{1601};
t5487 = ct{1602};
t5488 = ct{1603};
t5494 = ct{1604};
t5495 = ct{1605};
t5499 = ct{1606};
t5500 = ct{1607};
t5501 = ct{1608};
t5502 = ct{1609};
t5503 = ct{1610};
t5504 = ct{1611};
t5506 = ct{1612};
t5507 = ct{1613};
t5508 = ct{1614};
t5509 = ct{1615};
t5510 = ct{1616};
t5512 = ct{1617};
t5513 = ct{1618};
t5514 = ct{1619};
t5516 = ct{1620};
t5517 = ct{1621};
t5520 = ct{1622};
t5522 = ct{1623};
t5523 = ct{1624};
t5524 = ct{1625};
t5527 = ct{1626};
t5528 = ct{1627};
t5529 = ct{1628};
t5531 = ct{1629};
t5532 = ct{1630};
t5535 = ct{1631};
t5536 = ct{1632};
t5537 = ct{1633};
t5538 = ct{1634};
t5539 = ct{1635};
t5540 = ct{1636};
t5541 = ct{1637};
t5542 = ct{1638};
t5543 = ct{1639};
t5544 = ct{1640};
t5545 = ct{1641};
t5548 = ct{1642};
t5549 = ct{1643};
t5550 = ct{1644};
t5553 = ct{1645};
t5554 = ct{1646};
t5555 = ct{1647};
t5556 = ct{1648};
t5557 = ct{1649};
t5560 = ct{1650};
t5565 = ct{1651};
t5567 = ct{1652};
t5568 = ct{1653};
t5569 = ct{1654};
t5570 = ct{1655};
t5572 = ct{1656};
t5573 = ct{1657};
t5574 = ct{1658};
t5575 = ct{1659};
t5576 = ct{1660};
t5577 = ct{1661};
t5578 = ct{1662};
t5579 = ct{1663};
t5581 = ct{1664};
t5586 = ct{1665};
t5587 = ct{1666};
t5588 = ct{1667};
t5589 = ct{1668};
t5590 = ct{1669};
t5591 = ct{1670};
t5592 = ct{1671};
t5593 = ct{1672};
t5594 = ct{1673};
t5596 = ct{1674};
t5597 = ct{1675};
t5598 = ct{1676};
t5599 = ct{1677};
t56 = ct{1678};
t5600 = ct{1679};
t5601 = ct{1680};
t5602 = ct{1681};
t5603 = ct{1682};
t5604 = ct{1683};
t5605 = ct{1684};
t5606 = ct{1685};
t5607 = ct{1686};
t5608 = ct{1687};
t5609 = ct{1688};
t5611 = ct{1689};
t5612 = ct{1690};
t5613 = ct{1691};
t5614 = ct{1692};
t5615 = ct{1693};
t5616 = ct{1694};
t5619 = ct{1695};
t5623 = ct{1696};
t5624 = ct{1697};
t5625 = ct{1698};
t5629 = ct{1699};
t5630 = ct{1700};
t5631 = ct{1701};
t5632 = ct{1702};
t5633 = ct{1703};
t5634 = ct{1704};
t5635 = ct{1705};
t5636 = ct{1706};
t5637 = ct{1707};
t5638 = ct{1708};
t5639 = ct{1709};
t5644 = ct{1710};
t5645 = ct{1711};
t5646 = ct{1712};
t5649 = ct{1713};
t5650 = ct{1714};
t5651 = ct{1715};
t5653 = ct{1716};
t5654 = ct{1717};
t5655 = ct{1718};
t5657 = ct{1719};
t5658 = ct{1720};
t5659 = ct{1721};
t5660 = ct{1722};
t5661 = ct{1723};
t5662 = ct{1724};
t5663 = ct{1725};
t5666 = ct{1726};
t5675 = ct{1727};
t5676 = ct{1728};
t5677 = ct{1729};
t5678 = ct{1730};
t5679 = ct{1731};
t5680 = ct{1732};
t5684 = ct{1733};
t5689 = ct{1734};
t5691 = ct{1735};
t5694 = ct{1736};
t5698 = ct{1737};
t5699 = ct{1738};
t5701 = ct{1739};
t5702 = ct{1740};
t5717 = ct{1741};
t5718 = ct{1742};
t5719 = ct{1743};
t5720 = ct{1744};
t5721 = ct{1745};
t5722 = ct{1746};
t5724 = ct{1747};
t5725 = ct{1748};
t5727 = ct{1749};
t5730 = ct{1750};
t5731 = ct{1751};
t5734 = ct{1752};
t5735 = ct{1753};
t5736 = ct{1754};
t5738 = ct{1755};
t5739 = ct{1756};
t5741 = ct{1757};
t5742 = ct{1758};
t5745 = ct{1759};
t5747 = ct{1760};
t5749 = ct{1761};
t5750 = ct{1762};
t5751 = ct{1763};
t5752 = ct{1764};
t5757 = ct{1765};
t5758 = ct{1766};
t5759 = ct{1767};
t5760 = ct{1768};
t5761 = ct{1769};
t5763 = ct{1770};
t5764 = ct{1771};
t5765 = ct{1772};
t5766 = ct{1773};
t5768 = ct{1774};
t5769 = ct{1775};
t5770 = ct{1776};
t5775 = ct{1777};
t5776 = ct{1778};
t5777 = ct{1779};
t5778 = ct{1780};
t5779 = ct{1781};
t5781 = ct{1782};
t5782 = ct{1783};
t5783 = ct{1784};
t5784 = ct{1785};
t5787 = ct{1786};
t5788 = ct{1787};
t5790 = ct{1788};
t5792 = ct{1789};
t5793 = ct{1790};
t5794 = ct{1791};
t5795 = ct{1792};
t58 = ct{1793};
t5801 = ct{1794};
t5802 = ct{1795};
t5804 = ct{1796};
t5805 = ct{1797};
t5806 = ct{1798};
t5813 = ct{1799};
t5814 = ct{1800};
t5821 = ct{1801};
t5822 = ct{1802};
t5823 = ct{1803};
t5824 = ct{1804};
t5825 = ct{1805};
t5835 = ct{1806};
t5836 = ct{1807};
t5839 = ct{1808};
t5842 = ct{1809};
t5849 = ct{1810};
t5851 = ct{1811};
t5852 = ct{1812};
t5853 = ct{1813};
t5855 = ct{1814};
t5863 = ct{1815};
t5864 = ct{1816};
t5865 = ct{1817};
t5866 = ct{1818};
t5876 = ct{1819};
t5885 = ct{1820};
t5886 = ct{1821};
t5887 = ct{1822};
t5891 = ct{1823};
t5892 = ct{1824};
t5896 = ct{1825};
t59 = ct{1826};
t5901 = ct{1827};
t5902 = ct{1828};
t5904 = ct{1829};
t5908 = ct{1830};
t5909 = ct{1831};
t5916 = ct{1832};
t5917 = ct{1833};
t5918 = ct{1834};
t5919 = ct{1835};
t5920 = ct{1836};
t5922 = ct{1837};
t5924 = ct{1838};
t5925 = ct{1839};
t5928 = ct{1840};
t5929 = ct{1841};
t5930 = ct{1842};
t5933 = ct{1843};
t5938 = ct{1844};
t5941 = ct{1845};
t5954 = ct{1846};
t5955 = ct{1847};
t5959 = ct{1848};
t5960 = ct{1849};
t5963 = ct{1850};
t5964 = ct{1851};
t5966 = ct{1852};
t5967 = ct{1853};
t5968 = ct{1854};
t5971 = ct{1855};
t5973 = ct{1856};
t5978 = ct{1857};
t5979 = ct{1858};
t5980 = ct{1859};
t5990 = ct{1860};
t5992 = ct{1861};
t5993 = ct{1862};
t60 = ct{1863};
t6002 = ct{1864};
t6004 = ct{1865};
t6005 = ct{1866};
t6011 = ct{1867};
t6013 = ct{1868};
t6014 = ct{1869};
t6015 = ct{1870};
t6019 = ct{1871};
t6020 = ct{1872};
t6022 = ct{1873};
t6023 = ct{1874};
t6024 = ct{1875};
t6031 = ct{1876};
t6047 = ct{1877};
t6048 = ct{1878};
t6050 = ct{1879};
t6052 = ct{1880};
t6054 = ct{1881};
t6056 = ct{1882};
t6057 = ct{1883};
t6059 = ct{1884};
t6062 = ct{1885};
t6066 = ct{1886};
t6067 = ct{1887};
t6069 = ct{1888};
t6070 = ct{1889};
t6071 = ct{1890};
t6072 = ct{1891};
t6074 = ct{1892};
t6076 = ct{1893};
t6079 = ct{1894};
t6080 = ct{1895};
t6081 = ct{1896};
t6091 = ct{1897};
t6093 = ct{1898};
t6094 = ct{1899};
t6095 = ct{1900};
t6096 = ct{1901};
t6101 = ct{1902};
t6113 = ct{1903};
t6114 = ct{1904};
t6115 = ct{1905};
t6119 = ct{1906};
t6123 = ct{1907};
t6125 = ct{1908};
t6126 = ct{1909};
t6127 = ct{1910};
t6129 = ct{1911};
t6131 = ct{1912};
t6133 = ct{1913};
t6134 = ct{1914};
t6143 = ct{1915};
t6144 = ct{1916};
t6154 = ct{1917};
t6158 = ct{1918};
t6162 = ct{1919};
t6164 = ct{1920};
t6166 = ct{1921};
t6168 = ct{1922};
t6172 = ct{1923};
t6183 = ct{1924};
t6211 = ct{1925};
t6213 = ct{1926};
t6217 = ct{1927};
t6219 = ct{1928};
t6221 = ct{1929};
t6222 = ct{1930};
t6227 = ct{1931};
t6232 = ct{1932};
t6241 = ct{1933};
t6255 = ct{1934};
t6256 = ct{1935};
t6257 = ct{1936};
t6270 = ct{1937};
t6271 = ct{1938};
t6272 = ct{1939};
t6307 = ct{1940};
t6324 = ct{1941};
t6366 = ct{1942};
t6375 = ct{1943};
t6377 = ct{1944};
t638 = ct{1945};
t6388 = ct{1946};
t6394 = ct{1947};
t6396 = ct{1948};
t6398 = ct{1949};
t640 = ct{1950};
t6411 = ct{1951};
t6412 = ct{1952};
t642 = ct{1953};
t6425 = ct{1954};
t643 = ct{1955};
t6438 = ct{1956};
t6440 = ct{1957};
t6442 = ct{1958};
t6460 = ct{1959};
t6461 = ct{1960};
t6482 = ct{1961};
t6483 = ct{1962};
t6484 = ct{1963};
t649 = ct{1964};
t6491 = ct{1965};
t6508 = ct{1966};
t6515 = ct{1967};
t6517 = ct{1968};
t6523 = ct{1969};
t6524 = ct{1970};
t6525 = ct{1971};
t6526 = ct{1972};
t6527 = ct{1973};
t6528 = ct{1974};
t654 = ct{1975};
t655 = ct{1976};
t656 = ct{1977};
t6560 = ct{1978};
t6564 = ct{1979};
t6565 = ct{1980};
t657 = ct{1981};
t6574 = ct{1982};
t6581 = ct{1983};
t6588 = ct{1984};
t6589 = ct{1985};
t659 = ct{1986};
t6594 = ct{1987};
t660 = ct{1988};
t6602 = ct{1989};
t6622 = ct{1990};
t6623 = ct{1991};
t6651 = ct{1992};
t6661 = ct{1993};
t6662 = ct{1994};
t667 = ct{1995};
t668 = ct{1996};
t6680 = ct{1997};
t669 = ct{1998};
t67 = ct{1999};
t670 = ct{2000};
t674 = ct{2001};
t6745 = ct{2002};
t6751 = ct{2003};
t677 = ct{2004};
t68 = ct{2005};
t681 = ct{2006};
t682 = ct{2007};
t684 = ct{2008};
t685 = ct{2009};
t686 = ct{2010};
t687 = ct{2011};
t6919 = ct{2012};
t692 = ct{2013};
t6920 = ct{2014};
t693 = ct{2015};
t694 = ct{2016};
t6965 = ct{2017};
t6966 = ct{2018};
t6987 = ct{2019};
t7003 = ct{2020};
t7005 = ct{2021};
t7007 = ct{2022};
t7014 = ct{2023};
t702 = ct{2024};
t7035 = ct{2025};
t707 = ct{2026};
t708 = ct{2027};
t7086 = ct{2028};
t7088 = ct{2029};
t7093 = ct{2030};
t7094 = ct{2031};
t7096 = ct{2032};
t71 = ct{2033};
t710 = ct{2034};
t7134 = ct{2035};
t7135 = ct{2036};
t7137 = ct{2037};
t7138 = ct{2038};
t7148 = ct{2039};
t715 = ct{2040};
t7150 = ct{2041};
t7153 = ct{2042};
t7154 = ct{2043};
t7158 = ct{2044};
t716 = ct{2045};
t7160 = ct{2046};
t7167 = ct{2047};
t7199 = ct{2048};
t721 = ct{2049};
t722 = ct{2050};
t724 = ct{2051};
t725 = ct{2052};
t73 = ct{2053};
t7304 = ct{2054};
t7319 = ct{2055};
t7331 = ct{2056};
t7332 = ct{2057};
t7333 = ct{2058};
t7334 = ct{2059};
t736 = ct{2060};
t738 = ct{2061};
t740 = ct{2062};
t741 = ct{2063};
t749 = ct{2064};
t762 = ct{2065};
t768 = ct{2066};
t777 = ct{2067};
t792 = ct{2068};
t793 = ct{2069};
t8 = ct{2070};
t801 = ct{2071};
t802 = ct{2072};
t808 = ct{2073};
t813 = ct{2074};
t819 = ct{2075};
t821 = ct{2076};
t850 = ct{2077};
t855 = ct{2078};
t874 = ct{2079};
t878 = ct{2080};
t89 = ct{2081};
t9 = ct{2082};
t92 = ct{2083};
t941 = ct{2084};
t948 = ct{2085};
t951 = ct{2086};
t97 = ct{2087};
et135 = t18.*t19.*t26.*t27.*t50.*t202.*(-3.509445006623964e-21);
et136 = t21.*t24.*t25.*t26.*t50.*t202.*(-7.696420262413979e-21);
t6576 = t4712.*(et132+et133+et134+et135+et136).*(-1.0./2.0);
et137 = t1288+t1289+t1302+t1303-t1319-t1320+t1336-t1348+t1350+t1351-t1360+t1369-t1378+t1396-t1425+t1435-t2174+t2183-t2187+t2193-t2194-t2195+t2199-t2203-t2215+t2219-t2222-t2223+t2239+t2240-t2256-t2257+t2555+t2556+t2572+t2583-t2605-t2606+t2612+t2613-t2618-t2619+t2651+t2652;
et138 = t18.*t19.*t20.*t50.*t202.*(-3.566935413776081e-21);
et139 = t24.*t25.*t26.*t50.*t202.*(-3.992732227073824e-24);
et140 = t18.*t19.*t26.*t27.*t50.*t202.*(-3.509445006623964e-21);
et141 = t21.*t24.*t25.*t26.*t50.*t202.*(-7.696420262413979e-21);
t6577 = (t4712.*(et137+et138+et139+et140+et141))./2.0;
t6595 = -t6594;
et142 = t1288+t1289+t1302+t1303-t1319-t1320+t1336-t1348+t1350+t1351-t1360+t1369-t1378+t1396-t1425+t1435-t2174+t2183-t2187+t2193-t2194-t2195+t2199-t2203-t2215+t2219-t2222-t2223+t2239+t2240-t2256-t2257+t2555+t2556+t2572+t2583-t2605-t2606+t2612+t2613-t2618-t2619+t2651+t2652;
et143 = t18.*t19.*t20.*t50.*t202.*(-3.566935413776081e-21);
et144 = t24.*t25.*t26.*t50.*t202.*(-3.992732227073824e-24);
et145 = t18.*t19.*t26.*t27.*t50.*t202.*(-3.509445006623964e-21);
et146 = t21.*t24.*t25.*t26.*t50.*t202.*(-7.696420262413979e-21);
t6601 = t4950.*(et142+et143+et144+et145+et146).*(-1.0./2.0);
t6603 = -t6602;
t6606 = t3055.*t6581;
t6652 = t2736+t2797+t2937+t2942+t3004+t3008+t3999+t4230+t4249+t4258+t4945+t4947;
et147 = t707+t708-t721-t722-t749+t762+t768-t777-t792-t793-t801-t802-t808+t813-t819+t821-t1629+t1637-t1640-t1641-t1659-t1661+t1666+t1667+t1683+t1692+t1705-t1712+t1758+t1759+t1775+t1776+t1973+t1993+t1994+t2023+t2053+t2060-t2089-t2090+t2098+t2099-t8.*t9.*t15.*t50.*t189.*3.670836568391568e-22;
et148 = t10.*t13.*t14.*t50.*t189.*(-3.279367663374749e-19)-t8.*t9.*t11.*t15.*t50.*t189.*7.075931802640439e-19;
et149 = t8.*t11.*t14.*t15.*t50.*t189.*(-1.190170786299927e-18)-t9.*t11.*t13.*t15.*t50.*t189.*1.190170786299927e-18;
et150 = t13.*t14.*t15.*t16.*t50.*t189.*(-3.226512155691387e-19);
t6671 = t5594.*(et147+et148+et149+et150).*(-1.0./2.0);
t6712 = -t6581.*(t3242-t3554);
t6713 = t4026.*t6581;
t6714 = t6581.*(t3242-t3554);
t6726 = t3343+t3452+t4934+t4941+t5168+t5174;
et151 = t1288+t1289+t1302+t1303-t1319-t1320+t1336-t1348+t1350+t1351-t1360+t1369-t1378+t1396-t1425+t1435-t2174+t2183-t2187+t2193-t2194-t2195+t2199-t2203-t2215+t2219-t2222-t2223+t2239+t2240-t2256-t2257+t2555+t2556+t2572+t2583-t2605-t2606+t2612+t2613-t2618-t2619+t2651+t2652;
et152 = t18.*t19.*t20.*t50.*t202.*(-3.566935413776081e-21);
et153 = t24.*t25.*t26.*t50.*t202.*(-3.992732227073824e-24);
et154 = t18.*t19.*t26.*t27.*t50.*t202.*(-3.509445006623964e-21);
et155 = t21.*t24.*t25.*t26.*t50.*t202.*(-7.696420262413979e-21);
t6857 = t5465.*(et151+et152+et153+et154+et155).*(-1.0./2.0);
et156 = t1288+t1289+t1302+t1303-t1319-t1320+t1336-t1348+t1350+t1351-t1360+t1369-t1378+t1396-t1425+t1435-t2174+t2183-t2187+t2193-t2194-t2195+t2199-t2203-t2215+t2219-t2222-t2223+t2239+t2240-t2256-t2257+t2555+t2556+t2572+t2583-t2605-t2606+t2612+t2613-t2618-t2619+t2651+t2652;
et157 = t18.*t19.*t20.*t50.*t202.*(-3.566935413776081e-21);
et158 = t24.*t25.*t26.*t50.*t202.*(-3.992732227073824e-24);
et159 = t18.*t19.*t26.*t27.*t50.*t202.*(-3.509445006623964e-21);
et160 = t21.*t24.*t25.*t26.*t50.*t202.*(-7.696420262413979e-21);
t6858 = (t5465.*(et156+et157+et158+et159+et160))./2.0;
t6974 = -t2363.*(t3157+t3158+t3386-t4299-t4300-t4562+t4567+t3543.*(t1861-t3221).*6.2e-7+t3500.*(t1896-t3239).*6.2e-7-(t11.*(t1861-t3221).*(t1896-t3239))./1.0e+8-(t11.*t2297.*t2363)./1.0e+8-(t11.*t3502.*t3547)./1.0e+8);
t6976 = t2363.*(t3157+t3158+t3386-t4299-t4300-t4562+t4567+t3543.*(t1861-t3221).*6.2e-7+t3500.*(t1896-t3239).*6.2e-7-(t11.*(t1861-t3221).*(t1896-t3239))./1.0e+8-(t11.*t2297.*t2363)./1.0e+8-(t11.*t3502.*t3547)./1.0e+8).*(-1.0./2.0);
t7015 = -t7014;
t7020 = (t1896-t3239).*(t3157+t3158+t3386-t4299-t4300-t4562+t4567+t3543.*(t1861-t3221).*6.2e-7+t3500.*(t1896-t3239).*6.2e-7-(t11.*(t1861-t3221).*(t1896-t3239))./1.0e+8-(t11.*t2297.*t2363)./1.0e+8-(t11.*t3502.*t3547)./1.0e+8);
t7021 = -t3547.*(t3157+t3158+t3386-t4299-t4300-t4562+t4567+t3543.*(t1861-t3221).*6.2e-7+t3500.*(t1896-t3239).*6.2e-7-(t11.*(t1861-t3221).*(t1896-t3239))./1.0e+8-(t11.*t2297.*t2363)./1.0e+8-(t11.*t3502.*t3547)./1.0e+8);
t7053 = -t3055.*(t5288-t5329+t5330+t3934.*(t11.*((t237.*(t42-t43))./9.007199254740992e+15+t15.*(-t1881+t3121+t3276))+t16.*(-t1901+t3122+t3277)).*1.02e-6);
t7054 = t3055.*(t5288-t5329+t5330+t3934.*(t11.*((t237.*(t42-t43))./9.007199254740992e+15+t15.*(-t1881+t3121+t3276))+t16.*(-t1901+t3122+t3277)).*1.02e-6);
t7083 = t5268+t5805+t5823;
t7095 = -t7093;
t7097 = -t7096;
t7098 = t7096./2.0;
t7120 = (t3242-t3554).*(t5288-t5329+t5330+t3934.*(t11.*((t237.*(t42-t43))./9.007199254740992e+15+t15.*(-t1881+t3121+t3276))+t16.*(-t1901+t3122+t3277)).*1.02e-6);
t7123 = -t4026.*(t5288-t5329+t5330+t3934.*(t11.*((t237.*(t42-t43))./9.007199254740992e+15+t15.*(-t1881+t3121+t3276))+t16.*(-t1901+t3122+t3277)).*1.02e-6);
t7136 = -t7134;
t7151 = t1599+t1704+t2360+t2391+t2404+t2405+t2438+t2472+t2575+t2638+t2984+t2987+t3180+t3394+t3949+t3988+t3998+t4188+t4219+t4224+t4918+t4919;
t7164 = t3915.*(-t5264+t5804+t5698.*(t1896-t3239)).*(-1.0./2.0);
t7169 = -t7167;
t7173 = t1613+t2360+t2448+t2449+t2461+t2471+t2492+t2575+t2638+t2984+t2987+t3983+t3992+t3996+t4218+t4219+t4224+t4229+t4918+t4919;
t7283 = t5527+t6056+t6070;
t7292 = t3163+t3164+t3256+t3392+t4667+t4669+t4670+t4672+t4921+t4922+t5144+t5146;
t7384 = -t2363.*(-t5215+t5274+t5325-t5327+t4920.*(t1861-t3221).*6.2e-7+t3934.*(t951+t10.*(-t1881+t3121+t3276)).*6.2e-7+t4118.*(t2694-t2701+t3036-t3043).*6.2e-7+(t4838.*(t2694-t2701+t3036-t3043))./1.0e+8);
t7385 = t2363.*(-t5215+t5274+t5325-t5327+t4920.*(t1861-t3221).*6.2e-7+t3934.*(t951+t10.*(-t1881+t3121+t3276)).*6.2e-7+t4118.*(t2694-t2701+t3036-t3043).*6.2e-7+(t4838.*(t2694-t2701+t3036-t3043))./1.0e+8);
t7400 = (t1896-t3239).*(-t5215+t5274+t5325-t5327+t4920.*(t1861-t3221).*6.2e-7+t3934.*(t951+t10.*(-t1881+t3121+t3276)).*6.2e-7+t4118.*(t2694-t2701+t3036-t3043).*6.2e-7+(t4838.*(t2694-t2701+t3036-t3043))./1.0e+8);
t7401 = -t3547.*(-t5215+t5274+t5325-t5327+t4920.*(t1861-t3221).*6.2e-7+t3934.*(t951+t10.*(-t1881+t3121+t3276)).*6.2e-7+t4118.*(t2694-t2701+t3036-t3043).*6.2e-7+(t4838.*(t2694-t2701+t3036-t3043))./1.0e+8);
t7403 = t3547.*(-t5215+t5274+t5325-t5327+t4920.*(t1861-t3221).*6.2e-7+t3934.*(t951+t10.*(-t1881+t3121+t3276)).*6.2e-7+t4118.*(t2694-t2701+t3036-t3043).*6.2e-7+(t4838.*(t2694-t2701+t3036-t3043))./1.0e+8);
t7784 = t5424+t5865+t5885+t6222+t7135+t7154;
et161 = t3015-t3068+t4470-t4518+t3500.*(t1959-t3313+t38.*t1022.*(t855-t878).*2.196325630278387e-1).*9.840000000000001e-6;
et162 = t3237.*((t237.*(t42-t43))./9.007199254740992e+15+t15.*(-t1881+t3121+t3276)).*9.840000000000001e-6;
t7790 = t3216.*(t5425+t5886+t7134+t5699.*(t1959-t3313+t38.*t1022.*(t855-t878).*2.196325630278387e-1)+t7088.*(t1896-t3239)+t3543.*(et161+et162)).*(-1.0./2.0);
t7827 = t5654+t6126+t6154+t6662+t7331+t7334;
t4072 = t4006.*9.99471e-3;
t4073 = t4007.*9.99471e-3;
t4074 = t4006.*1.838876e-2;
t4075 = t4007.*1.838876e-2;
t4124 = t4052.*1.838876e-2;
t4127 = t4051.*9.99471e-3;
t4128 = t4052.*9.99471e-3;
t4129 = t4051.*1.838876e-2;
t4183 = t4051.*1.33637554986e-4;
t4184 = t4052.*1.33637554986e-4;
t4185 = t4051.*7.26350557185e-5;
t4186 = t4052.*7.26350557185e-5;
t4368 = -t4363;
t4450 = -t4446;
t4451 = -t4447;
t4556 = t3510+t4007;
t4557 = t3522+t4006;
t4586 = -t4582;
t4592 = t3237.*t4267.*1.02e-6;
t4597 = -t4590;
t4603 = t3237.*t4267.*9.0e-8;
t4604 = t3562+t4052;
t4616 = t3569+t4051;
t4628 = -t4619;
t4638 = -t4633;
t4642 = -t4639;
t4662 = -t4661;
t4699 = t3547.*t4267.*1.02e-6;
t4701 = t3547.*t4267.*9.0e-8;
t4738 = -t4735;
t4773 = -t4772;
t4817 = -t4808;
t4819 = -t4809;
t4827 = -t4821;
t4829 = -t4823;
t4832 = -t4830;
t4865 = t3237.*(t3512-t4006).*(-9.3e-7);
t4866 = t3237.*(t3512-t4006).*(-1.02e-6);
t4870 = t3237.*(t3512-t4006).*(-9.0e-8);
t4909 = -t4905;
t4910 = -t4906;
t4960 = t3934.*t4267.*1.02e-6;
t4962 = t3934.*t4267.*9.0e-8;
t4967 = -t4964;
t4972 = -t4968;
t4975 = t21.*t4966;
t4978 = t21.*t4970;
t4980 = t21.*t4971;
t4982 = t21.*t4976;
t4988 = t3547.*(t3512-t4006).*(-9.3e-7);
t4989 = t3547.*(t3512-t4006).*(-1.02e-6);
t4992 = t3547.*(t3512-t4006).*9.3e-7;
t4993 = t3550.*(t3512-t4006).*(-1.02e-6);
t4994 = t3547.*(t3512-t4006).*(-9.0e-8);
t4997 = t3547.*(t3512-t4006).*9.0e-8;
t4998 = t3550.*(t3512-t4006).*(-9.0e-8);
t5007 = -t5006;
t5009 = t4026.*t4267.*1.02e-6;
t5010 = -t5008;
t5011 = t4026.*t4267.*9.0e-8;
t5022 = -t4292.*(t2813-t2835+t12.*(t1456-t2355).*1.02e-6+t17.*(t1456-t2355).*9.0e-8);
t5023 = t4292.*(t2813-t2835+t12.*(t1456-t2355).*1.02e-6+t17.*(t1456-t2355).*9.0e-8);
t5032 = -t3760.*(t3563-t4051);
t5057 = -t3874.*(t3563-t4051);
t5105 = -t5104;
t5132 = t3934.*(t3512-t4006).*(-9.3e-7);
t5133 = t3934.*(t3512-t4006).*(-1.02e-6);
t5135 = t3937.*(t3512-t4006).*(-1.02e-6);
t5136 = t3934.*(t3512-t4006).*9.3e-7;
t5137 = t3934.*(t3512-t4006).*(-9.0e-8);
t5138 = t3937.*(t3512-t4006).*(-9.0e-8);
t5139 = t3934.*(t3512-t4006).*9.0e-8;
t5149 = -t5147;
t5150 = -t5148;
t5152 = -t3979.*(t3563-t4051);
t5185 = t4026.*(t3512-t4006).*(-9.3e-7);
t5187 = t4026.*(t3512-t4006).*(-1.02e-6);
t5188 = t4026.*(t3512-t4006).*9.3e-7;
t5189 = t4026.*(t3512-t4006).*(-9.0e-8);
t5191 = t4031.*(t3512-t4006).*(-1.02e-6);
t5192 = t4026.*(t3512-t4006).*9.0e-8;
t5193 = t4031.*(t3512-t4006).*(-9.0e-8);
t5222 = t4151.*(t3512-t4006).*(-1.02e-6);
t5223 = t4151.*(t3512-t4006).*(-9.0e-8);
t5235 = (t3563-t4051).*(-t2804+t2838+t3109+t17.*(t1456-t2355).*9.3e-7);
t5236 = (t3563-t4051).*(t2813-t2835+t12.*(t1456-t2355).*1.02e-6+t17.*(t1456-t2355).*9.0e-8);
t5237 = -t4163.*(t3563-t4051);
t5338 = -t5333;
t5342 = -t5341;
t5364 = t50.*t189.*t5313.*9.543032792050485e-17;
t5366 = t50.*t189.*t5317.*9.543032792050485e-17;
t5375 = t3598+t3599+t4045+t4056;
t5379 = t50.*t202.*t5355.*6.935255936130809e-19;
t5382 = t3225+t4404+t4411;
t5396 = t3644+t3645+t4110+t4113;
t5406 = t3266+t4423+t4445;
t5420 = t3722+t3726+t4158+t4168;
t5422 = -t5421;
t5453 = t21.*t2363.*t5405;
t5467 = t3003.*t5405;
t5477 = t4872.*(t3512-t4006).*(-1.02e-6);
t5478 = t4872.*(t3512-t4006).*(-9.0e-8);
t5484 = t3387+t4561+t4569;
t5486 = t3055.*t5405;
t5489 = -t5405.*(t1477-t2502);
t5491 = t56+t73+t5466;
t5493 = t5405.*(t1477-t2502).*(-1.0./2.0);
t5497 = (t5405.*(t1477-t2502))./2.0;
t5498 = t71+t97+t5466;
t5505 = -t5502;
t5511 = -t5508;
t5519 = t4915.*(t3512-t4006).*(-1.02e-6);
t5521 = t4915.*(t3512-t4006).*(-9.0e-8);
t5533 = t3434+t4591+t4611;
t5534 = t3438+t4584+t4621;
t5558 = -t5557;
t5562 = -t21.*t5405.*(t1896-t3239);
t5563 = t21.*t3547.*t5405;
t5564 = t21.*t5405.*(t1896-t3239);
t5583 = -t5581;
t5585 = t5581./2.0;
t5618 = -t2363.*(t4772+(t3976.*(t2694-t2701+t3036-t3043))./1.0e+8);
t5622 = t2363.*(t4772+(t3976.*(t2694-t2701+t3036-t3043))./1.0e+8);
t5640 = t21.*t2363.*t5572;
t5647 = t326+t339+t5603;
t5648 = t362+t380+t5603;
t5652 = -t5651;
t5667 = t2294+t2325+t3302+t3316+t5275;
t5672 = t3003.*t5572;
t5681 = -t3055.*(t4809+t3976.*(t2694-t2701+t3036-t3043).*1.02e-6);
t5682 = t3055.*t5572;
t5683 = -t5572.*(t1477-t2502);
t5685 = t3055.*(t4809+t3976.*(t2694-t2701+t3036-t3043).*1.02e-6).*(-1.0./2.0);
t5686 = (t3055.*(t4809+t3976.*(t2694-t2701+t3036-t3043).*1.02e-6))./2.0;
t5687 = t5572.*(t1477-t2502).*(-1.0./2.0);
t5688 = (t5572.*(t1477-t2502))./2.0;
t5690 = -t5689;
t5695 = -t5691;
t5700 = t2297.*t5639;
t5703 = t2297.*t5644;
t5707 = t4019.*t5405;
t5708 = -t5405.*(t3242-t3554);
t5710 = t4026.*t5405;
t5712 = t5405.*(t3242-t3554);
t5714 = t4031.*t5405;
t5723 = t2297.*t5666;
t5740 = t2363.*t5676.*7.26735e-3;
t5746 = t50.*t202.*t5702.*6.935255936130809e-19;
t5753 = -t5752;
t5754 = (t4772+(t3976.*(t2694-t2701+t3036-t3043))./1.0e+8).*(t1896-t3239);
t5755 = -t3547.*(t4772+(t3976.*(t2694-t2701+t3036-t3043))./1.0e+8);
t5756 = t3547.*(t4772+(t3976.*(t2694-t2701+t3036-t3043))./1.0e+8);
t5762 = t2363.*t5701.*7.26735e-3;
t5772 = -t21.*t5572.*(t1896-t3239);
t5773 = t21.*t3547.*t5572;
t5809 = t4241+t4689+t4733;
t5810 = t4457+t5408;
t5816 = t21.*t2363.*t5792;
t5826 = t3003.*t5792;
t5828 = t4019.*t5572;
t5829 = (t4809+t3976.*(t2694-t2701+t3036-t3043).*1.02e-6).*(t3242-t3554);
t5830 = -t5572.*(t3242-t3554);
t5831 = -t4026.*(t4809+t3976.*(t2694-t2701+t3036-t3043).*1.02e-6);
t5832 = t4026.*t5572;
t5833 = t5572.*(t3242-t3554);
t5834 = t4031.*t5572;
t5838 = t4491+t5431;
t5840 = -t5839;
t5844 = t3055.*t5792;
t5845 = -t5792.*(t1477-t2502);
t5846 = t5792.*(t1477-t2502).*(-1.0./2.0);
t5847 = t4650+t5414;
t5857 = t58+t59+t5855;
t5858 = t429+t5855;
t5861 = t4674+t5447;
t5867 = t3755.*t5480.*(t2694-t2701+t3036-t3043).*(-5.43845e-3);
t5868 = t3755.*t5483.*(t2694-t2701+t3036-t3043).*(-5.43845e-3);
t5871 = t3755.*t3934.*(t410-t5466).*(-5.43845e-3);
t5872 = t3755.*t3934.*(t410-t5466).*5.43845e-3;
t5873 = -t21.*t5792.*(t1896-t3239);
t5874 = t21.*t3547.*t5792;
t5875 = t21.*t5792.*(t1896-t3239);
t5877 = -t5876;
t5878 = t3810.*t5480.*(t2694-t2701+t3036-t3043).*(-5.43845e-3);
t5879 = t3810.*t5483.*(t2694-t2701+t3036-t3043).*(-5.43845e-3);
t5883 = t3810.*t3934.*(t410-t5466).*(-5.43845e-3);
t5884 = t3810.*t3934.*(t410-t5466).*5.43845e-3;
t5888 = t4872.*t5405;
t5889 = -t5405.*(t4165+t27.*(t1959-t3313+t38.*t1022.*(t855-t878).*2.196325630278387e-1));
t5890 = t5405.*(t4165+t27.*(t1959-t3313+t38.*t1022.*(t855-t878).*2.196325630278387e-1));
t5893 = t3934.*t5275.*(t1513+t1879+t2598+t2820+t2834+t3117+t3118).*(-3.633675e-3);
t5894 = t3934.*t5275.*(t1513+t1879+t2598+t2820+t2834+t3117+t3118).*3.633675e-3;
t5897 = t5313.*(t2694-t2701+t3036-t3043).*(t1513+t1879+t2598+t2820+t2834+t3117+t3118).*3.633675e-3;
t5899 = t3934.*t5317.*(t1513+t1879+t2598+t2820+t2834+t3117+t3118).*(-3.633675e-3);
t5900 = t3934.*t5317.*(t1513+t1879+t2598+t2820+t2834+t3117+t3118).*3.633675e-3;
t5905 = (t4774.*t5480)./2.0;
t5907 = (t4774.*t5483)./2.0;
t5913 = t3910.*t5369.*(t1488+t1874+t2519+t2740+t2747+t3096+t3097).*(-1.0./2.0);
t5914 = ((t410-t5466).*(t3421-t3731+t3737+t20.*t50.*t202.*(t46-t47).*8.687615694748404e-39))./2.0;
t5915 = (t3910.*t5369.*(t1488+t1874+t2519+t2740+t2747+t3096+t3097))./2.0;
t5923 = t4215.*t5466.*(t2694-t2701+t3036-t3043).*(-5.43845e-3);
t5926 = t3910.*t5373.*(t1488+t1874+t2519+t2740+t2747+t3096+t3097).*(-1.0./2.0);
t5927 = (t3910.*t5373.*(t1488+t1874+t2519+t2740+t2747+t3096+t3097))./2.0;
t5931 = -t5929;
t5934 = t3934.*t4215.*t5480.*5.43845e-3;
t5939 = t4019.*t5792;
t5940 = -t5792.*(t3242-t3554);
t5942 = t4026.*t5792;
t5943 = t5792.*(t3242-t3554);
t5945 = t4031.*t5792;
t5946 = t331+t333+t5904;
t5949 = t356+t372+t5904;
t5950 = t3712.*t5645.*(t2674-t2676+t3022-t3027).*(-1.0./2.0);
t5951 = t3712.*t5646.*(t2674-t2676+t3022-t3027).*(-1.0./2.0);
t5965 = -t5964;
t5974 = t3808.*t5645.*(t2674-t2676+t3022-t3027).*(-1.0./2.0);
t5975 = t3808.*t5646.*(t2674-t2676+t3022-t3027).*(-1.0./2.0);
t5981 = -t5980;
t5983 = t2363.*t5918;
t5984 = t2388.*t5918;
t5985 = t2419.*t5918;
t5996 = (t5024.*t5480)./2.0;
t5998 = (t5024.*t5483)./2.0;
t6001 = t5026.*(t410-t5466).*(-1.0./2.0);
t6006 = (t4711.*t5645)./2.0;
t6008 = (t4711.*t5646)./2.0;
t6017 = t4872.*t5572;
t6018 = -t5572.*(t4165+t27.*(t1959-t3313+t38.*t1022.*(t855-t878).*2.196325630278387e-1));
t6021 = t4172.*t5603.*(t2674-t2676+t3022-t3027).*(-1.0./2.0);
t6026 = (t3910.*t4172.*t5645)./2.0;
t6034 = t3543.*t5918;
t6035 = -t5918.*(t1896-t3239);
t6036 = t3547.*t5918;
t6037 = t3550.*t5918;
t6042 = (t4939.*t5645)./2.0;
t6044 = (t4939.*t5646)./2.0;
t6053 = t6052./2.0;
t6058 = t3154+t3383+t4295+t4296+t4564+t4566;
t6065 = t3160+t3445+t4298+t4305+t4585+t4620;
t6098 = t3267+t3269+t4422+t4432+t4441+t4444;
t6102 = t3265+t3272+t4433+t4439+t4442+t4449;
t6103 = t4354+t5225+t5228;
t6105 = t4151.*t5918;
t6106 = -t5918.*(t1005+t20.*(t1941-t3315+t39.*t1022.*(t855-t878).*2.196325630278387e-1));
t6109 = t4872.*t5792;
t6110 = -t5792.*(t4165+t27.*(t1959-t3313+t38.*t1022.*(t855-t878).*2.196325630278387e-1));
t6159 = t4517+t4523+t4766+t4770;
t6171 = (t5279.*t5645)./2.0;
t6174 = (t5279.*t5646)./2.0;
t6190 = t3395.*t6101;
t6220 = -t6219;
t6231 = (t5480.*t5541)./2.0;
t6233 = (t5483.*t5541)./2.0;
t6234 = t6232./2.0;
t6236 = t638+t654+t655+t657+t1576+t1579+t1584+t1585+t2291+t2311+t2671+t2683+t2684+t2696+t3029+t3233+t3288+t3307+t3531+t3597+t3609+t4053+t4054;
t6239 = t5540.*(t410-t5466).*(-1.0./2.0);
t6240 = (t5540.*(t410-t5466))./2.0;
t6245 = t3433+t3454+t4589+t4595+t4610+t4633;
t6247 = t3447+t3448+t4593+t4599+t4624+t4632;
t6248 = t3441+t3456+t4602+t4608+t4627+t4640;
t6249 = t3440+t3457+t4601+t4609+t4626+t4641;
t6260 = t3458+t3467+t4613+t4630+t4646+t4649;
